simulink model "dynamical_model_extended"  (R2017b)
settings: Solver=ode4  StartTime=0.0  StopTime=3  FixedStep=dt  RelTol=1e-3
undefined symbols (not defined in the file or in its folder): alpha0, c1, c2, c3, d0, dq_0, g, m, p_true, q_0, r
libraries: dspinverses x2
(part 2 of 3)

== matlab function dynamical_model_extended/soft robotic manipulator dynamical model/Coreoilis matrix  ==
  data: q input; y output; dq input; m parameter; r parameter
function y = fcn(q,dq,m,r)

l1 = q(1);
kappa_x1 = q(2);
kappa_y1 = q(3);

dl1 = dq(1);
dkappa_x1 = dq(2);
dkappa_y1 = dq(3);

V = zeros(3,3);

% V(1,1) = (5.0e-33*dl1*m*(400000000000000000000000000000000.0*kappa_x1^2*sin(l1*(kappa_x1^2 + kappa_y1^2)^(1/2)) + 133333333333333333333333333333333.0*kappa_y1^2*l1^3*(kappa_x1^2 + kappa_y1^2)^(3/2) - 400000000000000000000000000000000.0*kappa_x1^2*l1*cos(l1*(kappa_x1^2 + kappa_y1^2)^(1/2))*(kappa_x1^2 + kappa_y1^2)^(1/2)))/(l1^2*(kappa_x1^2 + kappa_y1^2)^(5/2)) - (5.0e-33*dkappa_y1*kappa_y1*m*(266666666666666666666666666666677.0*kappa_y1^4*l1^3*(kappa_x1^2 + kappa_y1^2)^(3/2) - 133333333333333333333333333333333.0*kappa_x1^2*l1^3*(kappa_x1^2 + kappa_y1^2)^(5/2) - 266666666666666666666666666666677.0*kappa_y1^2*l1^3*(kappa_x1^2 + kappa_y1^2)^(5/2) - 2.0e33*kappa_x1^4*sin(l1*(kappa_x1^2 + kappa_y1^2)^(1/2)) - 2.0e33*kappa_x1^2*kappa_y1^2*sin(l1*(kappa_x1^2 + kappa_y1^2)^(1/2)) + 400000000000000000000000000000000.0*kappa_x1^2*l1*(kappa_x1^2 + kappa_y1^2)^(3/2) + 1.2e33*kappa_x1^4*l1*(kappa_x1^2 + kappa_y1^2)^(1/2) + 266666666666666666666666666666677.0*kappa_x1^2*kappa_y1^2*l1^3*(kappa_x1^2 + kappa_y1^2)^(3/2) + 400000000000000000000000000000000.0*kappa_x1^4*l1*cos(l1*(kappa_x1^2 + kappa_y1^2)^(1/2))*(kappa_x1^2 + kappa_y1^2)^(1/2) + 1.2e33*kappa_x1^2*kappa_y1^2*l1*(kappa_x1^2 + kappa_y1^2)^(1/2) + 400000000000000000000000000000000.0*kappa_x1^2*kappa_y1^2*l1*cos(l1*(kappa_x1^2 + kappa_y1^2)^(1/2))*(kappa_x1^2 + kappa_y1^2)^(1/2)))/(l1*(kappa_x1^2 + kappa_y1^2)^(9/2)) - (5.0e-33*dkappa_x1*kappa_x1*m*(800000000000000000000000000000000.0*kappa_y1^4*sin(l1*(kappa_x1^2 + kappa_y1^2)^(1/2)) - 1.2e33*kappa_x1^4*sin(l1*(kappa_x1^2 + kappa_y1^2)^(1/2)) - 400000000000000000000000000000000.0*l1*(kappa_x1^2 + kappa_y1^2)^(5/2) - 133333333333333333333333333333333.0*kappa_y1^2*l1^3*(kappa_x1^2 + kappa_y1^2)^(5/2) + 266666666666666666666666666666677.0*kappa_y1^4*l1^3*(kappa_x1^2 + kappa_y1^2)^(3/2) - 400000000000000000000000000000000.0*kappa_x1^2*kappa_y1^2*sin(l1*(kappa_x1^2 + kappa_y1^2)^(1/2)) + 1.2e33*kappa_x1^4*l1*(kappa_x1^2 + kappa_y1^2)^(1/2) - 400000000000000000000000000000000.0*kappa_y1^2*l1*(kappa_x1^2 + kappa_y1^2)^(3/2) + 266666666666666666666666666666677.0*kappa_x1^2*kappa_y1^2*l1^3*(kappa_x1^2 + kappa_y1^2)^(3/2) + 400000000000000000000000000000000.0*kappa_x1^4*l1*cos(l1*(kappa_x1^2 + kappa_y1^2)^(1/2))*(kappa_x1^2 + kappa_y1^2)^(1/2) + 1.2e33*kappa_x1^2*kappa_y1^2*l1*(kappa_x1^2 + kappa_y1^2)^(1/2) + 400000000000000000000000000000000.0*kappa_x1^2*kappa_y1^2*l1*cos(l1*(kappa_x1^2 + kappa_y1^2)^(1/2))*(kappa_x1^2 + kappa_y1^2)^(1/2)))/(l1*(kappa_x1^2 + kappa_y1^2)^(9/2));
% V(1,2) = - (dkappa_x1*(6.4e34*l1*m*(kappa_x1^2 + kappa_y1^2)^(3/2) - 1.6e34*l1^3*m*(kappa_x1^2 + kappa_y1^2)^(5/2) - 6.4e34*l1*m*cos(l1*(kappa_x1^2 + kappa_y1^2)^(1/2))*(kappa_x1^2 + kappa_y1^2)^(3/2) + 1.6e34*l1^2*m*sin(l1*(kappa_x1^2 + kappa_y1^2)^(1/2))*(kappa_x1^2 + kappa_y1^2)^2 + 3.2e34*kappa_x1^2*l1^3*m*(kappa_x1^2 + kappa_y1^2)^(3/2) + 3.2e34*kappa_y1^2*l1^3*m*(kappa_x1^2 + kappa_y1^2)^(3/2) + 5.3333333333333333333333333333333e33*kappa_x1^6*l1^3*m*((kappa_x1^2 + kappa_y1^2)/kappa_x1^2)^(1/2) + 1.6e34*kappa_x1^2*l1^3*m*cos(l1*(kappa_x1^2 + kappa_y1^2)^(1/2))*(kappa_x1^2 + kappa_y1^2)^(3/2) + 1.6e34*kappa_y1^2*l1^3*m*cos(l1*(kappa_x1^2 + kappa_y1^2)^(1/2))*(kappa_x1^2 + kappa_y1^2)^(3/2) - 2.0e33*kappa_y1^2*m*sin(2.0*l1*(kappa_x1^2 + kappa_y1^2)^(1/2))*((kappa_x1^2 + kappa_y1^2)/kappa_x1^2)^(1/2)*(kappa_x1^2 + kappa_y1^2)^(1/2) + 5.3333333333333333333333333333333e33*kappa_x1^2*kappa_y1^4*l1^3*m*((kappa_x1^2 + kappa_y1^2)/kappa_x1^2)^(1/2) + 1.0666666666666666666666666666667e34*kappa_x1^4*kappa_y1^2*l1^3*m*((kappa_x1^2 + kappa_y1^2)/kappa_x1^2)^(1/2) + 1.3333333333333333333333333333333e33*kappa_x1^8*l1^3*m*r^2*((kappa_x1^2 + kappa_y1^2)/kappa_x1^2)^(1/2) - 8.0e34*kappa_x1^2*l1^2*m*sin(l1*(kappa_x1^2 + kappa_y1^2)^(1/2))*(kappa_x1^2 + kappa_y1^2) - 8.0e34*kappa_y1^2*l1^2*m*sin(l1*(kappa_x1^2 + kappa_y1^2)^(1/2))*(kappa_x1^2 + kappa_y1^2) + 3.2e34*kappa_x1^2*m*sin(l1*(kappa_x1^2 + kappa_y1^2)^(1/2))*((kappa_x1^2 + kappa_y1^2)/kappa_x1^2)^(1/2)*(kappa_x1^2 + kappa_y1^2)^(1/2) + 1.6e34*kappa_y1^2*m*sin(l1*(kappa_x1^2 + kappa_y1^2)^(1/2))*((kappa_x1^2 + kappa_y1^2)/kappa_x1^2)^(1/2)*(kappa_x1^2 + kappa_y1^2)^(1/2) - 1.0e33*kappa_y1^2*m*r^2*sin(2.0*l1*(kappa_x1^2 + kappa_y1^2)^(1/2))*((kappa_x1^2 + kappa_y1^2)/kappa_x1^2)^(1/2)*(kappa_x1^2 + kappa_y1^2)^(3/2) + 500000000000000000000000000000000.0*kappa_y1^4*m*r^2*sin(2.0*l1*(kappa_x1^2 + kappa_y1^2)^(1/2))*((kappa_x1^2 + kappa_y1^2)/kappa_x1^2)^(1/2)*(kappa_x1^2 + kappa_y1^2)^(1/2) + 4.0e33*kappa_y1^2*l1*m*cos(2.0*l1*(kappa_x1^2 + kappa_y1^2)^(1/2))*((kappa_x1^2 + kappa_y1^2)/kappa_x1^2)^(1/2)*(kappa_x1^2 + kappa_y1^2) + 2.6666666666666666666666666666667e33*kappa_x1^2*kappa_y1^6*l1^3*m*r^2*((kappa_x1^2 + kappa_y1^2)/kappa_x1^2)^(1/2) + 6.6666666666666666666666666666667e33*kappa_x1^4*kappa_y1^4*l1^3*m*r^2*((kappa_x1^2 + kappa_y1^2)/kappa_x1^2)^(1/2) + 5.3333333333333333333333333333333e33*kappa_x1^6*kappa_y1^2*l1^3*m*r^2*((kappa_x1^2 + kappa_y1^2)/kappa_x1^2)^(1/2) - 1.6e34*kappa_x1^4*l1^2*m*sin(l1*(kappa_x1^2 + kappa_y1^2)^(1/2))*((kappa_x1^2 + kappa_y1^2)/kappa_x1^2)^(1/2)*(kappa_x1^2 + kappa_y1^2)^(1/2) + 8.0e33*kappa_y1^2*m*r^2*sin(l1*(kappa_x1^2 + kappa_y1^2)^(1/2))*((kappa_x1^2 + kappa_y1^2)/kappa_x1^2)^(1/2)*(kappa_x1^2 + kappa_y1^2)^(3/2) - 3.2e34*kappa_x1^2*l1*m*cos(l1*(kappa_x1^2 + kappa_y1^2)^(1/2))*((kappa_x1^2 + kappa_y1^2)/kappa_x1^2)^(1/2)*(kappa_x1^2 + kappa_y1^2) - 1.6e34*kappa_y1^2*l1*m*cos(l1*(kappa_x1^2 + kappa_y1^2)^(1/2))*((kappa_x1^2 + kappa_y1^2)/kappa_x1^2)^(1/2)*(kappa_x1^2 + kappa_y1^2) - 1.0e33*kappa_y1^4*l1*m*r^2*cos(2.0*l1*(kappa_x1^2 + kappa_y1^2)^(1/2))*((kappa_x1^2 + kappa_y1^2)/kappa_x1^2)^(1/2)*(kappa_x1^2 + kappa_y1^2) - 8.0e33*kappa_y1^2*l1*m*r^2*cos(l1*(kappa_x1^2 + kappa_y1^2)^(1/2))*((kappa_x1^2 + kappa_y1^2)/kappa_x1^2)^(1/2)*(kappa_x1^2 + kappa_y1^2)^2 + 2.0e33*kappa_y1^2*l1*m*r^2*cos(2.0*l1*(kappa_x1^2 + kappa_y1^2)^(1/2))*((kappa_x1^2 + kappa_y1^2)/kappa_x1^2)^(1/2)*(kappa_x1^2 + kappa_y1^2)^2 - 1.6e34*kappa_x1^2*kappa_y1^2*l1^2*m*sin(l1*(kappa_x1^2 + kappa_y1^2)^(1/2))*((kappa_x1^2 + kappa_y1^2)/kappa_x1^2)^(1/2)*(kappa_x1^2 + kappa_y1^2)^(1/2) + 4.0e33*kappa_x1^2*kappa_y1^2*m*r^2*sin(l1*(kappa_x1^2 + kappa_y1^2)^(1/2))*((kappa_x1^2 + kappa_y1^2)/kappa_x1^2)^(1/2)*(kappa_x1^2 + kappa_y1^2)^(1/2) + 1.0e33*kappa_x1^2*kappa_y1^2*m*r^2*sin(2.0*l1*(kappa_x1^2 + kappa_y1^2)^(1/2))*((kappa_x1^2 + kappa_y1^2)/kappa_x1^2)^(1/2)*(kappa_x1^2 + kappa_y1^2)^(1/2) - 4.0e33*kappa_x1^2*kappa_y1^4*l1^2*m*r^2*sin(l1*(kappa_x1^2 + kappa_y1^2)^(1/2))*((kappa_x1^2 + kappa_y1^2)/kappa_x1^2)^(1/2)*(kappa_x1^2 + kappa_y1^2)^(1/2) - 4.0e33*kappa_x1^4*kappa_y1^2*l1^2*m*r^2*sin(l1*(kappa_x1^2 + kappa_y1^2)^(1/2))*((kappa_x1^2 + kappa_y1^2)/kappa_x1^2)^(1/2)*(kappa_x1^2 + kappa_y1^2)^(1/2) - 4.0e33*kappa_x1^2*kappa_y1^2*l1*m*r^2*cos(l1*(kappa_x1^2 + kappa_y1^2)^(1/2))*((kappa_x1^2 + kappa_y1^2)/kappa_x1^2)^(1/2)*(kappa_x1^2 + kappa_y1^2) - 2.0e33*kappa_x1^2*kappa_y1^2*l1*m*r^2*cos(2.0*l1*(kappa_x1^2 + kappa_y1^2)^(1/2))*((kappa_x1^2 + kappa_y1^2)/kappa_x1^2)^(1/2)*(kappa_x1^2 + kappa_y1^2)))/(8000000000000000000000000000000000*l1^2*((kappa_x1^2 + kappa_y1^2)/kappa_x1^2)^(1/2)*(kappa_x1^2 + kappa_y1^2)^4) - (dkappa_y1*(4.0e33*kappa_y1^3*l1^3*m*(kappa_x1^2 + kappa_y1^2)^(3/2) - 2.0e33*kappa_y1*l1^3*m*(kappa_x1^2 + kappa_y1^2)^(5/2) + 8.0e33*kappa_y1*l1*m*(kappa_x1^2 + kappa_y1^2)^(3/2) + 4.0e33*kappa_x1^2*kappa_y1*l1^3*m*(kappa_x1^2 + kappa_y1^2)^(3/2) + 2.0e33*kappa_y1^3*l1^3*m*cos(l1*(kappa_x1^2 + kappa_y1^2)^(1/2))*(kappa_x1^2 + kappa_y1^2)^(3/2) + 1.3333333333333333333333333333333e33*kappa_x1^6*kappa_y1*l1^3*m*((kappa_x1^2 + kappa_y1^2)/kappa_x1^2)^(1/2) - 8.0e33*kappa_y1*l1*m*cos(l1*(kappa_x1^2 + kappa_y1^2)^(1/2))*(kappa_x1^2 + kappa_y1^2)^(3/2) + 1.3333333333333333333333333333333e33*kappa_x1^2*kappa_y1^5*l1^3*m*((kappa_x1^2 + kappa_y1^2)/kappa_x1^2)^(1/2) + 2.6666666666666666666666666666667e33*kappa_x1^4*kappa_y1^3*l1^3*m*((kappa_x1^2 + kappa_y1^2)/kappa_x1^2)^(1/2) + 2.0e33*kappa_y1*l1^2*m*sin(l1*(kappa_x1^2 + kappa_y1^2)^(1/2))*(kappa_x1^2 + kappa_y1^2)^2 - 1.0e34*kappa_y1^3*l1^2*m*sin(l1*(kappa_x1^2 + kappa_y1^2)^(1/2))*(kappa_x1^2 + kappa_y1^2) + 333333333333333333333333333333333.0*kappa_x1^8*kappa_y1*l1^3*m*r^2*((kappa_x1^2 + kappa_y1^2)/kappa_x1^2)^(1/2) - 1.0e34*kappa_x1^2*kappa_y1*l1^2*m*sin(l1*(kappa_x1^2 + kappa_y1^2)^(1/2))*(kappa_x1^2 + kappa_y1^2) + 4.0e33*kappa_x1^2*kappa_y1*m*sin(l1*(kappa_x1^2 + kappa_y1^2)^(1/2))*((kappa_x1^2 + kappa_y1^2)/kappa_x1^2)^(1/2)*(kappa_x1^2 + kappa_y1^2)^(1/2) + 666666666666666666666666666666677.0*kappa_x1^2*kappa_y1^7*l1^3*m*r^2*((kappa_x1^2 + kappa_y1^2)/kappa_x1^2)^(1/2) + 1.6666666666666666666666666666667e33*kappa_x1^4*kappa_y1^5*l1^3*m*r^2*((kappa_x1^2 + kappa_y1^2)/kappa_x1^2)^(1/2) + 1.3333333333333333333333333333333e33*kappa_x1^6*kappa_y1^3*l1^3*m*r^2*((kappa_x1^2 + kappa_y1^2)/kappa_x1^2)^(1/2) + 2.0e33*kappa_x1^2*kappa_y1*l1^3*m*cos(l1*(kappa_x1^2 + kappa_y1^2)^(1/2))*(kappa_x1^2 + kappa_y1^2)^(3/2) + 500000000000000000000000000000000.0*kappa_x1^2*kappa_y1*m*sin(2.0*l1*(kappa_x1^2 + kappa_y1^2)^(1/2))*((kappa_x1^2 + kappa_y1^2)/kappa_x1^2)^(1/2)*(kappa_x1^2 + kappa_y1^2)^(1/2) - 4.0e33*kappa_x1^4*kappa_y1*l1^2*m*sin(l1*(kappa_x1^2 + kappa_y1^2)^(1/2))*((kappa_x1^2 + kappa_y1^2)/kappa_x1^2)^(1/2)*(kappa_x1^2 + kappa_y1^2)^(1/2) - 2.0e33*kappa_x1^2*kappa_y1*m*r^2*sin(l1*(kappa_x1^2 + kappa_y1^2)^(1/2))*((kappa_x1^2 + kappa_y1^2)/kappa_x1^2)^(1/2)*(kappa_x1^2 + kappa_y1^2)^(3/2) - 500000000000000000000000000000000.0*kappa_x1^4*kappa_y1*m*r^2*sin(l1*(kappa_x1^2 + kappa_y1^2)^(1/2))*((kappa_x1^2 + kappa_y1^2)/kappa_x1^2)^(1/2)*(kappa_x1^2 + kappa_y1^2)^(1/2) - 4.0e33*kappa_x1^2*kappa_y1*l1*m*cos(l1*(kappa_x1^2 + kappa_y1^2)^(1/2))*((kappa_x1^2 + kappa_y1^2)/kappa_x1^2)^(1/2)*(kappa_x1^2 + kappa_y1^2) + 250000000000000000000000000000000.0*kappa_x1^2*kappa_y1*m*r^2*sin(2.0*l1*(kappa_x1^2 + kappa_y1^2)^(1/2))*((kappa_x1^2 + kappa_y1^2)/kappa_x1^2)^(1/2)*(kappa_x1^2 + kappa_y1^2)^(3/2) - 250000000000000000000000000000000.0*kappa_x1^4*kappa_y1*m*r^2*sin(2.0*l1*(kappa_x1^2 + kappa_y1^2)^(1/2))*((kappa_x1^2 + kappa_y1^2)/kappa_x1^2)^(1/2)*(kappa_x1^2 + kappa_y1^2)^(1/2) - 4.0e33*kappa_x1^2*kappa_y1^3*l1^2*m*sin(l1*(kappa_x1^2 + kappa_y1^2)^(1/2))*((kappa_x1^2 + kappa_y1^2)/kappa_x1^2)^(1/2)*(kappa_x1^2 + kappa_y1^2)^(1/2) + 500000000000000000000000000000000.0*kappa_x1^2*kappa_y1^3*m*r^2*sin(l1*(kappa_x1^2 + kappa_y1^2)^(1/2))*((kappa_x1^2 + kappa_y1^2)/kappa_x1^2)^(1/2)*(kappa_x1^2 + kappa_y1^2)^(1/2) - 1.0e33*kappa_x1^2*kappa_y1*l1*m*cos(2.0*l1*(kappa_x1^2 + kappa_y1^2)^(1/2))*((kappa_x1^2 + kappa_y1^2)/kappa_x1^2)^(1/2)*(kappa_x1^2 + kappa_y1^2) - 125000000000000000000000000000000.0*kappa_x1^2*kappa_y1^3*m*r^2*sin(2.0*l1*(kappa_x1^2 + kappa_y1^2)^(1/2))*((kappa_x1^2 + kappa_y1^2)/kappa_x1^2)^(1/2)*(kappa_x1^2 + kappa_y1^2)^(1/2) + 500000000000000000000000000000000.0*kappa_x1^6*kappa_y1*l1^2*m*r^2*sin(l1*(kappa_x1^2 + kappa_y1^2)^(1/2))*((kappa_x1^2 + kappa_y1^2)/kappa_x1^2)^(1/2)*(kappa_x1^2 + kappa_y1^2)^(1/2) + 500000000000000000000000000000000.0*kappa_x1^4*kappa_y1*l1*m*r^2*cos(l1*(kappa_x1^2 + kappa_y1^2)^(1/2))*((kappa_x1^2 + kappa_y1^2)/kappa_x1^2)^(1/2)*(kappa_x1^2 + kappa_y1^2) - 500000000000000000000000000000000.0*kappa_x1^2*kappa_y1^5*l1^2*m*r^2*sin(l1*(kappa_x1^2 + kappa_y1^2)^(1/2))*((kappa_x1^2 + kappa_y1^2)/kappa_x1^2)^(1/2)*(kappa_x1^2 + kappa_y1^2)^(1/2) + 500000000000000000000000000000000.0*kappa_x1^4*kappa_y1*l1*m*r^2*cos(2.0*l1*(kappa_x1^2 + kappa_y1^2)^(1/2))*((kappa_x1^2 + kappa_y1^2)/kappa_x1^2)^(1/2)*(kappa_x1^2 + kappa_y1^2) + 2.0e33*kappa_x1^2*kappa_y1*l1*m*r^2*cos(l1*(kappa_x1^2 + kappa_y1^2)^(1/2))*((kappa_x1^2 + kappa_y1^2)/kappa_x1^2)^(1/2)*(kappa_x1^2 + kappa_y1^2)^2 - 500000000000000000000000000000000.0*kappa_x1^2*kappa_y1^3*l1*m*r^2*cos(l1*(kappa_x1^2 + kappa_y1^2)^(1/2))*((kappa_x1^2 + kappa_y1^2)/kappa_x1^2)^(1/2)*(kappa_x1^2 + kappa_y1^2) - 500000000000000000000000000000000.0*kappa_x1^2*kappa_y1*l1*m*r^2*cos(2.0*l1*(kappa_x1^2 + kappa_y1^2)^(1/2))*((kappa_x1^2 + kappa_y1^2)/kappa_x1^2)^(1/2)*(kappa_x1^2 + kappa_y1^2)^2 + 250000000000000000000000000000000.0*kappa_x1^2*kappa_y1^3*l1*m*r^2*cos(2.0*l1*(kappa_x1^2 + kappa_y1^2)^(1/2))*((kappa_x1^2 + kappa_y1^2)/kappa_x1^2)^(1/2)*(kappa_x1^2 + kappa_y1^2)))/(2000000000000000000000000000000000*kappa_x1*l1^2*((kappa_x1^2 + kappa_y1^2)/kappa_x1^2)^(1/2)*(kappa_x1^2 + kappa_y1^2)^4) - (5.0e-33*dl1*kappa_x1*m*(800000000000000000000000000000000.0*kappa_y1^4*sin(l1*(kappa_x1^2 + kappa_y1^2)^(1/2)) - 1.2e33*kappa_x1^4*sin(l1*(kappa_x1^2 + kappa_y1^2)^(1/2)) - 400000000000000000000000000000000.0*l1*(kappa_x1^2 + kappa_y1^2)^(5/2) - 133333333333333333333333333333333.0*kappa_y1^2*l1^3*(kappa_x1^2 + kappa_y1^2)^(5/2) + 266666666666666666666666666666677.0*kappa_y1^4*l1^3*(kappa_x1^2 + kappa_y1^2)^(3/2) - 400000000000000000000000000000000.0*kappa_x1^2*kappa_y1^2*sin(l1*(kappa_x1^2 + kappa_y1^2)^(1/2)) + 1.2e33*kappa_x1^4*l1*(kappa_x1^2 + kappa_y1^2)^(1/2) - 400000000000000000000000000000000.0*kappa_y1^2*l1*(kappa_x1^2 + kappa_y1^2)^(3/2) + 266666666666666666666666666666677.0*kappa_x1^2*kappa_y1^2*l1^3*(kappa_x1^2 + kappa_y1^2)^(3/2) + 400000000000000000000000000000000.0*kappa_x1^4*l1*cos(l1*(kappa_x1^2 + kappa_y1^2)^(1/2))*(kappa_x1^2 + kappa_y1^2)^(1/2) + 1.2e33*kappa_x1^2*kappa_y1^2*l1*(kappa_x1^2 + kappa_y1^2)^(1/2) + 400000000000000000000000000000000.0*kappa_x1^2*kappa_y1^2*l1*cos(l1*(kappa_x1^2 + kappa_y1^2)^(1/2))*(kappa_x1^2 + kappa_y1^2)^(1/2)))/(l1*(kappa_x1^2 + kappa_y1^2)^(9/2));
% V(1,3) = - (dkappa_y1*(5.3333333333333333333333333333333e33*kappa_y1^6*l1^3*m + 1.0666666666666666666666666666667e34*kappa_x1^2*kappa_y1^4*l1^3*m + 5.3333333333333333333333333333333e33*kappa_x1^4*kappa_y1^2*l1^3*m + 2.6666666666666666666666666666667e33*kappa_y1^8*l1^3*m*r^2 + 1.6e34*kappa_x1^2*m*sin(l1*(kappa_x1^2 + kappa_y1^2)^(1/2))*(kappa_x1^2 + kappa_y1^2)^(1/2) + 3.2e34*kappa_y1^2*m*sin(l1*(kappa_x1^2 + kappa_y1^2)^(1/2))*(kappa_x1^2 + kappa_y1^2)^(1/2) - 2.0e33*kappa_x1^2*m*sin(2.0*l1*(kappa_x1^2 + kappa_y1^2)^(1/2))*(kappa_x1^2 + kappa_y1^2)^(1/2) - 1.6e34*kappa_y1^4*l1^2*m*sin(l1*(kappa_x1^2 + kappa_y1^2)^(1/2))*(kappa_x1^2 + kappa_y1^2)^(1/2) + 8.0e33*kappa_x1^2*m*r^2*sin(l1*(kappa_x1^2 + kappa_y1^2)^(1/2))*(kappa_x1^2 + kappa_y1^2)^(3/2) - 1.6e34*kappa_x1^2*l1*m*cos(l1*(kappa_x1^2 + kappa_y1^2)^(1/2))*(kappa_x1^2 + kappa_y1^2) - 3.2e34*kappa_y1^2*l1*m*cos(l1*(kappa_x1^2 + kappa_y1^2)^(1/2))*(kappa_x1^2 + kappa_y1^2) - 1.0e33*kappa_x1^2*m*r^2*sin(2.0*l1*(kappa_x1^2 + kappa_y1^2)^(1/2))*(kappa_x1^2 + kappa_y1^2)^(3/2) + 1.0e33*kappa_x1^4*m*r^2*sin(2.0*l1*(kappa_x1^2 + kappa_y1^2)^(1/2))*(kappa_x1^2 + kappa_y1^2)^(1/2) + 4.0e33*kappa_x1^2*l1*m*cos(2.0*l1*(kappa_x1^2 + kappa_y1^2)^(1/2))*(kappa_x1^2 + kappa_y1^2) + 6.6666666666666666666666666666667e33*kappa_x1^2*kappa_y1^6*l1^3*m*r^2 + 5.3333333333333333333333333333333e33*kappa_x1^4*kappa_y1^4*l1^3*m*r^2 + 1.3333333333333333333333333333333e33*kappa_x1^6*kappa_y1^2*l1^3*m*r^2 - 1.6e34*kappa_x1^2*kappa_y1^2*l1^2*m*sin(l1*(kappa_x1^2 + kappa_y1^2)^(1/2))*(kappa_x1^2 + kappa_y1^2)^(1/2) - 4.0e33*kappa_x1^2*kappa_y1^2*m*r^2*sin(l1*(kappa_x1^2 + kappa_y1^2)^(1/2))*(kappa_x1^2 + kappa_y1^2)^(1/2) + 500000000000000000000000000000000.0*kappa_x1^2*kappa_y1^2*m*r^2*sin(2.0*l1*(kappa_x1^2 + kappa_y1^2)^(1/2))*(kappa_x1^2 + kappa_y1^2)^(1/2) - 2.0e33*kappa_x1^4*l1*m*r^2*cos(2.0*l1*(kappa_x1^2 + kappa_y1^2)^(1/2))*(kappa_x1^2 + kappa_y1^2) - 8.0e33*kappa_x1^2*l1*m*r^2*cos(l1*(kappa_x1^2 + kappa_y1^2)^(1/2))*(kappa_x1^2 + kappa_y1^2)^2 + 2.0e33*kappa_x1^2*l1*m*r^2*cos(2.0*l1*(kappa_x1^2 + kappa_y1^2)^(1/2))*(kappa_x1^2 + kappa_y1^2)^2 + 4.0e33*kappa_x1^2*kappa_y1^2*l1*m*r^2*cos(l1*(kappa_x1^2 + kappa_y1^2)^(1/2))*(kappa_x1^2 + kappa_y1^2) - 1.0e33*kappa_x1^2*kappa_y1^2*l1*m*r^2*cos(2.0*l1*(kappa_x1^2 + kappa_y1^2)^(1/2))*(kappa_x1^2 + kappa_y1^2) + 4.0e33*kappa_x1^2*kappa_y1^4*l1^2*m*r^2*sin(l1*(kappa_x1^2 + kappa_y1^2)^(1/2))*(kappa_x1^2 + kappa_y1^2)^(1/2) + 4.0e33*kappa_x1^4*kappa_y1^2*l1^2*m*r^2*sin(l1*(kappa_x1^2 + kappa_y1^2)^(1/2))*(kappa_x1^2 + kappa_y1^2)^(1/2)))/(8000000000000000000000000000000000*l1^2*(kappa_x1^2 + kappa_y1^2)^4) - (5.0e-33*dl1*kappa_y1*m*(266666666666666666666666666666677.0*kappa_y1^4*l1^3*(kappa_x1^2 + kappa_y1^2)^(3/2) - 133333333333333333333333333333333.0*kappa_x1^2*l1^3*(kappa_x1^2 + kappa_y1^2)^(5/2) - 266666666666666666666666666666677.0*kappa_y1^2*l1^3*(kappa_x1^2 + kappa_y1^2)^(5/2) - 2.0e33*kappa_x1^4*sin(l1*(kappa_x1^2 + kappa_y1^2)^(1/2)) - 2.0e33*kappa_x1^2*kappa_y1^2*sin(l1*(kappa_x1^2 + kappa_y1^2)^(1/2)) + 400000000000000000000000000000000.0*kappa_x1^2*l1*(kappa_x1^2 + kappa_y1^2)^(3/2) + 1.2e33*kappa_x1^4*l1*(kappa_x1^2 + kappa_y1^2)^(1/2) + 266666666666666666666666666666677.0*kappa_x1^2*kappa_y1^2*l1^3*(kappa_x1^2 + kappa_y1^2)^(3/2) + 400000000000000000000000000000000.0*kappa_x1^4*l1*cos(l1*(kappa_x1^2 + kappa_y1^2)^(1/2))*(kappa_x1^2 + kappa_y1^2)^(1/2) + 1.2e33*kappa_x1^2*kappa_y1^2*l1*(kappa_x1^2 + kappa_y1^2)^(1/2) + 400000000000000000000000000000000.0*kappa_x1^2*kappa_y1^2*l1*cos(l1*(kappa_x1^2 + kappa_y1^2)^(1/2))*(kappa_x1^2 + kappa_y1^2)^(1/2)))/(l1*(kappa_x1^2 + kappa_y1^2)^(9/2)) - (dkappa_x1*(4.0e33*kappa_y1^3*l1^3*m*(kappa_x1^2 + kappa_y1^2)^(3/2) - 2.0e33*kappa_y1*l1^3*m*(kappa_x1^2 + kappa_y1^2)^(5/2) + 8.0e33*kappa_y1*l1*m*(kappa_x1^2 + kappa_y1^2)^(3/2) + 4.0e33*kappa_x1^2*kappa_y1*l1^3*m*(kappa_x1^2 + kappa_y1^2)^(3/2) + 2.0e33*kappa_y1^3*l1^3*m*cos(l1*(kappa_x1^2 + kappa_y1^2)^(1/2))*(kappa_x1^2 + kappa_y1^2)^(3/2) + 1.3333333333333333333333333333333e33*kappa_x1^6*kappa_y1*l1^3*m*((kappa_x1^2 + kappa_y1^2)/kappa_x1^2)^(1/2) - 8.0e33*kappa_y1*l1*m*cos(l1*(kappa_x1^2 + kappa_y1^2)^(1/2))*(kappa_x1^2 + kappa_y1^2)^(3/2) + 1.3333333333333333333333333333333e33*kappa_x1^2*kappa_y1^5*l1^3*m*((kappa_x1^2 + kappa_y1^2)/kappa_x1^2)^(1/2) + 2.6666666666666666666666666666667e33*kappa_x1^4*kappa_y1^3*l1^3*m*((kappa_x1^2 + kappa_y1^2)/kappa_x1^2)^(1/2) + 2.0e33*kappa_y1*l1^2*m*sin(l1*(kappa_x1^2 + kappa_y1^2)^(1/2))*(kappa_x1^2 + kappa_y1^2)^2 - 1.0e34*kappa_y1^3*l1^2*m*sin(l1*(kappa_x1^2 + kappa_y1^2)^(1/2))*(kappa_x1^2 + kappa_y1^2) + 333333333333333333333333333333333.0*kappa_x1^8*kappa_y1*l1^3*m*r^2*((kappa_x1^2 + kappa_y1^2)/kappa_x1^2)^(1/2) - 1.0e34*kappa_x1^2*kappa_y1*l1^2*m*sin(l1*(kappa_x1^2 + kappa_y1^2)^(1/2))*(kappa_x1^2 + kappa_y1^2) + 4.0e33*kappa_x1^2*kappa_y1*m*sin(l1*(kappa_x1^2 + kappa_y1^2)^(1/2))*((kappa_x1^2 + kappa_y1^2)/kappa_x1^2)^(1/2)*(kappa_x1^2 + kappa_y1^2)^(1/2) + 666666666666666666666666666666677.0*kappa_x1^2*kappa_y1^7*l1^3*m*r^2*((kappa_x1^2 + kappa_y1^2)/kappa_x1^2)^(1/2) + 1.6666666666666666666666666666667e33*kappa_x1^4*kappa_y1^5*l1^3*m*r^2*((kappa_x1^2 + kappa_y1^2)/kappa_x1^2)^(1/2) + 1.3333333333333333333333333333333e33*kappa_x1^6*kappa_y1^3*l1^3*m*r^2*((kappa_x1^2 + kappa_y1^2)/kappa_x1^2)^(1/2) + 2.0e33*kappa_x1^2*kappa_y1*l1^3*m*cos(l1*(kappa_x1^2 + kappa_y1^2)^(1/2))*(kappa_x1^2 + kappa_y1^2)^(3/2) + 500000000000000000000000000000000.0*kappa_x1^2*kappa_y1*m*sin(2.0*l1*(kappa_x1^2 + kappa_y1^2)^(1/2))*((kappa_x1^2 + kappa_y1^2)/kappa_x1^2)^(1/2)*(kappa_x1^2 + kappa_y1^2)^(1/2) - 4.0e33*kappa_x1^4*kappa_y1*l1^2*m*sin(l1*(kappa_x1^2 + kappa_y1^2)^(1/2))*((kappa_x1^2 + kappa_y1^2)/kappa_x1^2)^(1/2)*(kappa_x1^2 + kappa_y1^2)^(1/2) - 2.0e33*kappa_x1^2*kappa_y1*m*r^2*sin(l1*(kappa_x1^2 + kappa_y1^2)^(1/2))*((kappa_x1^2 + kappa_y1^2)/kappa_x1^2)^(1/2)*(kappa_x1^2 + kappa_y1^2)^(3/2) - 500000000000000000000000000000000.0*kappa_x1^4*kappa_y1*m*r^2*sin(l1*(kappa_x1^2 + kappa_y1^2)^(1/2))*((kappa_x1^2 + kappa_y1^2)/kappa_x1^2)^(1/2)*(kappa_x1^2 + kappa_y1^2)^(1/2) - 4.0e33*kappa_x1^2*kappa_y1*l1*m*cos(l1*(kappa_x1^2 + kappa_y1^2)^(1/2))*((kappa_x1^2 + kappa_y1^2)/kappa_x1^2)^(1/2)*(kappa_x1^2 + kappa_y1^2) + 250000000000000000000000000000000.0*kappa_x1^2*kappa_y1*m*r^2*sin(2.0*l1*(kappa_x1^2 + kappa_y1^2)^(1/2))*((kappa_x1^2 + kappa_y1^2)/kappa_x1^2)^(1/2)*(kappa_x1^2 + kappa_y1^2)^(3/2) - 250000000000000000000000000000000.0*kappa_x1^4*kappa_y1*m*r^2*sin(2.0*l1*(kappa_x1^2 + kappa_y1^2)^(1/2))*((kappa_x1^2 + kappa_y1^2)/kappa_x1^2)^(1/2)*(kappa_x1^2 + kappa_y1^2)^(1/2) - 4.0e33*kappa_x1^2*kappa_y1^3*l1^2*m*sin(l1*(kappa_x1^2 + kappa_y1^2)^(1/2))*((kappa_x1^2 + kappa_y1^2)/kappa_x1^2)^(1/2)*(kappa_x1^2 + kappa_y1^2)^(1/2) + 500000000000000000000000000000000.0*kappa_x1^2*kappa_y1^3*m*r^2*sin(l1*(kappa_x1^2 + kappa_y1^2)^(1/2))*((kappa_x1^2 + kappa_y1^2)/kappa_x1^2)^(1/2)*(kappa_x1^2 + kappa_y1^2)^(1/2) - 1.0e33*kappa_x1^2*kappa_y1*l1*m*cos(2.0*l1*(kappa_x1^2 + kappa_y1^2)^(1/2))*((kappa_x1^2 + kappa_y1^2)/kappa_x1^2)^(1/2)*(kappa_x1^2 + kappa_y1^2) - 125000000000000000000000000000000.0*kappa_x1^2*kappa_y1^3*m*r^2*sin(2.0*l1*(kappa_x1^2 + kappa_y1^2)^(1/2))*((kappa_x1^2 + kappa_y1^2)/kappa_x1^2)^(1/2)*(kappa_x1^2 + kappa_y1^2)^(1/2) + 500000000000000000000000000000000.0*kappa_x1^6*kappa_y1*l1^2*m*r^2*sin(l1*(kappa_x1^2 + kappa_y1^2)^(1/2))*((kappa_x1^2 + kappa_y1^2)/kappa_x1^2)^(1/2)*(kappa_x1^2 + kappa_y1^2)^(1/2) + 500000000000000000000000000000000.0*kappa_x1^4*kappa_y1*l1*m*r^2*cos(l1*(kappa_x1^2 + kappa_y1^2)^(1/2))*((kappa_x1^2 + kappa_y1^2)/kappa_x1^2)^(1/2)*(kappa_x1^2 + kappa_y1^2) - 500000000000000000000000000000000.0*kappa_x1^2*kappa_y1^5*l1^2*m*r^2*sin(l1*(kappa_x1^2 + kappa_y1^2)^(1/2))*((kappa_x1^2 + kappa_y1^2)/kappa_x1^2)^(1/2)*(kappa_x1^2 + kappa_y1^2)^(1/2) + 500000000000000000000000000000000.0*kappa_x1^4*kappa_y1*l1*m*r^2*cos(2.0*l1*(kappa_x1^2 + kappa_y1^2)^(1/2))*((kappa_x1^2 + kappa_y1^2)/kappa_x1^2)^(1/2)*(kappa_x1^2 + kappa_y1^2) + 2.0e33*kappa_x1^2*kappa_y1*l1*m*r^2*cos(l1*(kappa_x1^2 + kappa_y1^2)^(1/2))*((kappa_x1^2 + kappa_y1^2)/kappa_x1^2)^(1/2)*(kappa_x1^2 + kappa_y1^2)^2 - 500000000000000000000000000000000.0*kappa_x1^2*kappa_y1^3*l1*m*r^2*cos(l1*(kappa_x1^2 + kappa_y1^2)^(1/2))*((kappa_x1^2 + kappa_y1^2)/kappa_x1^2)^(1/2)*(kappa_x1^2 + kappa_y1^2) - 500000000000000000000000000000000.0*kappa_x1^2*kappa_y1*l1*m*r^2*cos(2.0*l1*(kappa_x1^2 + kappa_y1^2)^(1/2))*((kappa_x1^2 + kappa_y1^2)/kappa_x1^2)^(1/2)*(kappa_x1^2 + kappa_y1^2)^2 + 250000000000000000000000000000000.0*kappa_x1^2*kappa_y1^3*l1*m*r^2*cos(2.0*l1*(kappa_x1^2 + kappa_y1^2)^(1/2))*((kappa_x1^2 + kappa_y1^2)/kappa_x1^2)^(1/2)*(kappa_x1^2 + kappa_y1^2)))/(2000000000000000000000000000000000*kappa_x1*l1^2*((kappa_x1^2 + kappa_y1^2)/kappa_x1^2)^(1/2)*(kappa_x1^2 + kappa_y1^2)^4);
% 
% V(2,1) = (dkappa_x1*(5.3333333333333333333333333333333e33*kappa_x1^6*l1^3*m + 5.3333333333333333333333333333333e33*kappa_x1^2*kappa_y1^4*l1^3*m + 1.0666666666666666666666666666667e34*kappa_x1^4*kappa_y1^2*l1^3*m + 1.3333333333333333333333333333333e33*kappa_x1^8*l1^3*m*r^2 + 3.2e34*kappa_x1^2*m*sin(l1*(kappa_x1^2 + kappa_y1^2)^(1/2))*(kappa_x1^2 + kappa_y1^2)^(1/2) + 1.6e34*kappa_y1^2*m*sin(l1*(kappa_x1^2 + kappa_y1^2)^(1/2))*(kappa_x1^2 + kappa_y1^2)^(1/2) - 2.0e33*kappa_y1^2*m*sin(2.0*l1*(kappa_x1^2 + kappa_y1^2)^(1/2))*(kappa_x1^2 + kappa_y1^2)^(1/2) - 1.6e34*kappa_x1^4*l1^2*m*sin(l1*(kappa_x1^2 + kappa_y1^2)^(1/2))*(kappa_x1^2 + kappa_y1^2)^(1/2) + 8.0e33*kappa_y1^2*m*r^2*sin(l1*(kappa_x1^2 + kappa_y1^2)^(1/2))*(kappa_x1^2 + kappa_y1^2)^(3/2) - 3.2e34*kappa_x1^2*l1*m*cos(l1*(kappa_x1^2 + kappa_y1^2)^(1/2))*(kappa_x1^2 + kappa_y1^2) - 1.6e34*kappa_y1^2*l1*m*cos(l1*(kappa_x1^2 + kappa_y1^2)^(1/2))*(kappa_x1^2 + kappa_y1^2) - 1.0e33*kappa_y1^2*m*r^2*sin(2.0*l1*(kappa_x1^2 + kappa_y1^2)^(1/2))*(kappa_x1^2 + kappa_y1^2)^(3/2) + 500000000000000000000000000000000.0*kappa_y1^4*m*r^2*sin(2.0*l1*(kappa_x1^2 + kappa_y1^2)^(1/2))*(kappa_x1^2 + kappa_y1^2)^(1/2) + 4.0e33*kappa_y1^2*l1*m*cos(2.0*l1*(kappa_x1^2 + kappa_y1^2)^(1/2))*(kappa_x1^2 + kappa_y1^2) + 2.6666666666666666666666666666667e33*kappa_x1^2*kappa_y1^6*l1^3*m*r^2 + 6.6666666666666666666666666666667e33*kappa_x1^4*kappa_y1^4*l1^3*m*r^2 + 5.3333333333333333333333333333333e33*kappa_x1^6*kappa_y1^2*l1^3*m*r^2 - 1.6e34*kappa_x1^2*kappa_y1^2*l1^2*m*sin(l1*(kappa_x1^2 + kappa_y1^2)^(1/2))*(kappa_x1^2 + kappa_y1^2)^(1/2) + 4.0e33*kappa_x1^2*kappa_y1^2*m*r^2*sin(l1*(kappa_x1^2 + kappa_y1^2)^(1/2))*(kappa_x1^2 + kappa_y1^2)^(1/2) + 1.0e33*kappa_x1^2*kappa_y1^2*m*r^2*sin(2.0*l1*(kappa_x1^2 + kappa_y1^2)^(1/2))*(kappa_x1^2 + kappa_y1^2)^(1/2) - 1.0e33*kappa_y1^4*l1*m*r^2*cos(2.0*l1*(kappa_x1^2 + kappa_y1^2)^(1/2))*(kappa_x1^2 + kappa_y1^2) - 8.0e33*kappa_y1^2*l1*m*r^2*cos(l1*(kappa_x1^2 + kappa_y1^2)^(1/2))*(kappa_x1^2 + kappa_y1^2)^2 + 2.0e33*kappa_y1^2*l1*m*r^2*cos(2.0*l1*(kappa_x1^2 + kappa_y1^2)^(1/2))*(kappa_x1^2 + kappa_y1^2)^2 - 4.0e33*kappa_x1^2*kappa_y1^2*l1*m*r^2*cos(l1*(kappa_x1^2 + kappa_y1^2)^(1/2))*(kappa_x1^2 + kappa_y1^2) - 2.0e33*kappa_x1^2*kappa_y1^2*l1*m*r^2*cos(2.0*l1*(kappa_x1^2 + kappa_y1^2)^(1/2))*(kappa_x1^2 + kappa_y1^2) - 4.0e33*kappa_x1^2*kappa_y1^4*l1^2*m*r^2*sin(l1*(kappa_x1^2 + kappa_y1^2)^(1/2))*(kappa_x1^2 + kappa_y1^2)^(1/2) - 4.0e33*kappa_x1^4*kappa_y1^2*l1^2*m*r^2*sin(l1*(kappa_x1^2 + kappa_y1^2)^(1/2))*(kappa_x1^2 + kappa_y1^2)^(1/2)))/(8000000000000000000000000000000000*l1^2*(kappa_x1^2 + kappa_y1^2)^4) + (dl1*(12.0*kappa_x1^5*l1^2*m*(kappa_x1^2 + kappa_y1^2)^(1/2) - 4.0*kappa_x1*l1^2*m*(kappa_x1^2 + kappa_y1^2)^(5/2) - 28.0*kappa_x1^5*l1*m*sin(l1*(kappa_x1^2 + kappa_y1^2)^(1/2)) - 4.0*kappa_x1*m*((kappa_x1^2 + kappa_y1^2)/kappa_x1^2)^(1/2)*(kappa_x1^2 + kappa_y1^2)^2 - 4.0*kappa_x1*kappa_y1^2*l1^2*m*(kappa_x1^2 + kappa_y1^2)^(3/2) - 1.3333333333333333333333333333333*kappa_x1*kappa_y1^2*l1^4*m*(kappa_x1^2 + kappa_y1^2)^(5/2) + 2.6666666666666666666666666666667*kappa_x1*kappa_y1^4*l1^4*m*(kappa_x1^2 + kappa_y1^2)^(3/2) + 2.0*kappa_x1^3*l1^2*m*((kappa_x1^2 + kappa_y1^2)/kappa_x1^2)^(1/2)*(kappa_x1^2 + kappa_y1^2)^2 + 4.0*kappa_x1^5*l1^2*m*cos(l1*(kappa_x1^2 + kappa_y1^2)^(1/2))*(kappa_x1^2 + kappa_y1^2)^(1/2) - 28.0*kappa_x1^3*kappa_y1^2*l1*m*sin(l1*(kappa_x1^2 + kappa_y1^2)^(1/2)) + 12.0*kappa_x1^3*kappa_y1^2*l1^2*m*(kappa_x1^2 + kappa_y1^2)^(1/2) + 2.6666666666666666666666666666667*kappa_x1^3*kappa_y1^2*l1^4*m*(kappa_x1^2 + kappa_y1^2)^(3/2) + 16.0*kappa_x1^3*l1*m*sin(l1*(kappa_x1^2 + kappa_y1^2)^(1/2))*(kappa_x1^2 + kappa_y1^2) + 4.0*kappa_x1*m*cos(l1*(kappa_x1^2 + kappa_y1^2)^(1/2))*((kappa_x1^2 + kappa_y1^2)/kappa_x1^2)^(1/2)*(kappa_x1^2 + kappa_y1^2)^2 + 4.0*kappa_x1^3*kappa_y1^2*l1^2*m*cos(l1*(kappa_x1^2 + kappa_y1^2)^(1/2))*(kappa_x1^2 + kappa_y1^2)^(1/2) + 4.0*kappa_x1*l1*m*sin(l1*(kappa_x1^2 + kappa_y1^2)^(1/2))*((kappa_x1^2 + kappa_y1^2)/kappa_x1^2)^(1/2)*(kappa_x1^2 + kappa_y1^2)^(5/2) + 2.0*kappa_x1*kappa_y1^2*l1^2*m*((kappa_x1^2 + kappa_y1^2)/kappa_x1^2)^(1/2)*(kappa_x1^2 + kappa_y1^2)^2 - 4.0*kappa_x1^3*l1^2*m*cos(l1*(kappa_x1^2 + kappa_y1^2)^(1/2))*((kappa_x1^2 + kappa_y1^2)/kappa_x1^2)^(1/2)*(kappa_x1^2 + kappa_y1^2)^2 + 8.0*kappa_x1*kappa_y1^2*l1*m*sin(l1*(kappa_x1^2 + kappa_y1^2)^(1/2))*(kappa_x1^2 + kappa_y1^2) - 4.0*kappa_x1*kappa_y1^2*l1^2*m*cos(l1*(kappa_x1^2 + kappa_y1^2)^(1/2))*((kappa_x1^2 + kappa_y1^2)/kappa_x1^2)^(1/2)*(kappa_x1^2 + kappa_y1^2)^2))/(2*l1^2*(kappa_x1^2 + kappa_y1^2)^(9/2)) + (dkappa_y1*(2.0e33*kappa_y1*l1^3*m*(kappa_x1^2 + kappa_y1^2)^(5/2) - 4.0e33*kappa_y1^3*l1^3*m*(kappa_x1^2 + kappa_y1^2)^(3/2) - 8.0e33*kappa_y1*l1*m*(kappa_x1^2 + kappa_y1^2)^(3/2) - 4.0e33*kappa_x1^2*kappa_y1*l1^3*m*(kappa_x1^2 + kappa_y1^2)^(3/2) - 2.0e33*kappa_y1^3*l1^3*m*cos(l1*(kappa_x1^2 + kappa_y1^2)^(1/2))*(kappa_x1^2 + kappa_y1^2)^(3/2) + 1.3333333333333333333333333333333e33*kappa_x1^6*kappa_y1*l1^3*m*((kappa_x1^2 + kappa_y1^2)/kappa_x1^2)^(1/2) + 8.0e33*kappa_y1*l1*m*cos(l1*(kappa_x1^2 + kappa_y1^2)^(1/2))*(kappa_x1^2 + kappa_y1^2)^(3/2) + 1.3333333333333333333333333333333e33*kappa_x1^2*kappa_y1^5*l1^3*m*((kappa_x1^2 + kappa_y1^2)/kappa_x1^2)^(1/2) + 2.6666666666666666666666666666667e33*kappa_x1^4*kappa_y1^3*l1^3*m*((kappa_x1^2 + kappa_y1^2)/kappa_x1^2)^(1/2) - 2.0e33*kappa_y1*l1^2*m*sin(l1*(kappa_x1^2 + kappa_y1^2)^(1/2))*(kappa_x1^2 + kappa_y1^2)^2 + 1.0e34*kappa_y1^3*l1^2*m*sin(l1*(kappa_x1^2 + kappa_y1^2)^(1/2))*(kappa_x1^2 + kappa_y1^2) + 333333333333333333333333333333333.0*kappa_x1^8*kappa_y1*l1^3*m*r^2*((kappa_x1^2 + kappa_y1^2)/kappa_x1^2)^(1/2) + 1.0e34*kappa_x1^2*kappa_y1*l1^2*m*sin(l1*(kappa_x1^2 + kappa_y1^2)^(1/2))*(kappa_x1^2 + kappa_y1^2) + 4.0e33*kappa_x1^2*kappa_y1*m*sin(l1*(kappa_x1^2 + kappa_y1^2)^(1/2))*((kappa_x1^2 + kappa_y1^2)/kappa_x1^2)^(1/2)*(kappa_x1^2 + kappa_y1^2)^(1/2) + 666666666666666666666666666666677.0*kappa_x1^2*kappa_y1^7*l1^3*m*r^2*((kappa_x1^2 + kappa_y1^2)/kappa_x1^2)^(1/2) + 1.6666666666666666666666666666667e33*kappa_x1^4*kappa_y1^5*l1^3*m*r^2*((kappa_x1^2 + kappa_y1^2)/kappa_x1^2)^(1/2) + 1.3333333333333333333333333333333e33*kappa_x1^6*kappa_y1^3*l1^3*m*r^2*((kappa_x1^2 + kappa_y1^2)/kappa_x1^2)^(1/2) - 2.0e33*kappa_x1^2*kappa_y1*l1^3*m*cos(l1*(kappa_x1^2 + kappa_y1^2)^(1/2))*(kappa_x1^2 + kappa_y1^2)^(3/2) + 500000000000000000000000000000000.0*kappa_x1^2*kappa_y1*m*sin(2.0*l1*(kappa_x1^2 + kappa_y1^2)^(1/2))*((kappa_x1^2 + kappa_y1^2)/kappa_x1^2)^(1/2)*(kappa_x1^2 + kappa_y1^2)^(1/2) - 4.0e33*kappa_x1^4*kappa_y1*l1^2*m*sin(l1*(kappa_x1^2 + kappa_y1^2)^(1/2))*((kappa_x1^2 + kappa_y1^2)/kappa_x1^2)^(1/2)*(kappa_x1^2 + kappa_y1^2)^(1/2) - 2.0e33*kappa_x1^2*kappa_y1*m*r^2*sin(l1*(kappa_x1^2 + kappa_y1^2)^(1/2))*((kappa_x1^2 + kappa_y1^2)/kappa_x1^2)^(1/2)*(kappa_x1^2 + kappa_y1^2)^(3/2) - 500000000000000000000000000000000.0*kappa_x1^4*kappa_y1*m*r^2*sin(l1*(kappa_x1^2 + kappa_y1^2)^(1/2))*((kappa_x1^2 + kappa_y1^2)/kappa_x1^2)^(1/2)*(kappa_x1^2 + kappa_y1^2)^(1/2) - 4.0e33*kappa_x1^2*kappa_y1*l1*m*cos(l1*(kappa_x1^2 + kappa_y1^2)^(1/2))*((kappa_x1^2 + kappa_y1^2)/kappa_x1^2)^(1/2)*(kappa_x1^2 + kappa_y1^2) + 250000000000000000000000000000000.0*kappa_x1^2*kappa_y1*m*r^2*sin(2.0*l1*(kappa_x1^2 + kappa_y1^2)^(1/2))*((kappa_x1^2 + kappa_y1^2)/kappa_x1^2)^(1/2)*(kappa_x1^2 + kappa_y1^2)^(3/2) - 250000000000000000000000000000000.0*kappa_x1^4*kappa_y1*m*r^2*sin(2.0*l1*(kappa_x1^2 + kappa_y1^2)^(1/2))*((kappa_x1^2 + kappa_y1^2)/kappa_x1^2)^(1/2)*(kappa_x1^2 + kappa_y1^2)^(1/2) - 4.0e33*kappa_x1^2*kappa_y1^3*l1^2*m*sin(l1*(kappa_x1^2 + kappa_y1^2)^(1/2))*((kappa_x1^2 + kappa_y1^2)/kappa_x1^2)^(1/2)*(kappa_x1^2 + kappa_y1^2)^(1/2) + 500000000000000000000000000000000.0*kappa_x1^2*kappa_y1^3*m*r^2*sin(l1*(kappa_x1^2 + kappa_y1^2)^(1/2))*((kappa_x1^2 + kappa_y1^2)/kappa_x1^2)^(1/2)*(kappa_x1^2 + kappa_y1^2)^(1/2) - 1.0e33*kappa_x1^2*kappa_y1*l1*m*cos(2.0*l1*(kappa_x1^2 + kappa_y1^2)^(1/2))*((kappa_x1^2 + kappa_y1^2)/kappa_x1^2)^(1/2)*(kappa_x1^2 + kappa_y1^2) - 125000000000000000000000000000000.0*kappa_x1^2*kappa_y1^3*m*r^2*sin(2.0*l1*(kappa_x1^2 + kappa_y1^2)^(1/2))*((kappa_x1^2 + kappa_y1^2)/kappa_x1^2)^(1/2)*(kappa_x1^2 + kappa_y1^2)^(1/2) + 500000000000000000000000000000000.0*kappa_x1^6*kappa_y1*l1^2*m*r^2*sin(l1*(kappa_x1^2 + kappa_y1^2)^(1/2))*((kappa_x1^2 + kappa_y1^2)/kappa_x1^2)^(1/2)*(kappa_x1^2 + kappa_y1^2)^(1/2) + 500000000000000000000000000000000.0*kappa_x1^4*kappa_y1*l1*m*r^2*cos(l1*(kappa_x1^2 + kappa_y1^2)^(1/2))*((kappa_x1^2 + kappa_y1^2)/kappa_x1^2)^(1/2)*(kappa_x1^2 + kappa_y1^2) - 500000000000000000000000000000000.0*kappa_x1^2*kappa_y1^5*l1^2*m*r^2*sin(l1*(kappa_x1^2 + kappa_y1^2)^(1/2))*((kappa_x1^2 + kappa_y1^2)/kappa_x1^2)^(1/2)*(kappa_x1^2 + kappa_y1^2)^(1/2) + 500000000000000000000000000000000.0*kappa_x1^4*kappa_y1*l1*m*r^2*cos(2.0*l1*(kappa_x1^2 + kappa_y1^2)^(1/2))*((kappa_x1^2 + kappa_y1^2)/kappa_x1^2)^(1/2)*(kappa_x1^2 + kappa_y1^2) + 2.0e33*kappa_x1^2*kappa_y1*l1*m*r^2*cos(l1*(kappa_x1^2 + kappa_y1^2)^(1/2))*((kappa_x1^2 + kappa_y1^2)/kappa_x1^2)^(1/2)*(kappa_x1^2 + kappa_y1^2)^2 - 500000000000000000000000000000000.0*kappa_x1^2*kappa_y1^3*l1*m*r^2*cos(l1*(kappa_x1^2 + kappa_y1^2)^(1/2))*((kappa_x1^2 + kappa_y1^2)/kappa_x1^2)^(1/2)*(kappa_x1^2 + kappa_y1^2) - 500000000000000000000000000000000.0*kappa_x1^2*kappa_y1*l1*m*r^2*cos(2.0*l1*(kappa_x1^2 + kappa_y1^2)^(1/2))*((kappa_x1^2 + kappa_y1^2)/kappa_x1^2)^(1/2)*(kappa_x1^2 + kappa_y1^2)^2 + 250000000000000000000000000000000.0*kappa_x1^2*kappa_y1^3*l1*m*r^2*cos(2.0*l1*(kappa_x1^2 + kappa_y1^2)^(1/2))*((kappa_x1^2 + kappa_y1^2)/kappa_x1^2)^(1/2)*(kappa_x1^2 + kappa_y1^2)))/(2000000000000000000000000000000000*kappa_x1*l1^2*((kappa_x1^2 + kappa_y1^2)/kappa_x1^2)^(1/2)*(kappa_x1^2 + kappa_y1^2)^4);
% V(2,2) = (dl1*(5.3333333333333333333333333333333e33*kappa_x1^6*l1^3*m + 5.3333333333333333333333333333333e33*kappa_x1^2*kappa_y1^4*l1^3*m + 1.0666666666666666666666666666667e34*kappa_x1^4*kappa_y1^2*l1^3*m + 1.3333333333333333333333333333333e33*kappa_x1^8*l1^3*m*r^2 + 3.2e34*kappa_x1^2*m*sin(l1*(kappa_x1^2 + kappa_y1^2)^(1/2))*(kappa_x1^2 + kappa_y1^2)^(1/2) + 1.6e34*kappa_y1^2*m*sin(l1*(kappa_x1^2 + kappa_y1^2)^(1/2))*(kappa_x1^2 + kappa_y1^2)^(1/2) - 2.0e33*kappa_y1^2*m*sin(2.0*l1*(kappa_x1^2 + kappa_y1^2)^(1/2))*(kappa_x1^2 + kappa_y1^2)^(1/2) - 1.6e34*kappa_x1^4*l1^2*m*sin(l1*(kappa_x1^2 + kappa_y1^2)^(1/2))*(kappa_x1^2 + kappa_y1^2)^(1/2) + 8.0e33*kappa_y1^2*m*r^2*sin(l1*(kappa_x1^2 + kappa_y1^2)^(1/2))*(kappa_x1^2 + kappa_y1^2)^(3/2) - 3.2e34*kappa_x1^2*l1*m*cos(l1*(kappa_x1^2 + kappa_y1^2)^(1/2))*(kappa_x1^2 + kappa_y1^2) - 1.6e34*kappa_y1^2*l1*m*cos(l1*(kappa_x1^2 + kappa_y1^2)^(1/2))*(kappa_x1^2 + kappa_y1^2) - 1.0e33*kappa_y1^2*m*r^2*sin(2.0*l1*(kappa_x1^2 + kappa_y1^2)^(1/2))*(kappa_x1^2 + kappa_y1^2)^(3/2) + 500000000000000000000000000000000.0*kappa_y1^4*m*r^2*sin(2.0*l1*(kappa_x1^2 + kappa_y1^2)^(1/2))*(kappa_x1^2 + kappa_y1^2)^(1/2) + 4.0e33*kappa_y1^2*l1*m*cos(2.0*l1*(kappa_x1^2 + kappa_y1^2)^(1/2))*(kappa_x1^2 + kappa_y1^2) + 2.6666666666666666666666666666667e33*kappa_x1^2*kappa_y1^6*l1^3*m*r^2 + 6.6666666666666666666666666666667e33*kappa_x1^4*kappa_y1^4*l1^3*m*r^2 + 5.3333333333333333333333333333333e33*kappa_x1^6*kappa_y1^2*l1^3*m*r^2 - 1.6e34*kappa_x1^2*kappa_y1^2*l1^2*m*sin(l1*(kappa_x1^2 + kappa_y1^2)^(1/2))*(kappa_x1^2 + kappa_y1^2)^(1/2) + 4.0e33*kappa_x1^2*kappa_y1^2*m*r^2*sin(l1*(kappa_x1^2 + kappa_y1^2)^(1/2))*(kappa_x1^2 + kappa_y1^2)^(1/2) + 1.0e33*kappa_x1^2*kappa_y1^2*m*r^2*sin(2.0*l1*(kappa_x1^2 + kappa_y1^2)^(1/2))*(kappa_x1^2 + kappa_y1^2)^(1/2) - 1.0e33*kappa_y1^4*l1*m*r^2*cos(2.0*l1*(kappa_x1^2 + kappa_y1^2)^(1/2))*(kappa_x1^2 + kappa_y1^2) - 8.0e33*kappa_y1^2*l1*m*r^2*cos(l1*(kappa_x1^2 + kappa_y1^2)^(1/2))*(kappa_x1^2 + kappa_y1^2)^2 + 2.0e33*kappa_y1^2*l1*m*r^2*cos(2.0*l1*(kappa_x1^2 + kappa_y1^2)^(1/2))*(kappa_x1^2 + kappa_y1^2)^2 - 4.0e33*kappa_x1^2*kappa_y1^2*l1*m*r^2*cos(l1*(kappa_x1^2 + kappa_y1^2)^(1/2))*(kappa_x1^2 + kappa_y1^2) - 2.0e33*kappa_x1^2*kappa_y1^2*l1*m*r^2*cos(2.0*l1*(kappa_x1^2 + kappa_y1^2)^(1/2))*(kappa_x1^2 + kappa_y1^2) - 4.0e33*kappa_x1^2*kappa_y1^4*l1^2*m*r^2*sin(l1*(kappa_x1^2 + kappa_y1^2)^(1/2))*(kappa_x1^2 + kappa_y1^2)^(1/2) - 4.0e33*kappa_x1^4*kappa_y1^2*l1^2*m*r^2*sin(l1*(kappa_x1^2 + kappa_y1^2)^(1/2))*(kappa_x1^2 + kappa_y1^2)^(1/2)))/(8000000000000000000000000000000000*l1^2*(kappa_x1^2 + kappa_y1^2)^4) - (2.5e-33*dkappa_y1*(2.4e33*kappa_y1^5*l1*m + 1.6e33*kappa_y1*m*sin(l1*(kappa_x1^2 + kappa_y1^2)^(1/2))*(kappa_x1^2 + kappa_y1^2)^(3/2) + 533333333333333333333333333333344.0*kappa_x1^2*kappa_y1^5*l1^3*m + 1.0666666666666666666666666666667e33*kappa_x1^4*kappa_y1^3*l1^3*m - 200000000000000000000000000000000.0*kappa_y1*m*sin(2.0*l1*(kappa_x1^2 + kappa_y1^2)^(1/2))*(kappa_x1^2 + kappa_y1^2)^(3/2) + 3.6e33*kappa_x1^4*kappa_y1*l1*m - 5.6e33*kappa_y1^3*m*sin(l1*(kappa_x1^2 + kappa_y1^2)^(1/2))*(kappa_x1^2 + kappa_y1^2)^(1/2) + 800000000000000000000000000000000.0*kappa_y1^5*l1*m*cos(l1*(kappa_x1^2 + kappa_y1^2)^(1/2)) + 700000000000000000000000000000000.0*kappa_y1^3*m*sin(2.0*l1*(kappa_x1^2 + kappa_y1^2)^(1/2))*(kappa_x1^2 + kappa_y1^2)^(1/2) - 200000000000000000000000000000000.0*kappa_y1^5*l1*m*cos(2.0*l1*(kappa_x1^2 + kappa_y1^2)^(1/2)) + 6.0e33*kappa_x1^2*kappa_y1^3*l1*m + 533333333333333333333333333333344.0*kappa_x1^6*kappa_y1*l1^3*m + 700000000000000000000000000000000.0*kappa_y1^7*l1*m*r^2 - 100000000000000000000000000000000.0*kappa_y1*m*r^2*sin(2.0*l1*(kappa_x1^2 + kappa_y1^2)^(1/2))*(kappa_x1^2 + kappa_y1^2)^(5/2) - 800000000000000000000000000000000.0*kappa_x1^6*kappa_y1*l1*m*r^2 - 2.0e33*kappa_y1^3*m*r^2*sin(l1*(kappa_x1^2 + kappa_y1^2)^(1/2))*(kappa_x1^2 + kappa_y1^2)^(3/2) + 7.2e33*kappa_x1^2*kappa_y1^3*l1*m*cos(l1*(kappa_x1^2 + kappa_y1^2)^(1/2)) + 400000000000000000000000000000000.0*kappa_y1^7*l1*m*r^2*cos(l1*(kappa_x1^2 + kappa_y1^2)^(1/2)) + 350000000000000000000000000000000.0*kappa_y1^3*m*r^2*sin(2.0*l1*(kappa_x1^2 + kappa_y1^2)^(1/2))*(kappa_x1^2 + kappa_y1^2)^(3/2) - 175000000000000000000000000000000.0*kappa_y1^5*m*r^2*sin(2.0*l1*(kappa_x1^2 + kappa_y1^2)^(1/2))*(kappa_x1^2 + kappa_y1^2)^(1/2) - 200000000000000000000000000000000.0*kappa_x1^2*kappa_y1^3*l1*m*cos(2.0*l1*(kappa_x1^2 + kappa_y1^2)^(1/2)) - 50000000000000000000000000000000.0*kappa_y1^7*l1*m*r^2*cos(2.0*l1*(kappa_x1^2 + kappa_y1^2)^(1/2)) + 900000000000000000000000000000000.0*kappa_x1^2*kappa_y1^5*l1*m*r^2 - 600000000000000000000000000000000.0*kappa_x1^4*kappa_y1^3*l1*m*r^2 - 1.12e34*kappa_x1^2*kappa_y1*m*sin(l1*(kappa_x1^2 + kappa_y1^2)^(1/2))*(kappa_x1^2 + kappa_y1^2)^(1/2) + 800000000000000000000000000000000.0*kappa_y1*m*r^2*sin(l1*(kappa_x1^2 + kappa_y1^2)^(1/2))*(kappa_x1^2 + kappa_y1^2)^(5/2) + 6.4e33*kappa_x1^4*kappa_y1*l1*m*cos(l1*(kappa_x1^2 + kappa_y1^2)^(1/2)) + 133333333333333333333333333333333.0*kappa_x1^2*kappa_y1^7*l1^3*m*r^2 + 266666666666666666666666666666677.0*kappa_x1^4*kappa_y1^5*l1^3*m*r^2 + 133333333333333333333333333333333.0*kappa_x1^6*kappa_y1^3*l1^3*m*r^2 + 800000000000000000000000000000000.0*kappa_x1^2*kappa_y1^3*l1^2*m*sin(l1*(kappa_x1^2 + kappa_y1^2)^(1/2))*(kappa_x1^2 + kappa_y1^2)^(1/2) - 1.4e33*kappa_x1^2*kappa_y1^3*m*r^2*sin(l1*(kappa_x1^2 + kappa_y1^2)^(1/2))*(kappa_x1^2 + kappa_y1^2)^(1/2) + 1.8e33*kappa_x1^2*kappa_y1^5*l1*m*r^2*cos(l1*(kappa_x1^2 + kappa_y1^2)^(1/2)) + 1.0e33*kappa_x1^4*kappa_y1^3*l1*m*r^2*cos(l1*(kappa_x1^2 + kappa_y1^2)^(1/2)) - 350000000000000000000000000000000.0*kappa_x1^2*kappa_y1^3*m*r^2*sin(2.0*l1*(kappa_x1^2 + kappa_y1^2)^(1/2))*(kappa_x1^2 + kappa_y1^2)^(1/2) - 50000000000000000000000000000000.0*kappa_x1^2*kappa_y1^5*l1*m*r^2*cos(2.0*l1*(kappa_x1^2 + kappa_y1^2)^(1/2)) + 800000000000000000000000000000000.0*kappa_x1^4*kappa_y1*l1^2*m*sin(l1*(kappa_x1^2 + kappa_y1^2)^(1/2))*(kappa_x1^2 + kappa_y1^2)^(1/2) + 400000000000000000000000000000000.0*kappa_x1^2*kappa_y1*m*r^2*sin(l1*(kappa_x1^2 + kappa_y1^2)^(1/2))*(kappa_x1^2 + kappa_y1^2)^(3/2) - 400000000000000000000000000000000.0*kappa_x1^6*kappa_y1*l1*m*r^2*cos(l1*(kappa_x1^2 + kappa_y1^2)^(1/2)) + 100000000000000000000000000000000.0*kappa_x1^2*kappa_y1*m*r^2*sin(2.0*l1*(kappa_x1^2 + kappa_y1^2)^(1/2))*(kappa_x1^2 + kappa_y1^2)^(3/2) + 200000000000000000000000000000000.0*kappa_x1^2*kappa_y1^5*l1^2*m*r^2*sin(l1*(kappa_x1^2 + kappa_y1^2)^(1/2))*(kappa_x1^2 + kappa_y1^2)^(1/2) + 200000000000000000000000000000000.0*kappa_x1^4*kappa_y1^3*l1^2*m*r^2*sin(l1*(kappa_x1^2 + kappa_y1^2)^(1/2))*(kappa_x1^2 + kappa_y1^2)^(1/2)))/(l1*(kappa_x1^2 + kappa_y1^2)^5) - (2.5e-33*dkappa_x1*(3.2e33*kappa_x1^5*l1*m + 266666666666666666666666666666666.0*kappa_x1^7*l1^3*m + 3.2e33*kappa_x1*m*sin(l1*(kappa_x1^2 + kappa_y1^2)^(1/2))*(kappa_x1^2 + kappa_y1^2)^(3/2) - 266666666666666666666666666666677.0*kappa_x1^3*kappa_y1^4*l1^3*m + 266666666666666666666666666666666.0*kappa_x1^5*kappa_y1^2*l1^3*m + 2.0e33*kappa_x1*kappa_y1^4*l1*m - 1.12e34*kappa_x1^3*m*sin(l1*(kappa_x1^2 + kappa_y1^2)^(1/2))*(kappa_x1^2 + kappa_y1^2)^(1/2) + 4.8e33*kappa_x1^5*l1*m*cos(l1*(kappa_x1^2 + kappa_y1^2)^(1/2)) + 5.2e33*kappa_x1^3*kappa_y1^2*l1*m - 266666666666666666666666666666677.0*kappa_x1*kappa_y1^6*l1^3*m + 700000000000000000000000000000000.0*kappa_x1*kappa_y1^2*m*sin(2.0*l1*(kappa_x1^2 + kappa_y1^2)^(1/2))*(kappa_x1^2 + kappa_y1^2)^(1/2) - 200000000000000000000000000000000.0*kappa_x1*kappa_y1^4*l1*m*cos(2.0*l1*(kappa_x1^2 + kappa_y1^2)^(1/2)) + 1.3e33*kappa_x1*kappa_y1^6*l1*m*r^2 + 800000000000000000000000000000000.0*kappa_x1^5*l1^2*m*sin(l1*(kappa_x1^2 + kappa_y1^2)^(1/2))*(kappa_x1^2 + kappa_y1^2)^(1/2) + 4.0e33*kappa_x1^3*kappa_y1^2*l1*m*cos(l1*(kappa_x1^2 + kappa_y1^2)^(1/2)) - 200000000000000000000000000000000.0*kappa_x1^3*kappa_y1^2*l1*m*cos(2.0*l1*(kappa_x1^2 + kappa_y1^2)^(1/2)) + 2.9e33*kappa_x1^3*kappa_y1^4*l1*m*r^2 + 1.6e33*kappa_x1^5*kappa_y1^2*l1*m*r^2 - 133333333333333333333333333333333.0*kappa_x1*kappa_y1^8*l1^3*m*r^2 - 5.6e33*kappa_x1*kappa_y1^2*m*sin(l1*(kappa_x1^2 + kappa_y1^2)^(1/2))*(kappa_x1^2 + kappa_y1^2)^(1/2) - 800000000000000000000000000000000.0*kappa_x1*kappa_y1^4*l1*m*cos(l1*(kappa_x1^2 + kappa_y1^2)^(1/2)) - 266666666666666666666666666666677.0*kappa_x1^3*kappa_y1^6*l1^3*m*r^2 - 133333333333333333333333333333344.0*kappa_x1^5*kappa_y1^4*l1^3*m*r^2 + 3.0*kappa_x1^7*kappa_y1^2*l1^3*m*r^2 - 50000000000000000000000000000000.0*kappa_x1*kappa_y1^6*l1*m*r^2*cos(2.0*l1*(kappa_x1^2 + kappa_y1^2)^(1/2)) + 800000000000000000000000000000000.0*kappa_x1^3*kappa_y1^2*l1^2*m*sin(l1*(kappa_x1^2 + kappa_y1^2)^(1/2))*(kappa_x1^2 + kappa_y1^2)^(1/2) - 1.4e33*kappa_x1^3*kappa_y1^2*m*r^2*sin(l1*(kappa_x1^2 + kappa_y1^2)^(1/2))*(kappa_x1^2 + kappa_y1^2)^(1/2) + 1.4e33*kappa_x1^3*kappa_y1^4*l1*m*r^2*cos(l1*(kappa_x1^2 + kappa_y1^2)^(1/2)) + 1.4e33*kappa_x1^5*kappa_y1^2*l1*m*r^2*cos(l1*(kappa_x1^2 + kappa_y1^2)^(1/2)) - 350000000000000000000000000000000.0*kappa_x1^3*kappa_y1^2*m*r^2*sin(2.0*l1*(kappa_x1^2 + kappa_y1^2)^(1/2))*(kappa_x1^2 + kappa_y1^2)^(1/2) - 50000000000000000000000000000000.0*kappa_x1^3*kappa_y1^4*l1*m*r^2*cos(2.0*l1*(kappa_x1^2 + kappa_y1^2)^(1/2)) - 1.6e33*kappa_x1*kappa_y1^2*m*r^2*sin(l1*(kappa_x1^2 + kappa_y1^2)^(1/2))*(kappa_x1^2 + kappa_y1^2)^(3/2) + 350000000000000000000000000000000.0*kappa_x1*kappa_y1^2*m*r^2*sin(2.0*l1*(kappa_x1^2 + kappa_y1^2)^(1/2))*(kappa_x1^2 + kappa_y1^2)^(3/2) - 175000000000000000000000000000000.0*kappa_x1*kappa_y1^4*m*r^2*sin(2.0*l1*(kappa_x1^2 + kappa_y1^2)^(1/2))*(kappa_x1^2 + kappa_y1^2)^(1/2) + 200000000000000000000000000000000.0*kappa_x1^3*kappa_y1^4*l1^2*m*r^2*sin(l1*(kappa_x1^2 + kappa_y1^2)^(1/2))*(kappa_x1^2 + kappa_y1^2)^(1/2) + 200000000000000000000000000000000.0*kappa_x1^5*kappa_y1^2*l1^2*m*r^2*sin(l1*(kappa_x1^2 + kappa_y1^2)^(1/2))*(kappa_x1^2 + kappa_y1^2)^(1/2)))/(l1*(kappa_x1^2 + kappa_y1^2)^5);
% V(2,3) = (dkappa_y1*(5.6e33*kappa_x1^5*l1*m + 533333333333333333333333333333333.0*kappa_x1^7*l1^3*m - 533333333333333333333333333333333.0*kappa_x1^3*kappa_y1^4*l1^3*m + 533333333333333333333333333333322.0*kappa_x1^5*kappa_y1^2*l1^3*m + 133333333333333333333333333333333.0*kappa_x1^9*l1^3*m*r^2 - 800000000000000000000000000000000.0*kappa_x1*m*sin(2.0*l1*(kappa_x1^2 + kappa_y1^2)^(1/2))*(kappa_x1^2 + kappa_y1^2)^(3/2) + 3.2e33*kappa_x1*kappa_y1^4*l1*m - 1.12e34*kappa_x1^3*m*sin(l1*(kappa_x1^2 + kappa_y1^2)^(1/2))*(kappa_x1^2 + kappa_y1^2)^(1/2) + 4.8e33*kappa_x1^5*l1*m*cos(l1*(kappa_x1^2 + kappa_y1^2)^(1/2)) + 1.4e33*kappa_x1^3*m*sin(2.0*l1*(kappa_x1^2 + kappa_y1^2)^(1/2))*(kappa_x1^2 + kappa_y1^2)^(1/2) - 400000000000000000000000000000000.0*kappa_x1^5*l1*m*cos(2.0*l1*(kappa_x1^2 + kappa_y1^2)^(1/2)) + 8.8e33*kappa_x1^3*kappa_y1^2*l1*m - 533333333333333333333333333333344.0*kappa_x1*kappa_y1^6*l1^3*m + 2.8e33*kappa_x1*kappa_y1^2*m*sin(2.0*l1*(kappa_x1^2 + kappa_y1^2)^(1/2))*(kappa_x1^2 + kappa_y1^2)^(1/2) - 400000000000000000000000000000000.0*kappa_x1*m*r^2*sin(2.0*l1*(kappa_x1^2 + kappa_y1^2)^(1/2))*(kappa_x1^2 + kappa_y1^2)^(5/2) - 800000000000000000000000000000000.0*kappa_x1*kappa_y1^4*l1*m*cos(2.0*l1*(kappa_x1^2 + kappa_y1^2)^(1/2)) + 2.8e33*kappa_x1*kappa_y1^6*l1*m*r^2 - 3.6e33*kappa_x1^3*m*r^2*sin(l1*(kappa_x1^2 + kappa_y1^2)^(1/2))*(kappa_x1^2 + kappa_y1^2)^(3/2) - 1.6e33*kappa_x1^3*kappa_y1^2*l1*m*cos(l1*(kappa_x1^2 + kappa_y1^2)^(1/2)) + 400000000000000000000000000000000.0*kappa_x1^7*l1*m*r^2*cos(l1*(kappa_x1^2 + kappa_y1^2)^(1/2)) + 1.1e33*kappa_x1^3*m*r^2*sin(2.0*l1*(kappa_x1^2 + kappa_y1^2)^(1/2))*(kappa_x1^2 + kappa_y1^2)^(3/2) - 700000000000000000000000000000000.0*kappa_x1^5*m*r^2*sin(2.0*l1*(kappa_x1^2 + kappa_y1^2)^(1/2))*(kappa_x1^2 + kappa_y1^2)^(1/2) - 1.2e33*kappa_x1^3*kappa_y1^2*l1*m*cos(2.0*l1*(kappa_x1^2 + kappa_y1^2)^(1/2)) + 6.2e33*kappa_x1^3*kappa_y1^4*l1*m*r^2 + 3.4e33*kappa_x1^5*kappa_y1^2*l1*m*r^2 + 133333333333333333333333333333333.0*kappa_x1*kappa_y1^8*l1^3*m*r^2 + 3.2e33*kappa_x1*m*r^2*sin(l1*(kappa_x1^2 + kappa_y1^2)^(1/2))*(kappa_x1^2 + kappa_y1^2)^(5/2) - 6.4e33*kappa_x1*kappa_y1^4*l1*m*cos(l1*(kappa_x1^2 + kappa_y1^2)^(1/2)) + 800000000000000000000000000000000.0*kappa_x1^3*kappa_y1^6*l1^3*m*r^2 + 1.3333333333333333333333333333333e33*kappa_x1^5*kappa_y1^4*l1^3*m*r^2 + 800000000000000000000000000000000.0*kappa_x1^7*kappa_y1^2*l1^3*m*r^2 - 200000000000000000000000000000000.0*kappa_x1*kappa_y1^6*l1*m*r^2*cos(2.0*l1*(kappa_x1^2 + kappa_y1^2)^(1/2)) - 1.6e33*kappa_x1^3*kappa_y1^2*l1^2*m*sin(l1*(kappa_x1^2 + kappa_y1^2)^(1/2))*(kappa_x1^2 + kappa_y1^2)^(1/2) + 4.8e33*kappa_x1^3*kappa_y1^4*l1*m*r^2*cos(l1*(kappa_x1^2 + kappa_y1^2)^(1/2)) + 4.4e33*kappa_x1^5*kappa_y1^2*l1*m*r^2*cos(l1*(kappa_x1^2 + kappa_y1^2)^(1/2)) - 1.75e33*kappa_x1^3*kappa_y1^2*m*r^2*sin(2.0*l1*(kappa_x1^2 + kappa_y1^2)^(1/2))*(kappa_x1^2 + kappa_y1^2)^(1/2) - 300000000000000000000000000000000.0*kappa_x1^3*kappa_y1^4*l1*m*r^2*cos(2.0*l1*(kappa_x1^2 + kappa_y1^2)^(1/2)) - 100000000000000000000000000000000.0*kappa_x1^5*kappa_y1^2*l1*m*r^2*cos(2.0*l1*(kappa_x1^2 + kappa_y1^2)^(1/2)) - 1.6e33*kappa_x1*kappa_y1^4*l1^2*m*sin(l1*(kappa_x1^2 + kappa_y1^2)^(1/2))*(kappa_x1^2 + kappa_y1^2)^(1/2) - 1.0e34*kappa_x1*kappa_y1^2*m*r^2*sin(l1*(kappa_x1^2 + kappa_y1^2)^(1/2))*(kappa_x1^2 + kappa_y1^2)^(3/2) + 2.8e33*kappa_x1*kappa_y1^4*m*r^2*sin(l1*(kappa_x1^2 + kappa_y1^2)^(1/2))*(kappa_x1^2 + kappa_y1^2)^(1/2) + 800000000000000000000000000000000.0*kappa_x1*kappa_y1^6*l1*m*r^2*cos(l1*(kappa_x1^2 + kappa_y1^2)^(1/2)) + 1.4e33*kappa_x1*kappa_y1^2*m*r^2*sin(2.0*l1*(kappa_x1^2 + kappa_y1^2)^(1/2))*(kappa_x1^2 + kappa_y1^2)^(3/2) - 700000000000000000000000000000000.0*kappa_x1*kappa_y1^4*m*r^2*sin(2.0*l1*(kappa_x1^2 + kappa_y1^2)^(1/2))*(kappa_x1^2 + kappa_y1^2)^(1/2) - 400000000000000000000000000000000.0*kappa_x1*kappa_y1^6*l1^2*m*r^2*sin(l1*(kappa_x1^2 + kappa_y1^2)^(1/2))*(kappa_x1^2 + kappa_y1^2)^(1/2) - 400000000000000000000000000000000.0*kappa_x1^3*kappa_y1^4*l1^2*m*r^2*sin(l1*(kappa_x1^2 + kappa_y1^2)^(1/2))*(kappa_x1^2 + kappa_y1^2)^(1/2)))/(800000000000000000000000000000000*l1*(kappa_x1^2 + kappa_y1^2)^5) - (2.5e-33*dkappa_x1*(2.4e33*kappa_y1^5*l1*m + 1.6e33*kappa_y1*m*sin(l1*(kappa_x1^2 + kappa_y1^2)^(1/2))*(kappa_x1^2 + kappa_y1^2)^(3/2) + 533333333333333333333333333333344.0*kappa_x1^2*kappa_y1^5*l1^3*m + 1.0666666666666666666666666666667e33*kappa_x1^4*kappa_y1^3*l1^3*m - 200000000000000000000000000000000.0*kappa_y1*m*sin(2.0*l1*(kappa_x1^2 + kappa_y1^2)^(1/2))*(kappa_x1^2 + kappa_y1^2)^(3/2) + 3.6e33*kappa_x1^4*kappa_y1*l1*m - 5.6e33*kappa_y1^3*m*sin(l1*(kappa_x1^2 + kappa_y1^2)^(1/2))*(kappa_x1^2 + kappa_y1^2)^(1/2) + 800000000000000000000000000000000.0*kappa_y1^5*l1*m*cos(l1*(kappa_x1^2 + kappa_y1^2)^(1/2)) + 700000000000000000000000000000000.0*kappa_y1^3*m*sin(2.0*l1*(kappa_x1^2 + kappa_y1^2)^(1/2))*(kappa_x1^2 + kappa_y1^2)^(1/2) - 200000000000000000000000000000000.0*kappa_y1^5*l1*m*cos(2.0*l1*(kappa_x1^2 + kappa_y1^2)^(1/2)) + 6.0e33*kappa_x1^2*kappa_y1^3*l1*m + 533333333333333333333333333333344.0*kappa_x1^6*kappa_y1*l1^3*m + 700000000000000000000000000000000.0*kappa_y1^7*l1*m*r^2 - 100000000000000000000000000000000.0*kappa_y1*m*r^2*sin(2.0*l1*(kappa_x1^2 + kappa_y1^2)^(1/2))*(kappa_x1^2 + kappa_y1^2)^(5/2) - 800000000000000000000000000000000.0*kappa_x1^6*kappa_y1*l1*m*r^2 - 2.0e33*kappa_y1^3*m*r^2*sin(l1*(kappa_x1^2 + kappa_y1^2)^(1/2))*(kappa_x1^2 + kappa_y1^2)^(3/2) + 7.2e33*kappa_x1^2*kappa_y1^3*l1*m*cos(l1*(kappa_x1^2 + kappa_y1^2)^(1/2)) + 400000000000000000000000000000000.0*kappa_y1^7*l1*m*r^2*cos(l1*(kappa_x1^2 + kappa_y1^2)^(1/2)) + 350000000000000000000000000000000.0*kappa_y1^3*m*r^2*sin(2.0*l1*(kappa_x1^2 + kappa_y1^2)^(1/2))*(kappa_x1^2 + kappa_y1^2)^(3/2) - 175000000000000000000000000000000.0*kappa_y1^5*m*r^2*sin(2.0*l1*(kappa_x1^2 + kappa_y1^2)^(1/2))*(kappa_x1^2 + kappa_y1^2)^(1/2) - 200000000000000000000000000000000.0*kappa_x1^2*kappa_y1^3*l1*m*cos(2.0*l1*(kappa_x1^2 + kappa_y1^2)^(1/2)) - 50000000000000000000000000000000.0*kappa_y1^7*l1*m*r^2*cos(2.0*l1*(kappa_x1^2 + kappa_y1^2)^(1/2)) + 900000000000000000000000000000000.0*kappa_x1^2*kappa_y1^5*l1*m*r^2 - 600000000000000000000000000000000.0*kappa_x1^4*kappa_y1^3*l1*m*r^2 - 1.12e34*kappa_x1^2*kappa_y1*m*sin(l1*(kappa_x1^2 + kappa_y1^2)^(1/2))*(kappa_x1^2 + kappa_y1^2)^(1/2) + 800000000000000000000000000000000.0*kappa_y1*m*r^2*sin(l1*(kappa_x1^2 + kappa_y1^2)^(1/2))*(kappa_x1^2 + kappa_y1^2)^(5/2) + 6.4e33*kappa_x1^4*kappa_y1*l1*m*cos(l1*(kappa_x1^2 + kappa_y1^2)^(1/2)) + 133333333333333333333333333333333.0*kappa_x1^2*kappa_y1^7*l1^3*m*r^2 + 266666666666666666666666666666677.0*kappa_x1^4*kappa_y1^5*l1^3*m*r^2 + 133333333333333333333333333333333.0*kappa_x1^6*kappa_y1^3*l1^3*m*r^2 + 800000000000000000000000000000000.0*kappa_x1^2*kappa_y1^3*l1^2*m*sin(l1*(kappa_x1^2 + kappa_y1^2)^(1/2))*(kappa_x1^2 + kappa_y1^2)^(1/2) - 1.4e33*kappa_x1^2*kappa_y1^3*m*r^2*sin(l1*(kappa_x1^2 + kappa_y1^2)^(1/2))*(kappa_x1^2 + kappa_y1^2)^(1/2) + 1.8e33*kappa_x1^2*kappa_y1^5*l1*m*r^2*cos(l1*(kappa_x1^2 + kappa_y1^2)^(1/2)) + 1.0e33*kappa_x1^4*kappa_y1^3*l1*m*r^2*cos(l1*(kappa_x1^2 + kappa_y1^2)^(1/2)) - 350000000000000000000000000000000.0*kappa_x1^2*kappa_y1^3*m*r^2*sin(2.0*l1*(kappa_x1^2 + kappa_y1^2)^(1/2))*(kappa_x1^2 + kappa_y1^2)^(1/2) - 50000000000000000000000000000000.0*kappa_x1^2*kappa_y1^5*l1*m*r^2*cos(2.0*l1*(kappa_x1^2 + kappa_y1^2)^(1/2)) + 800000000000000000000000000000000.0*kappa_x1^4*kappa_y1*l1^2*m*sin(l1*(kappa_x1^2 + kappa_y1^2)^(1/2))*(kappa_x1^2 + kappa_y1^2)^(1/2) + 400000000000000000000000000000000.0*kappa_x1^2*kappa_y1*m*r^2*sin(l1*(kappa_x1^2 + kappa_y1^2)^(1/2))*(kappa_x1^2 + kappa_y1^2)^(3/2) - 400000000000000000000000000000000.0*kappa_x1^6*kappa_y1*l1*m*r^2*cos(l1*(kappa_x1^2 + kappa_y1^2)^(1/2)) + 100000000000000000000000000000000.0*kappa_x1^2*kappa_y1*m*r^2*sin(2.0*l1*(kappa_x1^2 + kappa_y1^2)^(1/2))*(kappa_x1^2 + kappa_y1^2)^(3/2) + 200000000000000000000000000000000.0*kappa_x1^2*kappa_y1^5*l1^2*m*r^2*sin(l1*(kappa_x1^2 + kappa_y1^2)^(1/2))*(kappa_x1^2 + kappa_y1^2)^(1/2) + 200000000000000000000000000000000.0*kappa_x1^4*kappa_y1^3*l1^2*m*r^2*sin(l1*(kappa_x1^2 + kappa_y1^2)^(1/2))*(kappa_x1^2 + kappa_y1^2)^(1/2)))/(l1*(kappa_x1^2 + kappa_y1^2)^5) + (dl1*(2.0e33*kappa_y1*l1^3*m*(kappa_x1^2 + kappa_y1^2)^(5/2) - 4.0e33*kappa_y1^3*l1^3*m*(kappa_x1^2 + kappa_y1^2)^(3/2) - 8.0e33*kappa_y1*l1*m*(kappa_x1^2 + kappa_y1^2)^(3/2) - 4.0e33*kappa_x1^2*kappa_y1*l1^3*m*(kappa_x1^2 + kappa_y1^2)^(3/2) - 2.0e33*kappa_y1^3*l1^3*m*cos(l1*(kappa_x1^2 + kappa_y1^2)^(1/2))*(kappa_x1^2 + kappa_y1^2)^(3/2) + 1.3333333333333333333333333333333e33*kappa_x1^6*kappa_y1*l1^3*m*((kappa_x1^2 + kappa_y1^2)/kappa_x1^2)^(1/2) + 8.0e33*kappa_y1*l1*m*cos(l1*(kappa_x1^2 + kappa_y1^2)^(1/2))*(kappa_x1^2 + kappa_y1^2)^(3/2) + 1.3333333333333333333333333333333e33*kappa_x1^2*kappa_y1^5*l1^3*m*((kappa_x1^2 + kappa_y1^2)/kappa_x1^2)^(1/2) + 2.6666666666666666666666666666667e33*kappa_x1^4*kappa_y1^3*l1^3*m*((kappa_x1^2 + kappa_y1^2)/kappa_x1^2)^(1/2) - 2.0e33*kappa_y1*l1^2*m*sin(l1*(kappa_x1^2 + kappa_y1^2)^(1/2))*(kappa_x1^2 + kappa_y1^2)^2 + 1.0e34*kappa_y1^3*l1^2*m*sin(l1*(kappa_x1^2 + kappa_y1^2)^(1/2))*(kappa_x1^2 + kappa_y1^2) + 333333333333333333333333333333333.0*kappa_x1^8*kappa_y1*l1^3*m*r^2*((kappa_x1^2 + kappa_y1^2)/kappa_x1^2)^(1/2) + 1.0e34*kappa_x1^2*kappa_y1*l1^2*m*sin(l1*(kappa_x1^2 + kappa_y1^2)^(1/2))*(kappa_x1^2 + kappa_y1^2) + 4.0e33*kappa_x1^2*kappa_y1*m*sin(l1*(kappa_x1^2 + kappa_y1^2)^(1/2))*((kappa_x1^2 + kappa_y1^2)/kappa_x1^2)^(1/2)*(kappa_x1^2 + kappa_y1^2)^(1/2) + 666666666666666666666666666666677.0*kappa_x1^2*kappa_y1^7*l1^3*m*r^2*((kappa_x1^2 + kappa_y1^2)/kappa_x1^2)^(1/2) + 1.6666666666666666666666666666667e33*kappa_x1^4*kappa_y1^5*l1^3*m*r^2*((kappa_x1^2 + kappa_y1^2)/kappa_x1^2)^(1/2) + 1.3333333333333333333333333333333e33*kappa_x1^6*kappa_y1^3*l1^3*m*r^2*((kappa_x1^2 + kappa_y1^2)/kappa_x1^2)^(1/2) - 2.0e33*kappa_x1^2*kappa_y1*l1^3*m*cos(l1*(kappa_x1^2 + kappa_y1^2)^(1/2))*(kappa_x1^2 + kappa_y1^2)^(3/2) + 500000000000000000000000000000000.0*kappa_x1^2*kappa_y1*m*sin(2.0*l1*(kappa_x1^2 + kappa_y1^2)^(1/2))*((kappa_x1^2 + kappa_y1^2)/kappa_x1^2)^(1/2)*(kappa_x1^2 + kappa_y1^2)^(1/2) - 4.0e33*kappa_x1^4*kappa_y1*l1^2*m*sin(l1*(kappa_x1^2 + kappa_y1^2)^(1/2))*((kappa_x1^2 + kappa_y1^2)/kappa_x1^2)^(1/2)*(kappa_x1^2 + kappa_y1^2)^(1/2) - 2.0e33*kappa_x1^2*kappa_y1*m*r^2*sin(l1*(kappa_x1^2 + kappa_y1^2)^(1/2))*((kappa_x1^2 + kappa_y1^2)/kappa_x1^2)^(1/2)*(kappa_x1^2 + kappa_y1^2)^(3/2) - 500000000000000000000000000000000.0*kappa_x1^4*kappa_y1*m*r^2*sin(l1*(kappa_x1^2 + kappa_y1^2)^(1/2))*((kappa_x1^2 + kappa_y1^2)/kappa_x1^2)^(1/2)*(kappa_x1^2 + kappa_y1^2)^(1/2) - 4.0e33*kappa_x1^2*kappa_y1*l1*m*cos(l1*(kappa_x1^2 + kappa_y1^2)^(1/2))*((kappa_x1^2 + kappa_y1^2)/kappa_x1^2)^(1/2)*(kappa_x1^2 + kappa_y1^2) + 250000000000000000000000000000000.0*kappa_x1^2*kappa_y1*m*r^2*sin(2.0*l1*(kappa_x1^2 + kappa_y1^2)^(1/2))*((kappa_x1^2 + kappa_y1^2)/kappa_x1^2)^(1/2)*(kappa_x1^2 + kappa_y1^2)^(3/2) - 250000000000000000000000000000000.0*kappa_x1^4*kappa_y1*m*r^2*sin(2.0*l1*(kappa_x1^2 + kappa_y1^2)^(1/2))*((kappa_x1^2 + kappa_y1^2)/kappa_x1^2)^(1/2)*(kappa_x1^2 + kappa_y1^2)^(1/2) - 4.0e33*kappa_x1^2*kappa_y1^3*l1^2*m*sin(l1*(kappa_x1^2 + kappa_y1^2)^(1/2))*((kappa_x1^2 + kappa_y1^2)/kappa_x1^2)^(1/2)*(kappa_x1^2 + kappa_y1^2)^(1/2) + 500000000000000000000000000000000.0*kappa_x1^2*kappa_y1^3*m*r^2*sin(l1*(kappa_x1^2 + kappa_y1^2)^(1/2))*((kappa_x1^2 + kappa_y1^2)/kappa_x1^2)^(1/2)*(kappa_x1^2 + kappa_y1^2)^(1/2) - 1.0e33*kappa_x1^2*kappa_y1*l1*m*cos(2.0*l1*(kappa_x1^2 + kappa_y1^2)^(1/2))*((kappa_x1^2 + kappa_y1^2)/kappa_x1^2)^(1/2)*(kappa_x1^2 + kappa_y1^2) - 125000000000000000000000000000000.0*kappa_x1^2*kappa_y1^3*m*r^2*sin(2.0*l1*(kappa_x1^2 + kappa_y1^2)^(1/2))*((kappa_x1^2 + kappa_y1^2)/kappa_x1^2)^(1/2)*(kappa_x1^2 + kappa_y1^2)^(1/2) + 500000000000000000000000000000000.0*kappa_x1^6*kappa_y1*l1^2*m*r^2*sin(l1*(kappa_x1^2 + kappa_y1^2)^(1/2))*((kappa_x1^2 + kappa_y1^2)/kappa_x1^2)^(1/2)*(kappa_x1^2 + kappa_y1^2)^(1/2) + 500000000000000000000000000000000.0*kappa_x1^4*kappa_y1*l1*m*r^2*cos(l1*(kappa_x1^2 + kappa_y1^2)^(1/2))*((kappa_x1^2 + kappa_y1^2)/kappa_x1^2)^(1/2)*(kappa_x1^2 + kappa_y1^2) - 500000000000000000000000000000000.0*kappa_x1^2*kappa_y1^5*l1^2*m*r^2*sin(l1*(kappa_x1^2 + kappa_y1^2)^(1/2))*((kappa_x1^2 + kappa_y1^2)/kappa_x1^2)^(1/2)*(kappa_x1^2 + kappa_y1^2)^(1/2) + 500000000000000000000000000000000.0*kappa_x1^4*kappa_y1*l1*m*r^2*cos(2.0*l1*(kappa_x1^2 + kappa_y1^2)^(1/2))*((kappa_x1^2 + kappa_y1^2)/kappa_x1^2)^(1/2)*(kappa_x1^2 + kappa_y1^2) + 2.0e33*kappa_x1^2*kappa_y1*l1*m*r^2*cos(l1*(kappa_x1^2 + kappa_y1^2)^(1/2))*((kappa_x1^2 + kappa_y1^2)/kappa_x1^2)^(1/2)*(kappa_x1^2 + kappa_y1^2)^2 - 500000000000000000000000000000000.0*kappa_x1^2*kappa_y1^3*l1*m*r^2*cos(l1*(kappa_x1^2 + kappa_y1^2)^(1/2))*((kappa_x1^2 + kappa_y1^2)/kappa_x1^2)^(1/2)*(kappa_x1^2 + kappa_y1^2) - 500000000000000000000000000000000.0*kappa_x1^2*kappa_y1*l1*m*r^2*cos(2.0*l1*(kappa_x1^2 + kappa_y1^2)^(1/2))*((kappa_x1^2 + kappa_y1^2)/kappa_x1^2)^(1/2)*(kappa_x1^2 + kappa_y1^2)^2 + 250000000000000000000000000000000.0*kappa_x1^2*kappa_y1^3*l1*m*r^2*cos(2.0*l1*(kappa_x1^2 + kappa_y1^2)^(1/2))*((kappa_x1^2 + kappa_y1^2)/kappa_x1^2)^(1/2)*(kappa_x1^2 + kappa_y1^2)))/(2000000000000000000000000000000000*kappa_x1*l1^2*((kappa_x1^2 + kappa_y1^2)/kappa_x1^2)^(1/2)*(kappa_x1^2 + kappa_y1^2)^4);
% 
% V(3,1) = (dkappa_y1*(5.3333333333333333333333333333333e33*kappa_y1^6*l1^3*m + 1.0666666666666666666666666666667e34*kappa_x1^2*kappa_y1^4*l1^3*m + 5.3333333333333333333333333333333e33*kappa_x1^4*kappa_y1^2*l1^3*m + 2.6666666666666666666666666666667e33*kappa_y1^8*l1^3*m*r^2 + 1.6e34*kappa_x1^2*m*sin(l1*(kappa_x1^2 + kappa_y1^2)^(1/2))*(kappa_x1^2 + kappa_y1^2)^(1/2) + 3.2e34*kappa_y1^2*m*sin(l1*(kappa_x1^2 + kappa_y1^2)^(1/2))*(kappa_x1^2 + kappa_y1^2)^(1/2) - 2.0e33*kappa_x1^2*m*sin(2.0*l1*(kappa_x1^2 + kappa_y1^2)^(1/2))*(kappa_x1^2 + kappa_y1^2)^(1/2) - 1.6e34*kappa_y1^4*l1^2*m*sin(l1*(kappa_x1^2 + kappa_y1^2)^(1/2))*(kappa_x1^2 + kappa_y1^2)^(1/2) + 8.0e33*kappa_x1^2*m*r^2*sin(l1*(kappa_x1^2 + kappa_y1^2)^(1/2))*(kappa_x1^2 + kappa_y1^2)^(3/2) - 1.6e34*kappa_x1^2*l1*m*cos(l1*(kappa_x1^2 + kappa_y1^2)^(1/2))*(kappa_x1^2 + kappa_y1^2) - 3.2e34*kappa_y1^2*l1*m*cos(l1*(kappa_x1^2 + kappa_y1^2)^(1/2))*(kappa_x1^2 + kappa_y1^2) - 1.0e33*kappa_x1^2*m*r^2*sin(2.0*l1*(kappa_x1^2 + kappa_y1^2)^(1/2))*(kappa_x1^2 + kappa_y1^2)^(3/2) + 1.0e33*kappa_x1^4*m*r^2*sin(2.0*l1*(kappa_x1^2 + kappa_y1^2)^(1/2))*(kappa_x1^2 + kappa_y1^2)^(1/2) + 4.0e33*kappa_x1^2*l1*m*cos(2.0*l1*(kappa_x1^2 + kappa_y1^2)^(1/2))*(kappa_x1^2 + kappa_y1^2) + 6.6666666666666666666666666666667e33*kappa_x1^2*kappa_y1^6*l1^3*m*r^2 + 5.3333333333333333333333333333333e33*kappa_x1^4*kappa_y1^4*l1^3*m*r^2 + 1.3333333333333333333333333333333e33*kappa_x1^6*kappa_y1^2*l1^3*m*r^2 - 1.6e34*kappa_x1^2*kappa_y1^2*l1^2*m*sin(l1*(kappa_x1^2 + kappa_y1^2)^(1/2))*(kappa_x1^2 + kappa_y1^2)^(1/2) - 4.0e33*kappa_x1^2*kappa_y1^2*m*r^2*sin(l1*(kappa_x1^2 + kappa_y1^2)^(1/2))*(kappa_x1^2 + kappa_y1^2)^(1/2) + 500000000000000000000000000000000.0*kappa_x1^2*kappa_y1^2*m*r^2*sin(2.0*l1*(kappa_x1^2 + kappa_y1^2)^(1/2))*(kappa_x1^2 + kappa_y1^2)^(1/2) - 2.0e33*kappa_x1^4*l1*m*r^2*cos(2.0*l1*(kappa_x1^2 + kappa_y1^2)^(1/2))*(kappa_x1^2 + kappa_y1^2) - 8.0e33*kappa_x1^2*l1*m*r^2*cos(l1*(kappa_x1^2 + kappa_y1^2)^(1/2))*(kappa_x1^2 + kappa_y1^2)^2 + 2.0e33*kappa_x1^2*l1*m*r^2*cos(2.0*l1*(kappa_x1^2 + kappa_y1^2)^(1/2))*(kappa_x1^2 + kappa_y1^2)^2 + 4.0e33*kappa_x1^2*kappa_y1^2*l1*m*r^2*cos(l1*(kappa_x1^2 + kappa_y1^2)^(1/2))*(kappa_x1^2 + kappa_y1^2) - 1.0e33*kappa_x1^2*kappa_y1^2*l1*m*r^2*cos(2.0*l1*(kappa_x1^2 + kappa_y1^2)^(1/2))*(kappa_x1^2 + kappa_y1^2) + 4.0e33*kappa_x1^2*kappa_y1^4*l1^2*m*r^2*sin(l1*(kappa_x1^2 + kappa_y1^2)^(1/2))*(kappa_x1^2 + kappa_y1^2)^(1/2) + 4.0e33*kappa_x1^4*kappa_y1^2*l1^2*m*r^2*sin(l1*(kappa_x1^2 + kappa_y1^2)^(1/2))*(kappa_x1^2 + kappa_y1^2)^(1/2)))/(8000000000000000000000000000000000*l1^2*(kappa_x1^2 + kappa_y1^2)^4) + (dl1*(2.6666666666666666666666666666667*kappa_y1^5*l1^3*m*(kappa_x1^2 + kappa_y1^2)^(3/2) - 2.6666666666666666666666666666667*kappa_y1^3*l1^3*m*(kappa_x1^2 + kappa_y1^2)^(5/2) - 20.0*kappa_x1^4*kappa_y1*m*sin(l1*(kappa_x1^2 + kappa_y1^2)^(1/2)) - 20.0*kappa_x1^2*kappa_y1^3*m*sin(l1*(kappa_x1^2 + kappa_y1^2)^(1/2)) + 12.0*kappa_x1^2*kappa_y1^3*l1*m*(kappa_x1^2 + kappa_y1^2)^(1/2) - 1.3333333333333333333333333333333*kappa_x1^2*kappa_y1*l1^3*m*(kappa_x1^2 + kappa_y1^2)^(5/2) + 2.6666666666666666666666666666667*kappa_x1^2*kappa_y1^3*l1^3*m*(kappa_x1^2 + kappa_y1^2)^(3/2) + 4.0*kappa_x1^2*kappa_y1*l1*m*(kappa_x1^2 + kappa_y1^2)^(3/2) + 12.0*kappa_x1^4*kappa_y1*l1*m*(kappa_x1^2 + kappa_y1^2)^(1/2) + 4.0*kappa_x1^4*kappa_y1*l1*m*cos(l1*(kappa_x1^2 + kappa_y1^2)^(1/2))*(kappa_x1^2 + kappa_y1^2)^(1/2) + 4.0*kappa_x1^2*kappa_y1^3*l1*m*cos(l1*(kappa_x1^2 + kappa_y1^2)^(1/2))*(kappa_x1^2 + kappa_y1^2)^(1/2)))/(2*l1*(kappa_x1^2 + kappa_y1^2)^(9/2)) + (dkappa_x1*(4.0e33*kappa_y1^3*l1^3*m*(kappa_x1^2 + kappa_y1^2)^(3/2) - 2.0e33*kappa_y1*l1^3*m*(kappa_x1^2 + kappa_y1^2)^(5/2) + 8.0e33*kappa_y1*l1*m*(kappa_x1^2 + kappa_y1^2)^(3/2) + 4.0e33*kappa_x1^2*kappa_y1*l1^3*m*(kappa_x1^2 + kappa_y1^2)^(3/2) + 2.0e33*kappa_y1^3*l1^3*m*cos(l1*(kappa_x1^2 + kappa_y1^2)^(1/2))*(kappa_x1^2 + kappa_y1^2)^(3/2) + 1.3333333333333333333333333333333e33*kappa_x1^6*kappa_y1*l1^3*m*((kappa_x1^2 + kappa_y1^2)/kappa_x1^2)^(1/2) - 8.0e33*kappa_y1*l1*m*cos(l1*(kappa_x1^2 + kappa_y1^2)^(1/2))*(kappa_x1^2 + kappa_y1^2)^(3/2) + 1.3333333333333333333333333333333e33*kappa_x1^2*kappa_y1^5*l1^3*m*((kappa_x1^2 + kappa_y1^2)/kappa_x1^2)^(1/2) + 2.6666666666666666666666666666667e33*kappa_x1^4*kappa_y1^3*l1^3*m*((kappa_x1^2 + kappa_y1^2)/kappa_x1^2)^(1/2) + 2.0e33*kappa_y1*l1^2*m*sin(l1*(kappa_x1^2 + kappa_y1^2)^(1/2))*(kappa_x1^2 + kappa_y1^2)^2 - 1.0e34*kappa_y1^3*l1^2*m*sin(l1*(kappa_x1^2 + kappa_y1^2)^(1/2))*(kappa_x1^2 + kappa_y1^2) + 333333333333333333333333333333333.0*kappa_x1^8*kappa_y1*l1^3*m*r^2*((kappa_x1^2 + kappa_y1^2)/kappa_x1^2)^(1/2) - 1.0e34*kappa_x1^2*kappa_y1*l1^2*m*sin(l1*(kappa_x1^2 + kappa_y1^2)^(1/2))*(kappa_x1^2 + kappa_y1^2) + 4.0e33*kappa_x1^2*kappa_y1*m*sin(l1*(kappa_x1^2 + kappa_y1^2)^(1/2))*((kappa_x1^2 + kappa_y1^2)/kappa_x1^2)^(1/2)*(kappa_x1^2 + kappa_y1^2)^(1/2) + 666666666666666666666666666666677.0*kappa_x1^2*kappa_y1^7*l1^3*m*r^2*((kappa_x1^2 + kappa_y1^2)/kappa_x1^2)^(1/2) + 1.6666666666666666666666666666667e33*kappa_x1^4*kappa_y1^5*l1^3*m*r^2*((kappa_x1^2 + kappa_y1^2)/kappa_x1^2)^(1/2) + 1.3333333333333333333333333333333e33*kappa_x1^6*kappa_y1^3*l1^3*m*r^2*((kappa_x1^2 + kappa_y1^2)/kappa_x1^2)^(1/2) + 2.0e33*kappa_x1^2*kappa_y1*l1^3*m*cos(l1*(kappa_x1^2 + kappa_y1^2)^(1/2))*(kappa_x1^2 + kappa_y1^2)^(3/2) + 500000000000000000000000000000000.0*kappa_x1^2*kappa_y1*m*sin(2.0*l1*(kappa_x1^2 + kappa_y1^2)^(1/2))*((kappa_x1^2 + kappa_y1^2)/kappa_x1^2)^(1/2)*(kappa_x1^2 + kappa_y1^2)^(1/2) - 4.0e33*kappa_x1^4*kappa_y1*l1^2*m*sin(l1*(kappa_x1^2 + kappa_y1^2)^(1/2))*((kappa_x1^2 + kappa_y1^2)/kappa_x1^2)^(1/2)*(kappa_x1^2 + kappa_y1^2)^(1/2) - 2.0e33*kappa_x1^2*kappa_y1*m*r^2*sin(l1*(kappa_x1^2 + kappa_y1^2)^(1/2))*((kappa_x1^2 + kappa_y1^2)/kappa_x1^2)^(1/2)*(kappa_x1^2 + kappa_y1^2)^(3/2) - 500000000000000000000000000000000.0*kappa_x1^4*kappa_y1*m*r^2*sin(l1*(kappa_x1^2 + kappa_y1^2)^(1/2))*((kappa_x1^2 + kappa_y1^2)/kappa_x1^2)^(1/2)*(kappa_x1^2 + kappa_y1^2)^(1/2) - 4.0e33*kappa_x1^2*kappa_y1*l1*m*cos(l1*(kappa_x1^2 + kappa_y1^2)^(1/2))*((kappa_x1^2 + kappa_y1^2)/kappa_x1^2)^(1/2)*(kappa_x1^2 + kappa_y1^2) + 250000000000000000000000000000000.0*kappa_x1^2*kappa_y1*m*r^2*sin(2.0*l1*(kappa_x1^2 + kappa_y1^2)^(1/2))*((kappa_x1^2 + kappa_y1^2)/kappa_x1^2)^(1/2)*(kappa_x1^2 + kappa_y1^2)^(3/2) - 250000000000000000000000000000000.0*kappa_x1^4*kappa_y1*m*r^2*sin(2.0*l1*(kappa_x1^2 + kappa_y1^2)^(1/2))*((kappa_x1^2 + kappa_y1^2)/kappa_x1^2)^(1/2)*(kappa_x1^2 + kappa_y1^2)^(1/2) - 4.0e33*kappa_x1^2*kappa_y1^3*l1^2*m*sin(l1*(kappa_x1^2 + kappa_y1^2)^(1/2))*((kappa_x1^2 + kappa_y1^2)/kappa_x1^2)^(1/2)*(kappa_x1^2 + kappa_y1^2)^(1/2) + 500000000000000000000000000000000.0*kappa_x1^2*kappa_y1^3*m*r^2*sin(l1*(kappa_x1^2 + kappa_y1^2)^(1/2))*((kappa_x1^2 + kappa_y1^2)/kappa_x1^2)^(1/2)*(kappa_x1^2 + kappa_y1^2)^(1/2) - 1.0e33*kappa_x1^2*kappa_y1*l1*m*cos(2.0*l1*(kappa_x1^2 + kappa_y1^2)^(1/2))*((kappa_x1^2 + kappa_y1^2)/kappa_x1^2)^(1/2)*(kappa_x1^2 + kappa_y1^2) - 125000000000000000000000000000000.0*kappa_x1^2*kappa_y1^3*m*r^2*sin(2.0*l1*(kappa_x1^2 + kappa_y1^2)^(1/2))*((kappa_x1^2 + kappa_y1^2)/kappa_x1^2)^(1/2)*(kappa_x1^2 + kappa_y1^2)^(1/2) + 500000000000000000000000000000000.0*kappa_x1^6*kappa_y1*l1^2*m*r^2*sin(l1*(kappa_x1^2 + kappa_y1^2)^(1/2))*((kappa_x1^2 + kappa_y1^2)/kappa_x1^2)^(1/2)*(kappa_x1^2 + kappa_y1^2)^(1/2) + 500000000000000000000000000000000.0*kappa_x1^4*kappa_y1*l1*m*r^2*cos(l1*(kappa_x1^2 + kappa_y1^2)^(1/2))*((kappa_x1^2 + kappa_y1^2)/kappa_x1^2)^(1/2)*(kappa_x1^2 + kappa_y1^2) - 500000000000000000000000000000000.0*kappa_x1^2*kappa_y1^5*l1^2*m*r^2*sin(l1*(kappa_x1^2 + kappa_y1^2)^(1/2))*((kappa_x1^2 + kappa_y1^2)/kappa_x1^2)^(1/2)*(kappa_x1^2 + kappa_y1^2)^(1/2) + 500000000000000000000000000000000.0*kappa_x1^4*kappa_y1*l1*m*r^2*cos(2.0*l1*(kappa_x1^2 + kappa_y1^2)^(1/2))*((kappa_x1^2 + kappa_y1^2)/kappa_x1^2)^(1/2)*(kappa_x1^2 + kappa_y1^2) + 2.0e33*kappa_x1^2*kappa_y1*l1*m*r^2*cos(l1*(kappa_x1^2 + kappa_y1^2)^(1/2))*((kappa_x1^2 + kappa_y1^2)/kappa_x1^2)^(1/2)*(kappa_x1^2 + kappa_y1^2)^2 - 500000000000000000000000000000000.0*kappa_x1^2*kappa_y1^3*l1*m*r^2*cos(l1*(kappa_x1^2 + kappa_y1^2)^(1/2))*((kappa_x1^2 + kappa_y1^2)/kappa_x1^2)^(1/2)*(kappa_x1^2 + kappa_y1^2) - 500000000000000000000000000000000.0*kappa_x1^2*kappa_y1*l1*m*r^2*cos(2.0*l1*(kappa_x1^2 + kappa_y1^2)^(1/2))*((kappa_x1^2 + kappa_y1^2)/kappa_x1^2)^(1/2)*(kappa_x1^2 + kappa_y1^2)^2 + 250000000000000000000000000000000.0*kappa_x1^2*kappa_y1^3*l1*m*r^2*cos(2.0*l1*(kappa_x1^2 + kappa_y1^2)^(1/2))*((kappa_x1^2 + kappa_y1^2)/kappa_x1^2)^(1/2)*(kappa_x1^2 + kappa_y1^2)))/(2000000000000000000000000000000000*kappa_x1*l1^2*((kappa_x1^2 + kappa_y1^2)/kappa_x1^2)^(1/2)*(kappa_x1^2 + kappa_y1^2)^4);
% V(3,2) = (dl1*(4.0e33*kappa_y1^3*l1^3*m*(kappa_x1^2 + kappa_y1^2)^(3/2) - 2.0e33*kappa_y1*l1^3*m*(kappa_x1^2 + kappa_y1^2)^(5/2) + 8.0e33*kappa_y1*l1*m*(kappa_x1^2 + kappa_y1^2)^(3/2) + 4.0e33*kappa_x1^2*kappa_y1*l1^3*m*(kappa_x1^2 + kappa_y1^2)^(3/2) + 2.0e33*kappa_y1^3*l1^3*m*cos(l1*(kappa_x1^2 + kappa_y1^2)^(1/2))*(kappa_x1^2 + kappa_y1^2)^(3/2) + 1.3333333333333333333333333333333e33*kappa_x1^6*kappa_y1*l1^3*m*((kappa_x1^2 + kappa_y1^2)/kappa_x1^2)^(1/2) - 8.0e33*kappa_y1*l1*m*cos(l1*(kappa_x1^2 + kappa_y1^2)^(1/2))*(kappa_x1^2 + kappa_y1^2)^(3/2) + 1.3333333333333333333333333333333e33*kappa_x1^2*kappa_y1^5*l1^3*m*((kappa_x1^2 + kappa_y1^2)/kappa_x1^2)^(1/2) + 2.6666666666666666666666666666667e33*kappa_x1^4*kappa_y1^3*l1^3*m*((kappa_x1^2 + kappa_y1^2)/kappa_x1^2)^(1/2) + 2.0e33*kappa_y1*l1^2*m*sin(l1*(kappa_x1^2 + kappa_y1^2)^(1/2))*(kappa_x1^2 + kappa_y1^2)^2 - 1.0e34*kappa_y1^3*l1^2*m*sin(l1*(kappa_x1^2 + kappa_y1^2)^(1/2))*(kappa_x1^2 + kappa_y1^2) + 333333333333333333333333333333333.0*kappa_x1^8*kappa_y1*l1^3*m*r^2*((kappa_x1^2 + kappa_y1^2)/kappa_x1^2)^(1/2) - 1.0e34*kappa_x1^2*kappa_y1*l1^2*m*sin(l1*(kappa_x1^2 + kappa_y1^2)^(1/2))*(kappa_x1^2 + kappa_y1^2) + 4.0e33*kappa_x1^2*kappa_y1*m*sin(l1*(kappa_x1^2 + kappa_y1^2)^(1/2))*((kappa_x1^2 + kappa_y1^2)/kappa_x1^2)^(1/2)*(kappa_x1^2 + kappa_y1^2)^(1/2) + 666666666666666666666666666666677.0*kappa_x1^2*kappa_y1^7*l1^3*m*r^2*((kappa_x1^2 + kappa_y1^2)/kappa_x1^2)^(1/2) + 1.6666666666666666666666666666667e33*kappa_x1^4*kappa_y1^5*l1^3*m*r^2*((kappa_x1^2 + kappa_y1^2)/kappa_x1^2)^(1/2) + 1.3333333333333333333333333333333e33*kappa_x1^6*kappa_y1^3*l1^3*m*r^2*((kappa_x1^2 + kappa_y1^2)/kappa_x1^2)^(1/2) + 2.0e33*kappa_x1^2*kappa_y1*l1^3*m*cos(l1*(kappa_x1^2 + kappa_y1^2)^(1/2))*(kappa_x1^2 + kappa_y1^2)^(3/2) + 500000000000000000000000000000000.0*kappa_x1^2*kappa_y1*m*sin(2.0*l1*(kappa_x1^2 + kappa_y1^2)^(1/2))*((kappa_x1^2 + kappa_y1^2)/kappa_x1^2)^(1/2)*(kappa_x1^2 + kappa_y1^2)^(1/2) - 4.0e33*kappa_x1^4*kappa_y1*l1^2*m*sin(l1*(kappa_x1^2 + kappa_y1^2)^(1/2))*((kappa_x1^2 + kappa_y1^2)/kappa_x1^2)^(1/2)*(kappa_x1^2 + kappa_y1^2)^(1/2) - 2.0e33*kappa_x1^2*kappa_y1*m*r^2*sin(l1*(kappa_x1^2 + kappa_y1^2)^(1/2))*((kappa_x1^2 + kappa_y1^2)/kappa_x1^2)^(1/2)*(kappa_x1^2 + kappa_y1^2)^(3/2) - 500000000000000000000000000000000.0*kappa_x1^4*kappa_y1*m*r^2*sin(l1*(kappa_x1^2 + kappa_y1^2)^(1/2))*((kappa_x1^2 + kappa_y1^2)/kappa_x1^2)^(1/2)*(kappa_x1^2 + kappa_y1^2)^(1/2) - 4.0e33*kappa_x1^2*kappa_y1*l1*m*cos(l1*(kappa_x1^2 + kappa_y1^2)^(1/2))*((kappa_x1^2 + kappa_y1^2)/kappa_x1^2)^(1/2)*(kappa_x1^2 + kappa_y1^2) + 250000000000000000000000000000000.0*kappa_x1^2*kappa_y1*m*r^2*sin(2.0*l1*(kappa_x1^2 + kappa_y1^2)^(1/2))*((kappa_x1^2 + kappa_y1^2)/kappa_x1^2)^(1/2)*(kappa_x1^2 + kappa_y1^2)^(3/2) - 250000000000000000000000000000000.0*kappa_x1^4*kappa_y1*m*r^2*sin(2.0*l1*(kappa_x1^2 + kappa_y1^2)^(1/2))*((kappa_x1^2 + kappa_y1^2)/kappa_x1^2)^(1/2)*(kappa_x1^2 + kappa_y1^2)^(1/2) - 4.0e33*kappa_x1^2*kappa_y1^3*l1^2*m*sin(l1*(kappa_x1^2 + kappa_y1^2)^(1/2))*((kappa_x1^2 + kappa_y1^2)/kappa_x1^2)^(1/2)*(kappa_x1^2 + kappa_y1^2)^(1/2) + 500000000000000000000000000000000.0*kappa_x1^2*kappa_y1^3*m*r^2*sin(l1*(kappa_x1^2 + kappa_y1^2)^(1/2))*((kappa_x1^2 + kappa_y1^2)/kappa_x1^2)^(1/2)*(kappa_x1^2 + kappa_y1^2)^(1/2) - 1.0e33*kappa_x1^2*kappa_y1*l1*m*cos(2.0*l1*(kappa_x1^2 + kappa_y1^2)^(1/2))*((kappa_x1^2 + kappa_y1^2)/kappa_x1^2)^(1/2)*(kappa_x1^2 + kappa_y1^2) - 125000000000000000000000000000000.0*kappa_x1^2*kappa_y1^3*m*r^2*sin(2.0*l1*(kappa_x1^2 + kappa_y1^2)^(1/2))*((kappa_x1^2 + kappa_y1^2)/kappa_x1^2)^(1/2)*(kappa_x1^2 + kappa_y1^2)^(1/2) + 500000000000000000000000000000000.0*kappa_x1^6*kappa_y1*l1^2*m*r^2*sin(l1*(kappa_x1^2 + kappa_y1^2)^(1/2))*((kappa_x1^2 + kappa_y1^2)/kappa_x1^2)^(1/2)*(kappa_x1^2 + kappa_y1^2)^(1/2) + 500000000000000000000000000000000.0*kappa_x1^4*kappa_y1*l1*m*r^2*cos(l1*(kappa_x1^2 + kappa_y1^2)^(1/2))*((kappa_x1^2 + kappa_y1^2)/kappa_x1^2)^(1/2)*(kappa_x1^2 + kappa_y1^2) - 500000000000000000000000000000000.0*kappa_x1^2*kappa_y1^5*l1^2*m*r^2*sin(l1*(kappa_x1^2 + kappa_y1^2)^(1/2))*((kappa_x1^2 + kappa_y1^2)/kappa_x1^2)^(1/2)*(kappa_x1^2 + kappa_y1^2)^(1/2) + 500000000000000000000000000000000.0*kappa_x1^4*kappa_y1*l1*m*r^2*cos(2.0*l1*(kappa_x1^2 + kappa_y1^2)^(1/2))*((kappa_x1^2 + kappa_y1^2)/kappa_x1^2)^(1/2)*(kappa_x1^2 + kappa_y1^2) + 2.0e33*kappa_x1^2*kappa_y1*l1*m*r^2*cos(l1*(kappa_x1^2 + kappa_y1^2)^(1/2))*((kappa_x1^2 + kappa_y1^2)/kappa_x1^2)^(1/2)*(kappa_x1^2 + kappa_y1^2)^2 - 500000000000000000000000000000000.0*kappa_x1^2*kappa_y1^3*l1*m*r^2*cos(l1*(kappa_x1^2 + kappa_y1^2)^(1/2))*((kappa_x1^2 + kappa_y1^2)/kappa_x1^2)^(1/2)*(kappa_x1^2 + kappa_y1^2) - 500000000000000000000000000000000.0*kappa_x1^2*kappa_y1*l1*m*r^2*cos(2.0*l1*(kappa_x1^2 + kappa_y1^2)^(1/2))*((kappa_x1^2 + kappa_y1^2)/kappa_x1^2)^(1/2)*(kappa_x1^2 + kappa_y1^2)^2 + 250000000000000000000000000000000.0*kappa_x1^2*kappa_y1^3*l1*m*r^2*cos(2.0*l1*(kappa_x1^2 + kappa_y1^2)^(1/2))*((kappa_x1^2 + kappa_y1^2)/kappa_x1^2)^(1/2)*(kappa_x1^2 + kappa_y1^2)))/(2000000000000000000000000000000000*kappa_x1*l1^2*((kappa_x1^2 + kappa_y1^2)/kappa_x1^2)^(1/2)*(kappa_x1^2 + kappa_y1^2)^4) - (2.5e-33*dkappa_y1*(2.4e33*kappa_x1^5*l1*m + 1.6e33*kappa_x1*m*sin(l1*(kappa_x1^2 + kappa_y1^2)^(1/2))*(kappa_x1^2 + kappa_y1^2)^(3/2) + 1.0666666666666666666666666666667e33*kappa_x1^3*kappa_y1^4*l1^3*m + 533333333333333333333333333333344.0*kappa_x1^5*kappa_y1^2*l1^3*m - 200000000000000000000000000000000.0*kappa_x1*m*sin(2.0*l1*(kappa_x1^2 + kappa_y1^2)^(1/2))*(kappa_x1^2 + kappa_y1^2)^(3/2) + 3.6e33*kappa_x1*kappa_y1^4*l1*m - 5.6e33*kappa_x1^3*m*sin(l1*(kappa_x1^2 + kappa_y1^2)^(1/2))*(kappa_x1^2 + kappa_y1^2)^(1/2) + 800000000000000000000000000000000.0*kappa_x1^5*l1*m*cos(l1*(kappa_x1^2 + kappa_y1^2)^(1/2)) + 700000000000000000000000000000000.0*kappa_x1^3*m*sin(2.0*l1*(kappa_x1^2 + kappa_y1^2)^(1/2))*(kappa_x1^2 + kappa_y1^2)^(1/2) - 200000000000000000000000000000000.0*kappa_x1^5*l1*m*cos(2.0*l1*(kappa_x1^2 + kappa_y1^2)^(1/2)) + 6.0e33*kappa_x1^3*kappa_y1^2*l1*m + 533333333333333333333333333333344.0*kappa_x1*kappa_y1^6*l1^3*m + 800000000000000000000000000000000.0*kappa_x1^7*l1*m*r^2 - 100000000000000000000000000000000.0*kappa_x1*m*r^2*sin(2.0*l1*(kappa_x1^2 + kappa_y1^2)^(1/2))*(kappa_x1^2 + kappa_y1^2)^(5/2) - 700000000000000000000000000000000.0*kappa_x1*kappa_y1^6*l1*m*r^2 - 2.0e33*kappa_x1^3*m*r^2*sin(l1*(kappa_x1^2 + kappa_y1^2)^(1/2))*(kappa_x1^2 + kappa_y1^2)^(3/2) + 7.2e33*kappa_x1^3*kappa_y1^2*l1*m*cos(l1*(kappa_x1^2 + kappa_y1^2)^(1/2)) + 400000000000000000000000000000000.0*kappa_x1^7*l1*m*r^2*cos(l1*(kappa_x1^2 + kappa_y1^2)^(1/2)) + 450000000000000000000000000000000.0*kappa_x1^3*m*r^2*sin(2.0*l1*(kappa_x1^2 + kappa_y1^2)^(1/2))*(kappa_x1^2 + kappa_y1^2)^(3/2) - 350000000000000000000000000000000.0*kappa_x1^5*m*r^2*sin(2.0*l1*(kappa_x1^2 + kappa_y1^2)^(1/2))*(kappa_x1^2 + kappa_y1^2)^(1/2) - 200000000000000000000000000000000.0*kappa_x1^3*kappa_y1^2*l1*m*cos(2.0*l1*(kappa_x1^2 + kappa_y1^2)^(1/2)) - 900000000000000000000000000000000.0*kappa_x1^3*kappa_y1^4*l1*m*r^2 + 600000000000000000000000000000000.0*kappa_x1^5*kappa_y1^2*l1*m*r^2 + 200000000000000000000000000000000.0*kappa_x1*kappa_y1^8*l1^3*m*r^2 - 1.12e34*kappa_x1*kappa_y1^2*m*sin(l1*(kappa_x1^2 + kappa_y1^2)^(1/2))*(kappa_x1^2 + kappa_y1^2)^(1/2) + 800000000000000000000000000000000.0*kappa_x1*m*r^2*sin(l1*(kappa_x1^2 + kappa_y1^2)^(1/2))*(kappa_x1^2 + kappa_y1^2)^(5/2) + 6.4e33*kappa_x1*kappa_y1^4*l1*m*cos(l1*(kappa_x1^2 + kappa_y1^2)^(1/2)) + 466666666666666666666666666666677.0*kappa_x1^3*kappa_y1^6*l1^3*m*r^2 + 333333333333333333333333333333344.0*kappa_x1^5*kappa_y1^4*l1^3*m*r^2 + 66666666666666666666666666666667.0*kappa_x1^7*kappa_y1^2*l1^3*m*r^2 + 800000000000000000000000000000000.0*kappa_x1^3*kappa_y1^2*l1^2*m*sin(l1*(kappa_x1^2 + kappa_y1^2)^(1/2))*(kappa_x1^2 + kappa_y1^2)^(1/2) + 1.4e33*kappa_x1^3*kappa_y1^2*m*r^2*sin(l1*(kappa_x1^2 + kappa_y1^2)^(1/2))*(kappa_x1^2 + kappa_y1^2)^(1/2) - 200000000000000000000000000000000.0*kappa_x1^3*kappa_y1^4*l1*m*r^2*cos(l1*(kappa_x1^2 + kappa_y1^2)^(1/2)) - 200000000000000000000000000000000.0*kappa_x1^5*kappa_y1^2*l1*m*r^2*cos(l1*(kappa_x1^2 + kappa_y1^2)^(1/2)) - 175000000000000000000000000000000.0*kappa_x1^3*kappa_y1^2*m*r^2*sin(2.0*l1*(kappa_x1^2 + kappa_y1^2)^(1/2))*(kappa_x1^2 + kappa_y1^2)^(1/2) - 50000000000000000000000000000000.0*kappa_x1^3*kappa_y1^4*l1*m*r^2*cos(2.0*l1*(kappa_x1^2 + kappa_y1^2)^(1/2)) - 50000000000000000000000000000000.0*kappa_x1^5*kappa_y1^2*l1*m*r^2*cos(2.0*l1*(kappa_x1^2 + kappa_y1^2)^(1/2)) + 800000000000000000000000000000000.0*kappa_x1*kappa_y1^4*l1^2*m*sin(l1*(kappa_x1^2 + kappa_y1^2)^(1/2))*(kappa_x1^2 + kappa_y1^2)^(1/2) - 400000000000000000000000000000000.0*kappa_x1*kappa_y1^2*m*r^2*sin(l1*(kappa_x1^2 + kappa_y1^2)^(1/2))*(kappa_x1^2 + kappa_y1^2)^(3/2) + 400000000000000000000000000000000.0*kappa_x1*kappa_y1^6*l1*m*r^2*cos(l1*(kappa_x1^2 + kappa_y1^2)^(1/2)) + 50000000000000000000000000000000.0*kappa_x1*kappa_y1^2*m*r^2*sin(2.0*l1*(kappa_x1^2 + kappa_y1^2)^(1/2))*(kappa_x1^2 + kappa_y1^2)^(3/2) - 200000000000000000000000000000000.0*kappa_x1^3*kappa_y1^4*l1^2*m*r^2*sin(l1*(kappa_x1^2 + kappa_y1^2)^(1/2))*(kappa_x1^2 + kappa_y1^2)^(1/2) - 200000000000000000000000000000000.0*kappa_x1^5*kappa_y1^2*l1^2*m*r^2*sin(l1*(kappa_x1^2 + kappa_y1^2)^(1/2))*(kappa_x1^2 + kappa_y1^2)^(1/2)))/(l1*(kappa_x1^2 + kappa_y1^2)^5) - (1.25e-33*dkappa_x1*(533333333333333333333333333333333.0*kappa_x1^4*kappa_y1^3*l1^3*m - 533333333333333333333333333333333.0*kappa_y1^7*l1^3*m - 533333333333333333333333333333322.0*kappa_x1^2*kappa_y1^5*l1^3*m - 5.6e33*kappa_y1^5*l1*m - 266666666666666666666666666666677.0*kappa_y1^9*l1^3*m*r^2 + 800000000000000000000000000000000.0*kappa_y1*m*sin(2.0*l1*(kappa_x1^2 + kappa_y1^2)^(1/2))*(kappa_x1^2 + kappa_y1^2)^(3/2) - 3.2e33*kappa_x1^4*kappa_y1*l1*m + 1.12e34*kappa_y1^3*m*sin(l1*(kappa_x1^2 + kappa_y1^2)^(1/2))*(kappa_x1^2 + kappa_y1^2)^(1/2) - 4.8e33*kappa_y1^5*l1*m*cos(l1*(kappa_x1^2 + kappa_y1^2)^(1/2)) - 1.4e33*kappa_y1^3*m*sin(2.0*l1*(kappa_x1^2 + kappa_y1^2)^(1/2))*(kappa_x1^2 + kappa_y1^2)^(1/2) + 400000000000000000000000000000000.0*kappa_y1^5*l1*m*cos(2.0*l1*(kappa_x1^2 + kappa_y1^2)^(1/2)) - 8.8e33*kappa_x1^2*kappa_y1^3*l1*m + 533333333333333333333333333333344.0*kappa_x1^6*kappa_y1*l1^3*m - 2.8e33*kappa_x1^2*kappa_y1*m*sin(2.0*l1*(kappa_x1^2 + kappa_y1^2)^(1/2))*(kappa_x1^2 + kappa_y1^2)^(1/2) + 400000000000000000000000000000000.0*kappa_y1*m*r^2*sin(2.0*l1*(kappa_x1^2 + kappa_y1^2)^(1/2))*(kappa_x1^2 + kappa_y1^2)^(5/2) + 800000000000000000000000000000000.0*kappa_x1^4*kappa_y1*l1*m*cos(2.0*l1*(kappa_x1^2 + kappa_y1^2)^(1/2)) - 3.2e33*kappa_x1^6*kappa_y1*l1*m*r^2 + 4.4e33*kappa_y1^3*m*r^2*sin(l1*(kappa_x1^2 + kappa_y1^2)^(1/2))*(kappa_x1^2 + kappa_y1^2)^(3/2) + 1.6e33*kappa_x1^2*kappa_y1^3*l1*m*cos(l1*(kappa_x1^2 + kappa_y1^2)^(1/2)) - 1.2e33*kappa_y1^7*l1*m*r^2*cos(l1*(kappa_x1^2 + kappa_y1^2)^(1/2)) - 800000000000000000000000000000000.0*kappa_y1^3*m*r^2*sin(2.0*l1*(kappa_x1^2 + kappa_y1^2)^(1/2))*(kappa_x1^2 + kappa_y1^2)^(3/2) + 350000000000000000000000000000000.0*kappa_y1^5*m*r^2*sin(2.0*l1*(kappa_x1^2 + kappa_y1^2)^(1/2))*(kappa_x1^2 + kappa_y1^2)^(1/2) + 1.2e33*kappa_x1^2*kappa_y1^3*l1*m*cos(2.0*l1*(kappa_x1^2 + kappa_y1^2)^(1/2)) + 100000000000000000000000000000000.0*kappa_y1^7*l1*m*r^2*cos(2.0*l1*(kappa_x1^2 + kappa_y1^2)^(1/2)) - 2.6e33*kappa_x1^2*kappa_y1^5*l1*m*r^2 - 5.8e33*kappa_x1^4*kappa_y1^3*l1*m*r^2 + 133333333333333333333333333333333.0*kappa_x1^8*kappa_y1*l1^3*m*r^2 - 3.2e33*kappa_y1*m*r^2*sin(l1*(kappa_x1^2 + kappa_y1^2)^(1/2))*(kappa_x1^2 + kappa_y1^2)^(5/2) + 6.4e33*kappa_x1^4*kappa_y1*l1*m*cos(l1*(kappa_x1^2 + kappa_y1^2)^(1/2)) - 400000000000000000000000000000000.0*kappa_x1^2*kappa_y1^7*l1^3*m*r^2 + 133333333333333333333333333333333.0*kappa_x1^4*kappa_y1^5*l1^3*m*r^2 + 400000000000000000000000000000000.0*kappa_x1^6*kappa_y1^3*l1^3*m*r^2 + 1.6e33*kappa_x1^2*kappa_y1^3*l1^2*m*sin(l1*(kappa_x1^2 + kappa_y1^2)^(1/2))*(kappa_x1^2 + kappa_y1^2)^(1/2) - 2.0e33*kappa_x1^2*kappa_y1^5*l1*m*r^2*cos(l1*(kappa_x1^2 + kappa_y1^2)^(1/2)) - 3.2e33*kappa_x1^4*kappa_y1^3*l1*m*r^2*cos(l1*(kappa_x1^2 + kappa_y1^2)^(1/2)) + 1.4e33*kappa_x1^2*kappa_y1^3*m*r^2*sin(2.0*l1*(kappa_x1^2 + kappa_y1^2)^(1/2))*(kappa_x1^2 + kappa_y1^2)^(1/2) + 300000000000000000000000000000000.0*kappa_x1^2*kappa_y1^5*l1*m*r^2*cos(2.0*l1*(kappa_x1^2 + kappa_y1^2)^(1/2)) + 200000000000000000000000000000000.0*kappa_x1^4*kappa_y1^3*l1*m*r^2*cos(2.0*l1*(kappa_x1^2 + kappa_y1^2)^(1/2)) + 1.6e33*kappa_x1^4*kappa_y1*l1^2*m*sin(l1*(kappa_x1^2 + kappa_y1^2)^(1/2))*(kappa_x1^2 + kappa_y1^2)^(1/2) + 6.0e33*kappa_x1^2*kappa_y1*m*r^2*sin(l1*(kappa_x1^2 + kappa_y1^2)^(1/2))*(kappa_x1^2 + kappa_y1^2)^(3/2) + 2.8e33*kappa_x1^4*kappa_y1*m*r^2*sin(l1*(kappa_x1^2 + kappa_y1^2)^(1/2))*(kappa_x1^2 + kappa_y1^2)^(1/2) - 2.4e33*kappa_x1^6*kappa_y1*l1*m*r^2*cos(l1*(kappa_x1^2 + kappa_y1^2)^(1/2)) - 1.8e33*kappa_x1^2*kappa_y1*m*r^2*sin(2.0*l1*(kappa_x1^2 + kappa_y1^2)^(1/2))*(kappa_x1^2 + kappa_y1^2)^(3/2) + 1.4e33*kappa_x1^4*kappa_y1*m*r^2*sin(2.0*l1*(kappa_x1^2 + kappa_y1^2)^(1/2))*(kappa_x1^2 + kappa_y1^2)^(1/2) - 400000000000000000000000000000000.0*kappa_x1^6*kappa_y1*l1^2*m*r^2*sin(l1*(kappa_x1^2 + kappa_y1^2)^(1/2))*(kappa_x1^2 + kappa_y1^2)^(1/2) - 400000000000000000000000000000000.0*kappa_x1^4*kappa_y1^3*l1^2*m*r^2*sin(l1*(kappa_x1^2 + kappa_y1^2)^(1/2))*(kappa_x1^2 + kappa_y1^2)^(1/2)))/(l1*(kappa_x1^2 + kappa_y1^2)^5);
% V(3,3) = (dl1*(5.3333333333333333333333333333333e33*kappa_y1^6*l1^3*m + 1.0666666666666666666666666666667e34*kappa_x1^2*kappa_y1^4*l1^3*m + 5.3333333333333333333333333333333e33*kappa_x1^4*kappa_y1^2*l1^3*m + 2.6666666666666666666666666666667e33*kappa_y1^8*l1^3*m*r^2 + 1.6e34*kappa_x1^2*m*sin(l1*(kappa_x1^2 + kappa_y1^2)^(1/2))*(kappa_x1^2 + kappa_y1^2)^(1/2) + 3.2e34*kappa_y1^2*m*sin(l1*(kappa_x1^2 + kappa_y1^2)^(1/2))*(kappa_x1^2 + kappa_y1^2)^(1/2) - 2.0e33*kappa_x1^2*m*sin(2.0*l1*(kappa_x1^2 + kappa_y1^2)^(1/2))*(kappa_x1^2 + kappa_y1^2)^(1/2) - 1.6e34*kappa_y1^4*l1^2*m*sin(l1*(kappa_x1^2 + kappa_y1^2)^(1/2))*(kappa_x1^2 + kappa_y1^2)^(1/2) + 8.0e33*kappa_x1^2*m*r^2*sin(l1*(kappa_x1^2 + kappa_y1^2)^(1/2))*(kappa_x1^2 + kappa_y1^2)^(3/2) - 1.6e34*kappa_x1^2*l1*m*cos(l1*(kappa_x1^2 + kappa_y1^2)^(1/2))*(kappa_x1^2 + kappa_y1^2) - 3.2e34*kappa_y1^2*l1*m*cos(l1*(kappa_x1^2 + kappa_y1^2)^(1/2))*(kappa_x1^2 + kappa_y1^2) - 1.0e33*kappa_x1^2*m*r^2*sin(2.0*l1*(kappa_x1^2 + kappa_y1^2)^(1/2))*(kappa_x1^2 + kappa_y1^2)^(3/2) + 1.0e33*kappa_x1^4*m*r^2*sin(2.0*l1*(kappa_x1^2 + kappa_y1^2)^(1/2))*(kappa_x1^2 + kappa_y1^2)^(1/2) + 4.0e33*kappa_x1^2*l1*m*cos(2.0*l1*(kappa_x1^2 + kappa_y1^2)^(1/2))*(kappa_x1^2 + kappa_y1^2) + 6.6666666666666666666666666666667e33*kappa_x1^2*kappa_y1^6*l1^3*m*r^2 + 5.3333333333333333333333333333333e33*kappa_x1^4*kappa_y1^4*l1^3*m*r^2 + 1.3333333333333333333333333333333e33*kappa_x1^6*kappa_y1^2*l1^3*m*r^2 - 1.6e34*kappa_x1^2*kappa_y1^2*l1^2*m*sin(l1*(kappa_x1^2 + kappa_y1^2)^(1/2))*(kappa_x1^2 + kappa_y1^2)^(1/2) - 4.0e33*kappa_x1^2*kappa_y1^2*m*r^2*sin(l1*(kappa_x1^2 + kappa_y1^2)^(1/2))*(kappa_x1^2 + kappa_y1^2)^(1/2) + 500000000000000000000000000000000.0*kappa_x1^2*kappa_y1^2*m*r^2*sin(2.0*l1*(kappa_x1^2 + kappa_y1^2)^(1/2))*(kappa_x1^2 + kappa_y1^2)^(1/2) - 2.0e33*kappa_x1^4*l1*m*r^2*cos(2.0*l1*(kappa_x1^2 + kappa_y1^2)^(1/2))*(kappa_x1^2 + kappa_y1^2) - 8.0e33*kappa_x1^2*l1*m*r^2*cos(l1*(kappa_x1^2 + kappa_y1^2)^(1/2))*(kappa_x1^2 + kappa_y1^2)^2 + 2.0e33*kappa_x1^2*l1*m*r^2*cos(2.0*l1*(kappa_x1^2 + kappa_y1^2)^(1/2))*(kappa_x1^2 + kappa_y1^2)^2 + 4.0e33*kappa_x1^2*kappa_y1^2*l1*m*r^2*cos(l1*(kappa_x1^2 + kappa_y1^2)^(1/2))*(kappa_x1^2 + kappa_y1^2) - 1.0e33*kappa_x1^2*kappa_y1^2*l1*m*r^2*cos(2.0*l1*(kappa_x1^2 + kappa_y1^2)^(1/2))*(kappa_x1^2 + kappa_y1^2) + 4.0e33*kappa_x1^2*kappa_y1^4*l1^2*m*r^2*sin(l1*(kappa_x1^2 + kappa_y1^2)^(1/2))*(kappa_x1^2 + kappa_y1^2)^(1/2) + 4.0e33*kappa_x1^4*kappa_y1^2*l1^2*m*r^2*sin(l1*(kappa_x1^2 + kappa_y1^2)^(1/2))*(kappa_x1^2 + kappa_y1^2)^(1/2)))/(8000000000000000000000000000000000*l1^2*(kappa_x1^2 + kappa_y1^2)^4) + (dkappa_y1*(533333333333333333333333333333333.0*kappa_x1^4*kappa_y1^3*l1^3*m - 533333333333333333333333333333333.0*kappa_y1^7*l1^3*m - 6.4e33*kappa_y1*m*sin(l1*(kappa_x1^2 + kappa_y1^2)^(1/2))*(kappa_x1^2 + kappa_y1^2)^(3/2) - 533333333333333333333333333333333.0*kappa_x1^2*kappa_y1^5*l1^3*m - 6.4e33*kappa_y1^5*l1*m - 4.0e33*kappa_x1^4*kappa_y1*l1*m + 2.24e34*kappa_y1^3*m*sin(l1*(kappa_x1^2 + kappa_y1^2)^(1/2))*(kappa_x1^2 + kappa_y1^2)^(1/2) - 9.6e33*kappa_y1^5*l1*m*cos(l1*(kappa_x1^2 + kappa_y1^2)^(1/2)) - 1.04e34*kappa_x1^2*kappa_y1^3*l1*m + 533333333333333333333333333333333.0*kappa_x1^6*kappa_y1*l1^3*m - 1.4e33*kappa_x1^2*kappa_y1*m*sin(2.0*l1*(kappa_x1^2 + kappa_y1^2)^(1/2))*(kappa_x1^2 + kappa_y1^2)^(1/2) + 400000000000000000000000000000000.0*kappa_x1^4*kappa_y1*l1*m*cos(2.0*l1*(kappa_x1^2 + kappa_y1^2)^(1/2)) - 3.4e33*kappa_x1^6*kappa_y1*l1*m*r^2 - 1.6e33*kappa_y1^5*l1^2*m*sin(l1*(kappa_x1^2 + kappa_y1^2)^(1/2))*(kappa_x1^2 + kappa_y1^2)^(1/2) - 8.0e33*kappa_x1^2*kappa_y1^3*l1*m*cos(l1*(kappa_x1^2 + kappa_y1^2)^(1/2)) + 400000000000000000000000000000000.0*kappa_x1^2*kappa_y1^3*l1*m*cos(2.0*l1*(kappa_x1^2 + kappa_y1^2)^(1/2)) - 2.8e33*kappa_x1^2*kappa_y1^5*l1*m*r^2 - 6.2e33*kappa_x1^4*kappa_y1^3*l1*m*r^2 + 133333333333333333333333333333333.0*kappa_x1^8*kappa_y1*l1^3*m*r^2 + 1.12e34*kappa_x1^2*kappa_y1*m*sin(l1*(kappa_x1^2 + kappa_y1^2)^(1/2))*(kappa_x1^2 + kappa_y1^2)^(1/2) + 1.6e33*kappa_x1^4*kappa_y1*l1*m*cos(l1*(kappa_x1^2 + kappa_y1^2)^(1/2)) + 399999999999999999999999999999999.0*kappa_x1^2*kappa_y1^7*l1^3*m*r^2 + 933333333333333333333333333333333.0*kappa_x1^4*kappa_y1^5*l1^3*m*r^2 + 666666666666666666666666666666677.0*kappa_x1^6*kappa_y1^3*l1^3*m*r^2 - 1.6e33*kappa_x1^2*kappa_y1^3*l1^2*m*sin(l1*(kappa_x1^2 + kappa_y1^2)^(1/2))*(kappa_x1^2 + kappa_y1^2)^(1/2) - 2.8e33*kappa_x1^2*kappa_y1^3*m*r^2*sin(l1*(kappa_x1^2 + kappa_y1^2)^(1/2))*(kappa_x1^2 + kappa_y1^2)^(1/2) + 1.2e33*kappa_x1^2*kappa_y1^5*l1*m*r^2*cos(l1*(kappa_x1^2 + kappa_y1^2)^(1/2)) - 400000000000000000000000000000000.0*kappa_x1^4*kappa_y1^3*l1*m*r^2*cos(l1*(kappa_x1^2 + kappa_y1^2)^(1/2)) + 350000000000000000000000000000000.0*kappa_x1^2*kappa_y1^3*m*r^2*sin(2.0*l1*(kappa_x1^2 + kappa_y1^2)^(1/2))*(kappa_x1^2 + kappa_y1^2)^(1/2) + 100000000000000000000000000000000.0*kappa_x1^2*kappa_y1^5*l1*m*r^2*cos(2.0*l1*(kappa_x1^2 + kappa_y1^2)^(1/2)) + 100000000000000000000000000000000.0*kappa_x1^4*kappa_y1^3*l1*m*r^2*cos(2.0*l1*(kappa_x1^2 + kappa_y1^2)^(1/2)) + 4.8e33*kappa_x1^2*kappa_y1*m*r^2*sin(l1*(kappa_x1^2 + kappa_y1^2)^(1/2))*(kappa_x1^2 + kappa_y1^2)^(3/2) - 1.6e33*kappa_x1^6*kappa_y1*l1*m*r^2*cos(l1*(kappa_x1^2 + kappa_y1^2)^(1/2)) - 600000000000000000000000000000000.0*kappa_x1^2*kappa_y1*m*r^2*sin(2.0*l1*(kappa_x1^2 + kappa_y1^2)^(1/2))*(kappa_x1^2 + kappa_y1^2)^(3/2) + 700000000000000000000000000000000.0*kappa_x1^4*kappa_y1*m*r^2*sin(2.0*l1*(kappa_x1^2 + kappa_y1^2)^(1/2))*(kappa_x1^2 + kappa_y1^2)^(1/2) + 400000000000000000000000000000000.0*kappa_x1^2*kappa_y1^5*l1^2*m*r^2*sin(l1*(kappa_x1^2 + kappa_y1^2)^(1/2))*(kappa_x1^2 + kappa_y1^2)^(1/2) + 400000000000000000000000000000000.0*kappa_x1^4*kappa_y1^3*l1^2*m*r^2*sin(l1*(kappa_x1^2 + kappa_y1^2)^(1/2))*(kappa_x1^2 + kappa_y1^2)^(1/2)))/(800000000000000000000000000000000*l1*(kappa_x1^2 + kappa_y1^2)^5) - (2.5e-33*dkappa_x1*(2.4e33*kappa_x1^5*l1*m + 1.6e33*kappa_x1*m*sin(l1*(kappa_x1^2 + kappa_y1^2)^(1/2))*(kappa_x1^2 + kappa_y1^2)^(3/2) + 1.0666666666666666666666666666667e33*kappa_x1^3*kappa_y1^4*l1^3*m + 533333333333333333333333333333344.0*kappa_x1^5*kappa_y1^2*l1^3*m - 200000000000000000000000000000000.0*kappa_x1*m*sin(2.0*l1*(kappa_x1^2 + kappa_y1^2)^(1/2))*(kappa_x1^2 + kappa_y1^2)^(3/2) + 3.6e33*kappa_x1*kappa_y1^4*l1*m - 5.6e33*kappa_x1^3*m*sin(l1*(kappa_x1^2 + kappa_y1^2)^(1/2))*(kappa_x1^2 + kappa_y1^2)^(1/2) + 800000000000000000000000000000000.0*kappa_x1^5*l1*m*cos(l1*(kappa_x1^2 + kappa_y1^2)^(1/2)) + 700000000000000000000000000000000.0*kappa_x1^3*m*sin(2.0*l1*(kappa_x1^2 + kappa_y1^2)^(1/2))*(kappa_x1^2 + kappa_y1^2)^(1/2) - 200000000000000000000000000000000.0*kappa_x1^5*l1*m*cos(2.0*l1*(kappa_x1^2 + kappa_y1^2)^(1/2)) + 6.0e33*kappa_x1^3*kappa_y1^2*l1*m + 533333333333333333333333333333344.0*kappa_x1*kappa_y1^6*l1^3*m + 800000000000000000000000000000000.0*kappa_x1^7*l1*m*r^2 - 100000000000000000000000000000000.0*kappa_x1*m*r^2*sin(2.0*l1*(kappa_x1^2 + kappa_y1^2)^(1/2))*(kappa_x1^2 + kappa_y1^2)^(5/2) - 700000000000000000000000000000000.0*kappa_x1*kappa_y1^6*l1*m*r^2 - 2.0e33*kappa_x1^3*m*r^2*sin(l1*(kappa_x1^2 + kappa_y1^2)^(1/2))*(kappa_x1^2 + kappa_y1^2)^(3/2) + 7.2e33*kappa_x1^3*kappa_y1^2*l1*m*cos(l1*(kappa_x1^2 + kappa_y1^2)^(1/2)) + 400000000000000000000000000000000.0*kappa_x1^7*l1*m*r^2*cos(l1*(kappa_x1^2 + kappa_y1^2)^(1/2)) + 450000000000000000000000000000000.0*kappa_x1^3*m*r^2*sin(2.0*l1*(kappa_x1^2 + kappa_y1^2)^(1/2))*(kappa_x1^2 + kappa_y1^2)^(3/2) - 350000000000000000000000000000000.0*kappa_x1^5*m*r^2*sin(2.0*l1*(kappa_x1^2 + kappa_y1^2)^(1/2))*(kappa_x1^2 + kappa_y1^2)^(1/2) - 200000000000000000000000000000000.0*kappa_x1^3*kappa_y1^2*l1*m*cos(2.0*l1*(kappa_x1^2 + kappa_y1^2)^(1/2)) - 900000000000000000000000000000000.0*kappa_x1^3*kappa_y1^4*l1*m*r^2 + 600000000000000000000000000000000.0*kappa_x1^5*kappa_y1^2*l1*m*r^2 + 200000000000000000000000000000000.0*kappa_x1*kappa_y1^8*l1^3*m*r^2 - 1.12e34*kappa_x1*kappa_y1^2*m*sin(l1*(kappa_x1^2 + kappa_y1^2)^(1/2))*(kappa_x1^2 + kappa_y1^2)^(1/2) + 800000000000000000000000000000000.0*kappa_x1*m*r^2*sin(l1*(kappa_x1^2 + kappa_y1^2)^(1/2))*(kappa_x1^2 + kappa_y1^2)^(5/2) + 6.4e33*kappa_x1*kappa_y1^4*l1*m*cos(l1*(kappa_x1^2 + kappa_y1^2)^(1/2)) + 466666666666666666666666666666677.0*kappa_x1^3*kappa_y1^6*l1^3*m*r^2 + 333333333333333333333333333333344.0*kappa_x1^5*kappa_y1^4*l1^3*m*r^2 + 66666666666666666666666666666667.0*kappa_x1^7*kappa_y1^2*l1^3*m*r^2 + 800000000000000000000000000000000.0*kappa_x1^3*kappa_y1^2*l1^2*m*sin(l1*(kappa_x1^2 + kappa_y1^2)^(1/2))*(kappa_x1^2 + kappa_y1^2)^(1/2) + 1.4e33*kappa_x1^3*kappa_y1^2*m*r^2*sin(l1*(kappa_x1^2 + kappa_y1^2)^(1/2))*(kappa_x1^2 + kappa_y1^2)^(1/2) - 200000000000000000000000000000000.0*kappa_x1^3*kappa_y1^4*l1*m*r^2*cos(l1*(kappa_x1^2 + kappa_y1^2)^(1/2)) - 200000000000000000000000000000000.0*kappa_x1^5*kappa_y1^2*l1*m*r^2*cos(l1*(kappa_x1^2 + kappa_y1^2)^(1/2)) - 175000000000000000000000000000000.0*kappa_x1^3*kappa_y1^2*m*r^2*sin(2.0*l1*(kappa_x1^2 + kappa_y1^2)^(1/2))*(kappa_x1^2 + kappa_y1^2)^(1/2) - 50000000000000000000000000000000.0*kappa_x1^3*kappa_y1^4*l1*m*r^2*cos(2.0*l1*(kappa_x1^2 + kappa_y1^2)^(1/2)) - 50000000000000000000000000000000.0*kappa_x1^5*kappa_y1^2*l1*m*r^2*cos(2.0*l1*(kappa_x1^2 + kappa_y1^2)^(1/2)) + 800000000000000000000000000000000.0*kappa_x1*kappa_y1^4*l1^2*m*sin(l1*(kappa_x1^2 + kappa_y1^2)^(1/2))*(kappa_x1^2 + kappa_y1^2)^(1/2) - 400000000000000000000000000000000.0*kappa_x1*kappa_y1^2*m*r^2*sin(l1*(kappa_x1^2 + kappa_y1^2)^(1/2))*(kappa_x1^2 + kappa_y1^2)^(3/2) + 400000000000000000000000000000000.0*kappa_x1*kappa_y1^6*l1*m*r^2*cos(l1*(kappa_x1^2 + kappa_y1^2)^(1/2)) + 50000000000000000000000000000000.0*kappa_x1*kappa_y1^2*m*r^2*sin(2.0*l1*(kappa_x1^2 + kappa_y1^2)^(1/2))*(kappa_x1^2 + kappa_y1^2)^(3/2) - 200000000000000000000000000000000.0*kappa_x1^3*kappa_y1^4*l1^2*m*r^2*sin(l1*(kappa_x1^2 + kappa_y1^2)^(1/2))*(kappa_x1^2 + kappa_y1^2)^(1/2) - 200000000000000000000000000000000.0*kappa_x1^5*kappa_y1^2*l1^2*m*r^2*sin(l1*(kappa_x1^2 + kappa_y1^2)^(1/2))*(kappa_x1^2 + kappa_y1^2)^(1/2)))/(l1*(kappa_x1^2 + kappa_y1^2)^5);

V(1,1) = (dl1*(4.0*m*sin(l1*(kappa_x1^2 + kappa_y1^2)^(1/2)) - 4.0*l1*m*cos(l1*(kappa_x1^2 + kappa_y1^2)^(1/2))*(kappa_x1^2 + kappa_y1^2)^(1/2)))/(2*l1^2*(kappa_x1^2 + kappa_y1^2)^(3/2)) - (2.0*dkappa_x1*kappa_x1*m*(3.0*kappa_x1^2*l1*(kappa_x1^2 + kappa_y1^2)^(1/2) - 3.0*kappa_x1^2*sin(l1*(kappa_x1^2 + kappa_y1^2)^(1/2)) - 3.0*kappa_y1^2*sin(l1*(kappa_x1^2 + kappa_y1^2)^(1/2)) - 1.0*l1*(kappa_x1^2 + kappa_y1^2)^(3/2) + 3.0*kappa_y1^2*l1*(kappa_x1^2 + kappa_y1^2)^(1/2) + kappa_x1^2*l1*cos(l1*(kappa_x1^2 + kappa_y1^2)^(1/2))*(kappa_x1^2 + kappa_y1^2)^(1/2) + kappa_y1^2*l1*cos(l1*(kappa_x1^2 + kappa_y1^2)^(1/2))*(kappa_x1^2 + kappa_y1^2)^(1/2)))/(l1*(kappa_x1^2 + kappa_y1^2)^(7/2)) - (2.0*dkappa_y1*kappa_y1*m*(3.0*kappa_x1^2*l1*(kappa_x1^2 + kappa_y1^2)^(1/2) - 3.0*kappa_x1^2*sin(l1*(kappa_x1^2 + kappa_y1^2)^(1/2)) - 3.0*kappa_y1^2*sin(l1*(kappa_x1^2 + kappa_y1^2)^(1/2)) - 1.0*l1*(kappa_x1^2 + kappa_y1^2)^(3/2) + 3.0*kappa_y1^2*l1*(kappa_x1^2 + kappa_y1^2)^(1/2) + kappa_x1^2*l1*cos(l1*(kappa_x1^2 + kappa_y1^2)^(1/2))*(kappa_x1^2 + kappa_y1^2)^(1/2) + kappa_y1^2*l1*cos(l1*(kappa_x1^2 + kappa_y1^2)^(1/2))*(kappa_x1^2 + kappa_y1^2)^(1/2)))/(l1*(kappa_x1^2 + kappa_y1^2)^(7/2));
V(1,2) = - (dkappa_y1*(4.0*kappa_x1*kappa_y1*m*sin(l1*(kappa_x1^2 + kappa_y1^2)^(1/2)) + 0.5*kappa_x1*kappa_y1*m*sin(2.0*l1*(kappa_x1^2 + kappa_y1^2)^(1/2)) - 2.0*kappa_x1*kappa_y1^3*m*r^2*sin(l1*(kappa_x1^2 + kappa_y1^2)^(1/2)) - 2.0*kappa_x1^3*kappa_y1*m*r^2*sin(l1*(kappa_x1^2 + kappa_y1^2)^(1/2)) + 60.0*kappa_x1*kappa_y1*l1*m*sin(l1*(kappa_x1^2 + kappa_y1^2)^(1/2)) + 0.125*kappa_x1*kappa_y1^3*m*r^2*sin(2.0*l1*(kappa_x1^2 + kappa_y1^2)^(1/2)) + 0.125*kappa_x1^3*kappa_y1*m*r^2*sin(2.0*l1*(kappa_x1^2 + kappa_y1^2)^(1/2)) - 32.0*kappa_x1*kappa_y1*l1^2*m*(kappa_x1^2 + kappa_y1^2)^(1/2) + 1.3333333333333333333333333333333*kappa_x1*kappa_y1*l1^3*m*(kappa_x1^2 + kappa_y1^2)^(3/2) - 1.0*kappa_x1*kappa_y1*l1*m*cos(2.0*l1*(kappa_x1^2 + kappa_y1^2)^(1/2))*(kappa_x1^2 + kappa_y1^2)^(1/2) - 28.0*kappa_x1*kappa_y1*l1^2*m*cos(l1*(kappa_x1^2 + kappa_y1^2)^(1/2))*(kappa_x1^2 + kappa_y1^2)^(1/2) - 4.0*kappa_x1*kappa_y1*l1*m*cos(l1*(kappa_x1^2 + kappa_y1^2)^(1/2))*(kappa_x1^2 + kappa_y1^2)^(1/2) + 0.33333333333333333333333333333333*kappa_x1*kappa_y1^3*l1^3*m*r^2*(kappa_x1^2 + kappa_y1^2)^(3/2) + 0.33333333333333333333333333333333*kappa_x1^3*kappa_y1*l1^3*m*r^2*(kappa_x1^2 + kappa_y1^2)^(3/2) - 4.0*kappa_x1*kappa_y1*l1^2*m*sin(l1*(kappa_x1^2 + kappa_y1^2)^(1/2))*(kappa_x1^2 + kappa_y1^2) - 4*kappa_x1*kappa_y1*l1^3*m*sin(l1*(kappa_x1^2 + kappa_y1^2)^(1/2))*(kappa_x1^2 + kappa_y1^2) + 2.0*kappa_x1*kappa_y1^3*l1*m*r^2*cos(l1*(kappa_x1^2 + kappa_y1^2)^(1/2))*(kappa_x1^2 + kappa_y1^2)^(1/2) + 2.0*kappa_x1^3*kappa_y1*l1*m*r^2*cos(l1*(kappa_x1^2 + kappa_y1^2)^(1/2))*(kappa_x1^2 + kappa_y1^2)^(1/2) - 0.25*kappa_x1*kappa_y1^3*l1*m*r^2*cos(2.0*l1*(kappa_x1^2 + kappa_y1^2)^(1/2))*(kappa_x1^2 + kappa_y1^2)^(1/2) - 0.25*kappa_x1^3*kappa_y1*l1*m*r^2*cos(2.0*l1*(kappa_x1^2 + kappa_y1^2)^(1/2))*(kappa_x1^2 + kappa_y1^2)^(1/2)))/(2*l1^2*(kappa_x1^2 + kappa_y1^2)^(7/2)) - (dkappa_x1*(8.0*kappa_x1^2*m*sin(l1*(kappa_x1^2 + kappa_y1^2)^(1/2)) + 4.0*kappa_y1^2*m*sin(l1*(kappa_x1^2 + kappa_y1^2)^(1/2)) - 0.5*kappa_y1^2*m*sin(2.0*l1*(kappa_x1^2 + kappa_y1^2)^(1/2)) + 8.0*l1^2*m*(kappa_x1^2 + kappa_y1^2)^(3/2) - 0.125*kappa_y1^4*m*r^2*sin(2.0*l1*(kappa_x1^2 + kappa_y1^2)^(1/2)) + 4*l1^2*m*cos(l1*(kappa_x1^2 + kappa_y1^2)^(1/2))*(kappa_x1^2 + kappa_y1^2)^(3/2) + 60.0*kappa_x1^2*l1*m*sin(l1*(kappa_x1^2 + kappa_y1^2)^(1/2)) - 32.0*kappa_x1^2*l1^2*m*(kappa_x1^2 + kappa_y1^2)^(1/2) + 1.3333333333333333333333333333333*kappa_x1^2*l1^3*m*(kappa_x1^2 + kappa_y1^2)^(3/2) - 12.0*l1*m*sin(l1*(kappa_x1^2 + kappa_y1^2)^(1/2))*(kappa_x1^2 + kappa_y1^2) + 2.0*kappa_y1^4*m*r^2*sin(l1*(kappa_x1^2 + kappa_y1^2)^(1/2)) - 0.125*kappa_x1^2*kappa_y1^2*m*r^2*sin(2.0*l1*(kappa_x1^2 + kappa_y1^2)^(1/2)) + kappa_y1^2*l1*m*cos(2.0*l1*(kappa_x1^2 + kappa_y1^2)^(1/2))*(kappa_x1^2 + kappa_y1^2)^(1/2) - 28.0*kappa_x1^2*l1^2*m*cos(l1*(kappa_x1^2 + kappa_y1^2)^(1/2))*(kappa_x1^2 + kappa_y1^2)^(1/2) + 0.33333333333333333333333333333333*kappa_x1^4*l1^3*m*r^2*(kappa_x1^2 + kappa_y1^2)^(3/2) + 2.0*kappa_x1^2*kappa_y1^2*m*r^2*sin(l1*(kappa_x1^2 + kappa_y1^2)^(1/2)) - 8.0*kappa_x1^2*l1*m*cos(l1*(kappa_x1^2 + kappa_y1^2)^(1/2))*(kappa_x1^2 + kappa_y1^2)^(1/2) - 4.0*kappa_y1^2*l1*m*cos(l1*(kappa_x1^2 + kappa_y1^2)^(1/2))*(kappa_x1^2 + kappa_y1^2)^(1/2) - 4.0*kappa_x1^2*l1^2*m*sin(l1*(kappa_x1^2 + kappa_y1^2)^(1/2))*(kappa_x1^2 + kappa_y1^2) - 4*kappa_x1^2*l1^3*m*sin(l1*(kappa_x1^2 + kappa_y1^2)^(1/2))*(kappa_x1^2 + kappa_y1^2) + 0.33333333333333333333333333333333*kappa_x1^2*kappa_y1^2*l1^3*m*r^2*(kappa_x1^2 + kappa_y1^2)^(3/2) - 2.0*kappa_y1^4*l1*m*r^2*cos(l1*(kappa_x1^2 + kappa_y1^2)^(1/2))*(kappa_x1^2 + kappa_y1^2)^(1/2) + 0.25*kappa_y1^4*l1*m*r^2*cos(2.0*l1*(kappa_x1^2 + kappa_y1^2)^(1/2))*(kappa_x1^2 + kappa_y1^2)^(1/2) - 2.0*kappa_x1^2*kappa_y1^2*l1*m*r^2*cos(l1*(kappa_x1^2 + kappa_y1^2)^(1/2))*(kappa_x1^2 + kappa_y1^2)^(1/2) + 0.25*kappa_x1^2*kappa_y1^2*l1*m*r^2*cos(2.0*l1*(kappa_x1^2 + kappa_y1^2)^(1/2))*(kappa_x1^2 + kappa_y1^2)^(1/2)))/(2*l1^2*(kappa_x1^2 + kappa_y1^2)^(7/2)) - (2.0*dl1*kappa_x1*m*(3.0*kappa_x1^2*l1*(kappa_x1^2 + kappa_y1^2)^(1/2) - 3.0*kappa_x1^2*sin(l1*(kappa_x1^2 + kappa_y1^2)^(1/2)) - 3.0*kappa_y1^2*sin(l1*(kappa_x1^2 + kappa_y1^2)^(1/2)) - 1.0*l1*(kappa_x1^2 + kappa_y1^2)^(3/2) + 3.0*kappa_y1^2*l1*(kappa_x1^2 + kappa_y1^2)^(1/2) + kappa_x1^2*l1*cos(l1*(kappa_x1^2 + kappa_y1^2)^(1/2))*(kappa_x1^2 + kappa_y1^2)^(1/2) + kappa_y1^2*l1*cos(l1*(kappa_x1^2 + kappa_y1^2)^(1/2))*(kappa_x1^2 + kappa_y1^2)^(1/2)))/(l1*(kappa_x1^2 + kappa_y1^2)^(7/2));
V(1,3) = - (dkappa_x1*(4.0*kappa_x1*kappa_y1*m*sin(l1*(kappa_x1^2 + kappa_y1^2)^(1/2)) + 0.5*kappa_x1*kappa_y1*m*sin(2.0*l1*(kappa_x1^2 + kappa_y1^2)^(1/2)) - 2.0*kappa_x1*kappa_y1^3*m*r^2*sin(l1*(kappa_x1^2 + kappa_y1^2)^(1/2)) - 2.0*kappa_x1^3*kappa_y1*m*r^2*sin(l1*(kappa_x1^2 + kappa_y1^2)^(1/2)) + 60.0*kappa_x1*kappa_y1*l1*m*sin(l1*(kappa_x1^2 + kappa_y1^2)^(1/2)) + 0.125*kappa_x1*kappa_y1^3*m*r^2*sin(2.0*l1*(kappa_x1^2 + kappa_y1^2)^(1/2)) + 0.125*kappa_x1^3*kappa_y1*m*r^2*sin(2.0*l1*(kappa_x1^2 + kappa_y1^2)^(1/2)) - 32.0*kappa_x1*kappa_y1*l1^2*m*(kappa_x1^2 + kappa_y1^2)^(1/2) + 1.3333333333333333333333333333333*kappa_x1*kappa_y1*l1^3*m*(kappa_x1^2 + kappa_y1^2)^(3/2) - 1.0*kappa_x1*kappa_y1*l1*m*cos(2.0*l1*(kappa_x1^2 + kappa_y1^2)^(1/2))*(kappa_x1^2 + kappa_y1^2)^(1/2) - 28.0*kappa_x1*kappa_y1*l1^2*m*cos(l1*(kappa_x1^2 + kappa_y1^2)^(1/2))*(kappa_x1^2 + kappa_y1^2)^(1/2) - 4.0*kappa_x1*kappa_y1*l1*m*cos(l1*(kappa_x1^2 + kappa_y1^2)^(1/2))*(kappa_x1^2 + kappa_y1^2)^(1/2) + 0.33333333333333333333333333333333*kappa_x1*kappa_y1^3*l1^3*m*r^2*(kappa_x1^2 + kappa_y1^2)^(3/2) + 0.33333333333333333333333333333333*kappa_x1^3*kappa_y1*l1^3*m*r^2*(kappa_x1^2 + kappa_y1^2)^(3/2) - 4.0*kappa_x1*kappa_y1*l1^2*m*sin(l1*(kappa_x1^2 + kappa_y1^2)^(1/2))*(kappa_x1^2 + kappa_y1^2) - 4*kappa_x1*kappa_y1*l1^3*m*sin(l1*(kappa_x1^2 + kappa_y1^2)^(1/2))*(kappa_x1^2 + kappa_y1^2) + 2.0*kappa_x1*kappa_y1^3*l1*m*r^2*cos(l1*(kappa_x1^2 + kappa_y1^2)^(1/2))*(kappa_x1^2 + kappa_y1^2)^(1/2) + 2.0*kappa_x1^3*kappa_y1*l1*m*r^2*cos(l1*(kappa_x1^2 + kappa_y1^2)^(1/2))*(kappa_x1^2 + kappa_y1^2)^(1/2) - 0.25*kappa_x1*kappa_y1^3*l1*m*r^2*cos(2.0*l1*(kappa_x1^2 + kappa_y1^2)^(1/2))*(kappa_x1^2 + kappa_y1^2)^(1/2) - 0.25*kappa_x1^3*kappa_y1*l1*m*r^2*cos(2.0*l1*(kappa_x1^2 + kappa_y1^2)^(1/2))*(kappa_x1^2 + kappa_y1^2)^(1/2)))/(2*l1^2*(kappa_x1^2 + kappa_y1^2)^(7/2)) - (dkappa_y1*(4.0*kappa_x1^2*m*sin(l1*(kappa_x1^2 + kappa_y1^2)^(1/2)) + 8.0*kappa_y1^2*m*sin(l1*(kappa_x1^2 + kappa_y1^2)^(1/2)) - 0.5*kappa_x1^2*m*sin(2.0*l1*(kappa_x1^2 + kappa_y1^2)^(1/2)) + 8.0*l1^2*m*(kappa_x1^2 + kappa_y1^2)^(3/2) - 0.125*kappa_x1^4*m*r^2*sin(2.0*l1*(kappa_x1^2 + kappa_y1^2)^(1/2)) + 4*l1^2*m*cos(l1*(kappa_x1^2 + kappa_y1^2)^(1/2))*(kappa_x1^2 + kappa_y1^2)^(3/2) + 60.0*kappa_y1^2*l1*m*sin(l1*(kappa_x1^2 + kappa_y1^2)^(1/2)) - 32.0*kappa_y1^2*l1^2*m*(kappa_x1^2 + kappa_y1^2)^(1/2) + 1.3333333333333333333333333333333*kappa_y1^2*l1^3*m*(kappa_x1^2 + kappa_y1^2)^(3/2) - 12.0*l1*m*sin(l1*(kappa_x1^2 + kappa_y1^2)^(1/2))*(kappa_x1^2 + kappa_y1^2) + 2.0*kappa_x1^4*m*r^2*sin(l1*(kappa_x1^2 + kappa_y1^2)^(1/2)) - 0.125*kappa_x1^2*kappa_y1^2*m*r^2*sin(2.0*l1*(kappa_x1^2 + kappa_y1^2)^(1/2)) + kappa_x1^2*l1*m*cos(2.0*l1*(kappa_x1^2 + kappa_y1^2)^(1/2))*(kappa_x1^2 + kappa_y1^2)^(1/2) - 28.0*kappa_y1^2*l1^2*m*cos(l1*(kappa_x1^2 + kappa_y1^2)^(1/2))*(kappa_x1^2 + kappa_y1^2)^(1/2) + 0.33333333333333333333333333333333*kappa_y1^4*l1^3*m*r^2*(kappa_x1^2 + kappa_y1^2)^(3/2) + 2.0*kappa_x1^2*kappa_y1^2*m*r^2*sin(l1*(kappa_x1^2 + kappa_y1^2)^(1/2)) - 4.0*kappa_x1^2*l1*m*cos(l1*(kappa_x1^2 + kappa_y1^2)^(1/2))*(kappa_x1^2 + kappa_y1^2)^(1/2) - 8.0*kappa_y1^2*l1*m*cos(l1*(kappa_x1^2 + kappa_y1^2)^(1/2))*(kappa_x1^2 + kappa_y1^2)^(1/2) - 4.0*kappa_y1^2*l1^2*m*sin(l1*(kappa_x1^2 + kappa_y1^2)^(1/2))*(kappa_x1^2 + kappa_y1^2) - 4*kappa_y1^2*l1^3*m*sin(l1*(kappa_x1^2 + kappa_y1^2)^(1/2))*(kappa_x1^2 + kappa_y1^2) + 0.33333333333333333333333333333333*kappa_x1^2*kappa_y1^2*l1^3*m*r^2*(kappa_x1^2 + kappa_y1^2)^(3/2) - 2.0*kappa_x1^4*l1*m*r^2*cos(l1*(kappa_x1^2 + kappa_y1^2)^(1/2))*(kappa_x1^2 + kappa_y1^2)^(1/2) + 0.25*kappa_x1^4*l1*m*r^2*cos(2.0*l1*(kappa_x1^2 + kappa_y1^2)^(1/2))*(kappa_x1^2 + kappa_y1^2)^(1/2) - 2.0*kappa_x1^2*kappa_y1^2*l1*m*r^2*cos(l1*(kappa_x1^2 + kappa_y1^2)^(1/2))*(kappa_x1^2 + kappa_y1^2)^(1/2) + 0.25*kappa_x1^2*kappa_y1^2*l1*m*r^2*cos(2.0*l1*(kappa_x1^2 + kappa_y1^2)^(1/2))*(kappa_x1^2 + kappa_y1^2)^(1/2)))/(2*l1^2*(kappa_x1^2 + kappa_y1^2)^(7/2)) - (2.0*dl1*kappa_y1*m*(3.0*kappa_x1^2*l1*(kappa_x1^2 + kappa_y1^2)^(1/2) - 3.0*kappa_x1^2*sin(l1*(kappa_x1^2 + kappa_y1^2)^(1/2)) - 3.0*kappa_y1^2*sin(l1*(kappa_x1^2 + kappa_y1^2)^(1/2)) - 1.0*l1*(kappa_x1^2 + kappa_y1^2)^(3/2) + 3.0*kappa_y1^2*l1*(kappa_x1^2 + kappa_y1^2)^(1/2) + kappa_x1^2*l1*cos(l1*(kappa_x1^2 + kappa_y1^2)^(1/2))*(kappa_x1^2 + kappa_y1^2)^(1/2) + kappa_y1^2*l1*cos(l1*(kappa_x1^2 + kappa_y1^2)^(1/2))*(kappa_x1^2 + kappa_y1^2)^(1/2)))/(l1*(kappa_x1^2 + kappa_y1^2)^(7/2));

V(2,1) = (dkappa_y1*(4.0*kappa_x1*kappa_y1*m*sin(l1*(kappa_x1^2 + kappa_y1^2)^(1/2)) + 0.5*kappa_x1*kappa_y1*m*sin(2.0*l1*(kappa_x1^2 + kappa_y1^2)^(1/2)) - 2.0*kappa_x1*kappa_y1^3*m*r^2*sin(l1*(kappa_x1^2 + kappa_y1^2)^(1/2)) - 2.0*kappa_x1^3*kappa_y1*m*r^2*sin(l1*(kappa_x1^2 + kappa_y1^2)^(1/2)) + 0.125*kappa_x1*kappa_y1^3*m*r^2*sin(2.0*l1*(kappa_x1^2 + kappa_y1^2)^(1/2)) + 0.125*kappa_x1^3*kappa_y1*m*r^2*sin(2.0*l1*(kappa_x1^2 + kappa_y1^2)^(1/2)) + 1.3333333333333333333333333333333*kappa_x1*kappa_y1*l1^3*m*(kappa_x1^2 + kappa_y1^2)^(3/2) - 1.0*kappa_x1*kappa_y1*l1*m*cos(2.0*l1*(kappa_x1^2 + kappa_y1^2)^(1/2))*(kappa_x1^2 + kappa_y1^2)^(1/2) - 4.0*kappa_x1*kappa_y1*l1*m*cos(l1*(kappa_x1^2 + kappa_y1^2)^(1/2))*(kappa_x1^2 + kappa_y1^2)^(1/2) + 0.33333333333333333333333333333333*kappa_x1*kappa_y1^3*l1^3*m*r^2*(kappa_x1^2 + kappa_y1^2)^(3/2) + 0.33333333333333333333333333333333*kappa_x1^3*kappa_y1*l1^3*m*r^2*(kappa_x1^2 + kappa_y1^2)^(3/2) - 4.0*kappa_x1*kappa_y1*l1^2*m*sin(l1*(kappa_x1^2 + kappa_y1^2)^(1/2))*(kappa_x1^2 + kappa_y1^2) + 2.0*kappa_x1*kappa_y1^3*l1*m*r^2*cos(l1*(kappa_x1^2 + kappa_y1^2)^(1/2))*(kappa_x1^2 + kappa_y1^2)^(1/2) + 2.0*kappa_x1^3*kappa_y1*l1*m*r^2*cos(l1*(kappa_x1^2 + kappa_y1^2)^(1/2))*(kappa_x1^2 + kappa_y1^2)^(1/2) - 0.25*kappa_x1*kappa_y1^3*l1*m*r^2*cos(2.0*l1*(kappa_x1^2 + kappa_y1^2)^(1/2))*(kappa_x1^2 + kappa_y1^2)^(1/2) - 0.25*kappa_x1^3*kappa_y1*l1*m*r^2*cos(2.0*l1*(kappa_x1^2 + kappa_y1^2)^(1/2))*(kappa_x1^2 + kappa_y1^2)^(1/2)))/(2*l1^2*(kappa_x1^2 + kappa_y1^2)^(7/2)) + (dkappa_x1*(8.0*kappa_x1^2*m*sin(l1*(kappa_x1^2 + kappa_y1^2)^(1/2)) + 4.0*kappa_y1^2*m*sin(l1*(kappa_x1^2 + kappa_y1^2)^(1/2)) - 0.5*kappa_y1^2*m*sin(2.0*l1*(kappa_x1^2 + kappa_y1^2)^(1/2)) - 0.125*kappa_y1^4*m*r^2*sin(2.0*l1*(kappa_x1^2 + kappa_y1^2)^(1/2)) + 1.3333333333333333333333333333333*kappa_x1^2*l1^3*m*(kappa_x1^2 + kappa_y1^2)^(3/2) + 2.0*kappa_y1^4*m*r^2*sin(l1*(kappa_x1^2 + kappa_y1^2)^(1/2)) - 0.125*kappa_x1^2*kappa_y1^2*m*r^2*sin(2.0*l1*(kappa_x1^2 + kappa_y1^2)^(1/2)) + kappa_y1^2*l1*m*cos(2.0*l1*(kappa_x1^2 + kappa_y1^2)^(1/2))*(kappa_x1^2 + kappa_y1^2)^(1/2) + 0.33333333333333333333333333333333*kappa_x1^4*l1^3*m*r^2*(kappa_x1^2 + kappa_y1^2)^(3/2) + 2.0*kappa_x1^2*kappa_y1^2*m*r^2*sin(l1*(kappa_x1^2 + kappa_y1^2)^(1/2)) - 8.0*kappa_x1^2*l1*m*cos(l1*(kappa_x1^2 + kappa_y1^2)^(1/2))*(kappa_x1^2 + kappa_y1^2)^(1/2) - 4.0*kappa_y1^2*l1*m*cos(l1*(kappa_x1^2 + kappa_y1^2)^(1/2))*(kappa_x1^2 + kappa_y1^2)^(1/2) - 4.0*kappa_x1^2*l1^2*m*sin(l1*(kappa_x1^2 + kappa_y1^2)^(1/2))*(kappa_x1^2 + kappa_y1^2) + 0.33333333333333333333333333333333*kappa_x1^2*kappa_y1^2*l1^3*m*r^2*(kappa_x1^2 + kappa_y1^2)^(3/2) - 2.0*kappa_y1^4*l1*m*r^2*cos(l1*(kappa_x1^2 + kappa_y1^2)^(1/2))*(kappa_x1^2 + kappa_y1^2)^(1/2) + 0.25*kappa_y1^4*l1*m*r^2*cos(2.0*l1*(kappa_x1^2 + kappa_y1^2)^(1/2))*(kappa_x1^2 + kappa_y1^2)^(1/2) - 2.0*kappa_x1^2*kappa_y1^2*l1*m*r^2*cos(l1*(kappa_x1^2 + kappa_y1^2)^(1/2))*(kappa_x1^2 + kappa_y1^2)^(1/2) + 0.25*kappa_x1^2*kappa_y1^2*l1*m*r^2*cos(2.0*l1*(kappa_x1^2 + kappa_y1^2)^(1/2))*(kappa_x1^2 + kappa_y1^2)^(1/2)))/(2*l1^2*(kappa_x1^2 + kappa_y1^2)^(7/2)) + (dl1*(12.0*kappa_x1^3*l1^2*m*(kappa_x1^2 + kappa_y1^2)^(1/2) - 20.0*kappa_x1^3*l1*m*sin(l1*(kappa_x1^2 + kappa_y1^2)^(1/2)) - 4.0*kappa_x1*l1^2*m*(kappa_x1^2 + kappa_y1^2)^(3/2) - 12.0*kappa_x1*m*sin(l1*(kappa_x1^2 + kappa_y1^2)^(1/2))*(kappa_x1^2 + kappa_y1^2) - 20.0*kappa_x1*kappa_y1^2*l1*m*sin(l1*(kappa_x1^2 + kappa_y1^2)^(1/2)) + 12.0*kappa_x1*kappa_y1^2*l1^2*m*(kappa_x1^2 + kappa_y1^2)^(1/2) + 8.0*kappa_x1*l1*m*sin(l1*(kappa_x1^2 + kappa_y1^2)^(1/2))*(kappa_x1^2 + kappa_y1^2) + 4.0*kappa_x1^3*l1^2*m*cos(l1*(kappa_x1^2 + kappa_y1^2)^(1/2))*(kappa_x1^2 + kappa_y1^2)^(1/2) + 12.0*kappa_x1*l1*m*cos(l1*(kappa_x1^2 + kappa_y1^2)^(1/2))*(kappa_x1^2 + kappa_y1^2)^(3/2) + 4*kappa_x1*l1^2*m*sin(l1*(kappa_x1^2 + kappa_y1^2)^(1/2))*(kappa_x1^2 + kappa_y1^2)^2 + 4.0*kappa_x1*kappa_y1^2*l1^2*m*cos(l1*(kappa_x1^2 + kappa_y1^2)^(1/2))*(kappa_x1^2 + kappa_y1^2)^(1/2)))/(2*l1^2*(kappa_x1^2 + kappa_y1^2)^(7/2));
V(2,2) = (dl1*(8.0*kappa_x1^2*m*sin(l1*(kappa_x1^2 + kappa_y1^2)^(1/2)) + 4.0*kappa_y1^2*m*sin(l1*(kappa_x1^2 + kappa_y1^2)^(1/2)) - 0.5*kappa_y1^2*m*sin(2.0*l1*(kappa_x1^2 + kappa_y1^2)^(1/2)) - 0.125*kappa_y1^4*m*r^2*sin(2.0*l1*(kappa_x1^2 + kappa_y1^2)^(1/2)) + 1.3333333333333333333333333333333*kappa_x1^2*l1^3*m*(kappa_x1^2 + kappa_y1^2)^(3/2) + 2.0*kappa_y1^4*m*r^2*sin(l1*(kappa_x1^2 + kappa_y1^2)^(1/2)) - 0.125*kappa_x1^2*kappa_y1^2*m*r^2*sin(2.0*l1*(kappa_x1^2 + kappa_y1^2)^(1/2)) + kappa_y1^2*l1*m*cos(2.0*l1*(kappa_x1^2 + kappa_y1^2)^(1/2))*(kappa_x1^2 + kappa_y1^2)^(1/2) + 0.33333333333333333333333333333333*kappa_x1^4*l1^3*m*r^2*(kappa_x1^2 + kappa_y1^2)^(3/2) + 2.0*kappa_x1^2*kappa_y1^2*m*r^2*sin(l1*(kappa_x1^2 + kappa_y1^2)^(1/2)) - 8.0*kappa_x1^2*l1*m*cos(l1*(kappa_x1^2 + kappa_y1^2)^(1/2))*(kappa_x1^2 + kappa_y1^2)^(1/2) - 4.0*kappa_y1^2*l1*m*cos(l1*(kappa_x1^2 + kappa_y1^2)^(1/2))*(kappa_x1^2 + kappa_y1^2)^(1/2) - 4.0*kappa_x1^2*l1^2*m*sin(l1*(kappa_x1^2 + kappa_y1^2)^(1/2))*(kappa_x1^2 + kappa_y1^2) + 0.33333333333333333333333333333333*kappa_x1^2*kappa_y1^2*l1^3*m*r^2*(kappa_x1^2 + kappa_y1^2)^(3/2) - 2.0*kappa_y1^4*l1*m*r^2*cos(l1*(kappa_x1^2 + kappa_y1^2)^(1/2))*(kappa_x1^2 + kappa_y1^2)^(1/2) + 0.25*kappa_y1^4*l1*m*r^2*cos(2.0*l1*(kappa_x1^2 + kappa_y1^2)^(1/2))*(kappa_x1^2 + kappa_y1^2)^(1/2) - 2.0*kappa_x1^2*kappa_y1^2*l1*m*r^2*cos(l1*(kappa_x1^2 + kappa_y1^2)^(1/2))*(kappa_x1^2 + kappa_y1^2)^(1/2) + 0.25*kappa_x1^2*kappa_y1^2*l1*m*r^2*cos(2.0*l1*(kappa_x1^2 + kappa_y1^2)^(1/2))*(kappa_x1^2 + kappa_y1^2)^(1/2)))/(2*l1^2*(kappa_x1^2 + kappa_y1^2)^(7/2)) - (5.0e-34*dkappa_y1*(2.5e33*kappa_y1^3*m*sin(2.0*l1*(kappa_x1^2 + kappa_y1^2)^(1/2)) - 2.0e34*kappa_y1^3*m*sin(l1*(kappa_x1^2 + kappa_y1^2)^(1/2)) + 375000000000000000000000000000000.0*kappa_y1^5*m*r^2*sin(2.0*l1*(kappa_x1^2 + kappa_y1^2)^(1/2)) - 4.8e34*kappa_x1^2*kappa_y1*m*sin(l1*(kappa_x1^2 + kappa_y1^2)^(1/2)) - 1.0e33*kappa_x1^2*kappa_y1*m*sin(2.0*l1*(kappa_x1^2 + kappa_y1^2)^(1/2)) + 1.2e34*kappa_y1*l1*m*(kappa_x1^2 + kappa_y1^2)^(3/2) - 6.0e33*kappa_y1^5*m*r^2*sin(l1*(kappa_x1^2 + kappa_y1^2)^(1/2)) + 125000000000000000000000000000000.0*kappa_x1^2*kappa_y1^3*m*r^2*sin(2.0*l1*(kappa_x1^2 + kappa_y1^2)^(1/2)) - 1.0e33*kappa_y1^3*l1*m*cos(2.0*l1*(kappa_x1^2 + kappa_y1^2)^(1/2))*(kappa_x1^2 + kappa_y1^2)^(1/2) + 2.6666666666666666666666666666667e33*kappa_x1^2*kappa_y1*l1^3*m*(kappa_x1^2 + kappa_y1^2)^(3/2) + 5.0e33*kappa_y1^3*l1*m*r^2*(kappa_x1^2 + kappa_y1^2)^(3/2) + 1.5e33*kappa_y1^5*l1*m*r^2*(kappa_x1^2 + kappa_y1^2)^(1/2) + 4.0e33*kappa_x1^4*kappa_y1*l1^2*m*sin(l1*(kappa_x1^2 + kappa_y1^2)^(1/2)) + 4.0e33*kappa_x1^4*kappa_y1*m*r^2*sin(l1*(kappa_x1^2 + kappa_y1^2)^(1/2)) - 250000000000000000000000000000000.0*kappa_x1^4*kappa_y1*m*r^2*sin(2.0*l1*(kappa_x1^2 + kappa_y1^2)^(1/2)) + 4.0e33*kappa_x1^2*kappa_y1^3*l1^2*m*sin(l1*(kappa_x1^2 + kappa_y1^2)^(1/2)) + 6.0e33*kappa_x1^2*kappa_y1*l1*m*(kappa_x1^2 + kappa_y1^2)^(1/2) - 2.0e33*kappa_x1^2*kappa_y1^3*m*r^2*sin(l1*(kappa_x1^2 + kappa_y1^2)^(1/2)) - 3.0e33*kappa_y1*l1*m*r^2*(kappa_x1^2 + kappa_y1^2)^(5/2) + 4.0e33*kappa_y1^3*l1*m*cos(l1*(kappa_x1^2 + kappa_y1^2)^(1/2))*(kappa_x1^2 + kappa_y1^2)^(1/2) + 3.2e34*kappa_x1^2*kappa_y1*l1*m*cos(l1*(kappa_x1^2 + kappa_y1^2)^(1/2))*(kappa_x1^2 + kappa_y1^2)^(1/2) + 666666666666666666666666666666677.0*kappa_x1^2*kappa_y1^3*l1^3*m*r^2*(kappa_x1^2 + kappa_y1^2)^(3/2) - 500000000000000000000000000000000.0*kappa_x1^2*kappa_y1*l1*m*r^2*(kappa_x1^2 + kappa_y1^2)^(3/2) + 2.0e33*kappa_y1^5*l1*m*r^2*cos(l1*(kappa_x1^2 + kappa_y1^2)^(1/2))*(kappa_x1^2 + kappa_y1^2)^(1/2) - 250000000000000000000000000000000.0*kappa_y1^5*l1*m*r^2*cos(2.0*l1*(kappa_x1^2 + kappa_y1^2)^(1/2))*(kappa_x1^2 + kappa_y1^2)^(1/2) + 1.5e33*kappa_x1^2*kappa_y1^3*l1*m*r^2*(kappa_x1^2 + kappa_y1^2)^(1/2) - 333333333333333333333333333333333.0*kappa_x1^2*kappa_y1*l1^3*m*r^2*(kappa_x1^2 + kappa_y1^2)^(5/2) + 666666666666666666666666666666677.0*kappa_x1^4*kappa_y1*l1^3*m*r^2*(kappa_x1^2 + kappa_y1^2)^(3/2) + 2.0e33*kappa_x1^2*kappa_y1^3*l1*m*r^2*cos(l1*(kappa_x1^2 + kappa_y1^2)^(1/2))*(kappa_x1^2 + kappa_y1^2)^(1/2) - 250000000000000000000000000000000.0*kappa_x1^2*kappa_y1^3*l1*m*r^2*cos(2.0*l1*(kappa_x1^2 + kappa_y1^2)^(1/2))*(kappa_x1^2 + kappa_y1^2)^(1/2)))/(l1*(kappa_x1^2 + kappa_y1^2)^(9/2)) - (5.0e-34*dkappa_x1*(6.0e33*kappa_x1^3*l1*m*(kappa_x1^2 + kappa_y1^2)^(1/2) - 4.0e34*kappa_x1^3*m*sin(l1*(kappa_x1^2 + kappa_y1^2)^(1/2)) - 1.3333333333333333333333333333333e33*kappa_x1*l1^3*m*(kappa_x1^2 + kappa_y1^2)^(5/2) - 1.2e34*kappa_x1*kappa_y1^2*m*sin(l1*(kappa_x1^2 + kappa_y1^2)^(1/2)) + 2.6666666666666666666666666666667e33*kappa_x1^3*l1^3*m*(kappa_x1^2 + kappa_y1^2)^(3/2) + 3.5e33*kappa_x1*kappa_y1^2*m*sin(2.0*l1*(kappa_x1^2 + kappa_y1^2)^(1/2)) + 4.0e33*kappa_x1^5*l1^2*m*sin(l1*(kappa_x1^2 + kappa_y1^2)^(1/2)) + 1.0e34*kappa_x1*l1*m*(kappa_x1^2 + kappa_y1^2)^(3/2) + 625000000000000000000000000000000.0*kappa_x1^3*kappa_y1^2*m*r^2*sin(2.0*l1*(kappa_x1^2 + kappa_y1^2)^(1/2)) - 1.0e34*kappa_x1*kappa_y1^4*m*r^2*sin(l1*(kappa_x1^2 + kappa_y1^2)^(1/2)) - 8.0e33*kappa_x1*l1*m*cos(l1*(kappa_x1^2 + kappa_y1^2)^(1/2))*(kappa_x1^2 + kappa_y1^2)^(3/2) - 666666666666666666666666666666677.0*kappa_x1^3*l1^3*m*r^2*(kappa_x1^2 + kappa_y1^2)^(5/2) + 666666666666666666666666666666677.0*kappa_x1^5*l1^3*m*r^2*(kappa_x1^2 + kappa_y1^2)^(3/2) + 625000000000000000000000000000000.0*kappa_x1*kappa_y1^4*m*r^2*sin(2.0*l1*(kappa_x1^2 + kappa_y1^2)^(1/2)) + 4.0e33*kappa_x1^3*kappa_y1^2*l1^2*m*sin(l1*(kappa_x1^2 + kappa_y1^2)^(1/2)) - 1.0e34*kappa_x1^3*kappa_y1^2*m*r^2*sin(l1*(kappa_x1^2 + kappa_y1^2)^(1/2)) + 3.2e34*kappa_x1^3*l1*m*cos(l1*(kappa_x1^2 + kappa_y1^2)^(1/2))*(kappa_x1^2 + kappa_y1^2)^(1/2) + 4.0e33*kappa_x1*kappa_y1^2*l1*m*cos(l1*(kappa_x1^2 + kappa_y1^2)^(1/2))*(kappa_x1^2 + kappa_y1^2)^(1/2) + 666666666666666666666666666666677.0*kappa_x1^3*kappa_y1^2*l1^3*m*r^2*(kappa_x1^2 + kappa_y1^2)^(3/2) - 1.0e33*kappa_x1*kappa_y1^2*l1*m*cos(2.0*l1*(kappa_x1^2 + kappa_y1^2)^(1/2))*(kappa_x1^2 + kappa_y1^2)^(1/2) + 5.5e33*kappa_x1*kappa_y1^2*l1*m*r^2*(kappa_x1^2 + kappa_y1^2)^(3/2) + 1.5e33*kappa_x1*kappa_y1^4*l1*m*r^2*(kappa_x1^2 + kappa_y1^2)^(1/2) + 1.5e33*kappa_x1^3*kappa_y1^2*l1*m*r^2*(kappa_x1^2 + kappa_y1^2)^(1/2) - 333333333333333333333333333333333.0*kappa_x1*kappa_y1^2*l1^3*m*r^2*(kappa_x1^2 + kappa_y1^2)^(5/2) + 2.0e33*kappa_x1*kappa_y1^4*l1*m*r^2*cos(l1*(kappa_x1^2 + kappa_y1^2)^(1/2))*(kappa_x1^2 + kappa_y1^2)^(1/2) - 250000000000000000000000000000000.0*kappa_x1*kappa_y1^4*l1*m*r^2*cos(2.0*l1*(kappa_x1^2 + kappa_y1^2)^(1/2))*(kappa_x1^2 + kappa_y1^2)^(1/2) + 2.0e33*kappa_x1^3*kappa_y1^2*l1*m*r^2*cos(l1*(kappa_x1^2 + kappa_y1^2)^(1/2))*(kappa_x1^2 + kappa_y1^2)^(1/2) - 250000000000000000000000000000000.0*kappa_x1^3*kappa_y1^2*l1*m*r^2*cos(2.0*l1*(kappa_x1^2 + kappa_y1^2)^(1/2))*(kappa_x1^2 + kappa_y1^2)^(1/2)))/(l1*(kappa_x1^2 + kappa_y1^2)^(9/2));
V(2,3) = (dkappa_y1*(1.5*kappa_x1^3*m*sin(2.0*l1*(kappa_x1^2 + kappa_y1^2)^(1/2)) - 28.0*kappa_x1^3*m*sin(l1*(kappa_x1^2 + kappa_y1^2)^(1/2)) + 0.125*kappa_x1^5*m*r^2*sin(2.0*l1*(kappa_x1^2 + kappa_y1^2)^(1/2)) + 1.3333333333333333333333333333333*kappa_x1*l1^3*m*(kappa_x1^2 + kappa_y1^2)^(5/2) + 5.0*kappa_x1*kappa_y1^2*m*sin(2.0*l1*(kappa_x1^2 + kappa_y1^2)^(1/2)) + 14.0*kappa_x1*l1*m*(kappa_x1^2 + kappa_y1^2)^(3/2) - 2.0*kappa_x1^5*m*r^2*sin(l1*(kappa_x1^2 + kappa_y1^2)^(1/2)) + 0.875*kappa_x1^3*kappa_y1^2*m*r^2*sin(2.0*l1*(kappa_x1^2 + kappa_y1^2)^(1/2)) - 1.0*kappa_x1^3*l1*m*cos(2.0*l1*(kappa_x1^2 + kappa_y1^2)^(1/2))*(kappa_x1^2 + kappa_y1^2)^(1/2) - 2.6666666666666666666666666666667*kappa_x1*kappa_y1^2*l1^3*m*(kappa_x1^2 + kappa_y1^2)^(3/2) + 4.5*kappa_x1^3*l1*m*r^2*(kappa_x1^2 + kappa_y1^2)^(3/2) + 1.5*kappa_x1^5*l1*m*r^2*(kappa_x1^2 + kappa_y1^2)^(1/2) - 4.0*kappa_x1*kappa_y1^4*l1^2*m*sin(l1*(kappa_x1^2 + kappa_y1^2)^(1/2)) - 12.0*kappa_x1*kappa_y1^4*m*r^2*sin(l1*(kappa_x1^2 + kappa_y1^2)^(1/2)) + 8.0*kappa_x1*l1*m*cos(l1*(kappa_x1^2 + kappa_y1^2)^(1/2))*(kappa_x1^2 + kappa_y1^2)^(3/2) + 0.33333333333333333333333333333333*kappa_x1^3*l1^3*m*r^2*(kappa_x1^2 + kappa_y1^2)^(5/2) + 0.75*kappa_x1*kappa_y1^4*m*r^2*sin(2.0*l1*(kappa_x1^2 + kappa_y1^2)^(1/2)) - 4.0*kappa_x1^3*kappa_y1^2*l1^2*m*sin(l1*(kappa_x1^2 + kappa_y1^2)^(1/2)) - 6.0*kappa_x1*kappa_y1^2*l1*m*(kappa_x1^2 + kappa_y1^2)^(1/2) - 14.0*kappa_x1^3*kappa_y1^2*m*r^2*sin(l1*(kappa_x1^2 + kappa_y1^2)^(1/2)) - 6.0*kappa_x1*l1*m*r^2*(kappa_x1^2 + kappa_y1^2)^(5/2) + 4.0*kappa_x1^3*l1*m*cos(l1*(kappa_x1^2 + kappa_y1^2)^(1/2))*(kappa_x1^2 + kappa_y1^2)^(1/2) - 24.0*kappa_x1*kappa_y1^2*l1*m*cos(l1*(kappa_x1^2 + kappa_y1^2)^(1/2))*(kappa_x1^2 + kappa_y1^2)^(1/2) - 0.66666666666666666666666666666667*kappa_x1^3*kappa_y1^2*l1^3*m*r^2*(kappa_x1^2 + kappa_y1^2)^(3/2) - 2.0*kappa_x1*kappa_y1^2*l1*m*cos(2.0*l1*(kappa_x1^2 + kappa_y1^2)^(1/2))*(kappa_x1^2 + kappa_y1^2)^(1/2) + 10.0*kappa_x1*kappa_y1^2*l1*m*r^2*(kappa_x1^2 + kappa_y1^2)^(3/2) + 3.0*kappa_x1*kappa_y1^4*l1*m*r^2*(kappa_x1^2 + kappa_y1^2)^(1/2) + 2.0*kappa_x1^5*l1*m*r^2*cos(l1*(kappa_x1^2 + kappa_y1^2)^(1/2))*(kappa_x1^2 + kappa_y1^2)^(1/2) - 0.25*kappa_x1^5*l1*m*r^2*cos(2.0*l1*(kappa_x1^2 + kappa_y1^2)^(1/2))*(kappa_x1^2 + kappa_y1^2)^(1/2) + 4.5*kappa_x1^3*kappa_y1^2*l1*m*r^2*(kappa_x1^2 + kappa_y1^2)^(1/2) + 0.66666666666666666666666666666667*kappa_x1*kappa_y1^2*l1^3*m*r^2*(kappa_x1^2 + kappa_y1^2)^(5/2) - 0.66666666666666666666666666666667*kappa_x1*kappa_y1^4*l1^3*m*r^2*(kappa_x1^2 + kappa_y1^2)^(3/2) + 4.0*kappa_x1*kappa_y1^4*l1*m*r^2*cos(l1*(kappa_x1^2 + kappa_y1^2)^(1/2))*(kappa_x1^2 + kappa_y1^2)^(1/2) - 0.5*kappa_x1*kappa_y1^4*l1*m*r^2*cos(2.0*l1*(kappa_x1^2 + kappa_y1^2)^(1/2))*(kappa_x1^2 + kappa_y1^2)^(1/2) + 6.0*kappa_x1^3*kappa_y1^2*l1*m*r^2*cos(l1*(kappa_x1^2 + kappa_y1^2)^(1/2))*(kappa_x1^2 + kappa_y1^2)^(1/2) - 0.75*kappa_x1^3*kappa_y1^2*l1*m*r^2*cos(2.0*l1*(kappa_x1^2 + kappa_y1^2)^(1/2))*(kappa_x1^2 + kappa_y1^2)^(1/2)))/(2*l1*(kappa_x1^2 + kappa_y1^2)^(9/2)) - (5.0e-34*dkappa_x1*(2.5e33*kappa_y1^3*m*sin(2.0*l1*(kappa_x1^2 + kappa_y1^2)^(1/2)) - 2.0e34*kappa_y1^3*m*sin(l1*(kappa_x1^2 + kappa_y1^2)^(1/2)) + 375000000000000000000000000000000.0*kappa_y1^5*m*r^2*sin(2.0*l1*(kappa_x1^2 + kappa_y1^2)^(1/2)) - 4.8e34*kappa_x1^2*kappa_y1*m*sin(l1*(kappa_x1^2 + kappa_y1^2)^(1/2)) - 1.0e33*kappa_x1^2*kappa_y1*m*sin(2.0*l1*(kappa_x1^2 + kappa_y1^2)^(1/2)) + 1.2e34*kappa_y1*l1*m*(kappa_x1^2 + kappa_y1^2)^(3/2) - 6.0e33*kappa_y1^5*m*r^2*sin(l1*(kappa_x1^2 + kappa_y1^2)^(1/2)) + 125000000000000000000000000000000.0*kappa_x1^2*kappa_y1^3*m*r^2*sin(2.0*l1*(kappa_x1^2 + kappa_y1^2)^(1/2)) - 1.0e33*kappa_y1^3*l1*m*cos(2.0*l1*(kappa_x1^2 + kappa_y1^2)^(1/2))*(kappa_x1^2 + kappa_y1^2)^(1/2) + 2.6666666666666666666666666666667e33*kappa_x1^2*kappa_y1*l1^3*m*(kappa_x1^2 + kappa_y1^2)^(3/2) + 5.0e33*kappa_y1^3*l1*m*r^2*(kappa_x1^2 + kappa_y1^2)^(3/2) + 1.5e33*kappa_y1^5*l1*m*r^2*(kappa_x1^2 + kappa_y1^2)^(1/2) + 4.0e33*kappa_x1^4*kappa_y1*l1^2*m*sin(l1*(kappa_x1^2 + kappa_y1^2)^(1/2)) + 4.0e33*kappa_x1^4*kappa_y1*m*r^2*sin(l1*(kappa_x1^2 + kappa_y1^2)^(1/2)) - 250000000000000000000000000000000.0*kappa_x1^4*kappa_y1*m*r^2*sin(2.0*l1*(kappa_x1^2 + kappa_y1^2)^(1/2)) + 4.0e33*kappa_x1^2*kappa_y1^3*l1^2*m*sin(l1*(kappa_x1^2 + kappa_y1^2)^(1/2)) + 6.0e33*kappa_x1^2*kappa_y1*l1*m*(kappa_x1^2 + kappa_y1^2)^(1/2) - 2.0e33*kappa_x1^2*kappa_y1^3*m*r^2*sin(l1*(kappa_x1^2 + kappa_y1^2)^(1/2)) - 3.0e33*kappa_y1*l1*m*r^2*(kappa_x1^2 + kappa_y1^2)^(5/2) + 4.0e33*kappa_y1^3*l1*m*cos(l1*(kappa_x1^2 + kappa_y1^2)^(1/2))*(kappa_x1^2 + kappa_y1^2)^(1/2) + 3.2e34*kappa_x1^2*kappa_y1*l1*m*cos(l1*(kappa_x1^2 + kappa_y1^2)^(1/2))*(kappa_x1^2 + kappa_y1^2)^(1/2) + 666666666666666666666666666666677.0*kappa_x1^2*kappa_y1^3*l1^3*m*r^2*(kappa_x1^2 + kappa_y1^2)^(3/2) - 500000000000000000000000000000000.0*kappa_x1^2*kappa_y1*l1*m*r^2*(kappa_x1^2 + kappa_y1^2)^(3/2) + 2.0e33*kappa_y1^5*l1*m*r^2*cos(l1*(kappa_x1^2 + kappa_y1^2)^(1/2))*(kappa_x1^2 + kappa_y1^2)^(1/2) - 250000000000000000000000000000000.0*kappa_y1^5*l1*m*r^2*cos(2.0*l1*(kappa_x1^2 + kappa_y1^2)^(1/2))*(kappa_x1^2 + kappa_y1^2)^(1/2) + 1.5e33*kappa_x1^2*kappa_y1^3*l1*m*r^2*(kappa_x1^2 + kappa_y1^2)^(1/2) - 333333333333333333333333333333333.0*kappa_x1^2*kappa_y1*l1^3*m*r^2*(kappa_x1^2 + kappa_y1^2)^(5/2) + 666666666666666666666666666666677.0*kappa_x1^4*kappa_y1*l1^3*m*r^2*(kappa_x1^2 + kappa_y1^2)^(3/2) + 2.0e33*kappa_x1^2*kappa_y1^3*l1*m*r^2*cos(l1*(kappa_x1^2 + kappa_y1^2)^(1/2))*(kappa_x1^2 + kappa_y1^2)^(1/2) - 250000000000000000000000000000000.0*kappa_x1^2*kappa_y1^3*l1*m*r^2*cos(2.0*l1*(kappa_x1^2 + kappa_y1^2)^(1/2))*(kappa_x1^2 + kappa_y1^2)^(1/2)))/(l1*(kappa_x1^2 + kappa_y1^2)^(9/2)) + (dl1*(4.0*kappa_x1*kappa_y1*m*sin(l1*(kappa_x1^2 + kappa_y1^2)^(1/2)) + 0.5*kappa_x1*kappa_y1*m*sin(2.0*l1*(kappa_x1^2 + kappa_y1^2)^(1/2)) - 2.0*kappa_x1*kappa_y1^3*m*r^2*sin(l1*(kappa_x1^2 + kappa_y1^2)^(1/2)) - 2.0*kappa_x1^3*kappa_y1*m*r^2*sin(l1*(kappa_x1^2 + kappa_y1^2)^(1/2)) + 0.125*kappa_x1*kappa_y1^3*m*r^2*sin(2.0*l1*(kappa_x1^2 + kappa_y1^2)^(1/2)) + 0.125*kappa_x1^3*kappa_y1*m*r^2*sin(2.0*l1*(kappa_x1^2 + kappa_y1^2)^(1/2)) + 1.3333333333333333333333333333333*kappa_x1*kappa_y1*l1^3*m*(kappa_x1^2 + kappa_y1^2)^(3/2) - 1.0*kappa_x1*kappa_y1*l1*m*cos(2.0*l1*(kappa_x1^2 + kappa_y1^2)^(1/2))*(kappa_x1^2 + kappa_y1^2)^(1/2) - 4.0*kappa_x1*kappa_y1*l1*m*cos(l1*(kappa_x1^2 + kappa_y1^2)^(1/2))*(kappa_x1^2 + kappa_y1^2)^(1/2) + 0.33333333333333333333333333333333*kappa_x1*kappa_y1^3*l1^3*m*r^2*(kappa_x1^2 + kappa_y1^2)^(3/2) + 0.33333333333333333333333333333333*kappa_x1^3*kappa_y1*l1^3*m*r^2*(kappa_x1^2 + kappa_y1^2)^(3/2) - 4.0*kappa_x1*kappa_y1*l1^2*m*sin(l1*(kappa_x1^2 + kappa_y1^2)^(1/2))*(kappa_x1^2 + kappa_y1^2) + 2.0*kappa_x1*kappa_y1^3*l1*m*r^2*cos(l1*(kappa_x1^2 + kappa_y1^2)^(1/2))*(kappa_x1^2 + kappa_y1^2)^(1/2) + 2.0*kappa_x1^3*kappa_y1*l1*m*r^2*cos(l1*(kappa_x1^2 + kappa_y1^2)^(1/2))*(kappa_x1^2 + kappa_y1^2)^(1/2) - 0.25*kappa_x1*kappa_y1^3*l1*m*r^2*cos(2.0*l1*(kappa_x1^2 + kappa_y1^2)^(1/2))*(kappa_x1^2 + kappa_y1^2)^(1/2) - 0.25*kappa_x1^3*kappa_y1*l1*m*r^2*cos(2.0*l1*(kappa_x1^2 + kappa_y1^2)^(1/2))*(kappa_x1^2 + kappa_y1^2)^(1/2)))/(2*l1^2*(kappa_x1^2 + kappa_y1^2)^(7/2));
 
V(3,1) = (dkappa_x1*(4.0*kappa_x1*kappa_y1*m*sin(l1*(kappa_x1^2 + kappa_y1^2)^(1/2)) + 0.5*kappa_x1*kappa_y1*m*sin(2.0*l1*(kappa_x1^2 + kappa_y1^2)^(1/2)) - 2.0*kappa_x1*kappa_y1^3*m*r^2*sin(l1*(kappa_x1^2 + kappa_y1^2)^(1/2)) - 2.0*kappa_x1^3*kappa_y1*m*r^2*sin(l1*(kappa_x1^2 + kappa_y1^2)^(1/2)) + 0.125*kappa_x1*kappa_y1^3*m*r^2*sin(2.0*l1*(kappa_x1^2 + kappa_y1^2)^(1/2)) + 0.125*kappa_x1^3*kappa_y1*m*r^2*sin(2.0*l1*(kappa_x1^2 + kappa_y1^2)^(1/2)) + 1.3333333333333333333333333333333*kappa_x1*kappa_y1*l1^3*m*(kappa_x1^2 + kappa_y1^2)^(3/2) - 1.0*kappa_x1*kappa_y1*l1*m*cos(2.0*l1*(kappa_x1^2 + kappa_y1^2)^(1/2))*(kappa_x1^2 + kappa_y1^2)^(1/2) - 4.0*kappa_x1*kappa_y1*l1*m*cos(l1*(kappa_x1^2 + kappa_y1^2)^(1/2))*(kappa_x1^2 + kappa_y1^2)^(1/2) + 0.33333333333333333333333333333333*kappa_x1*kappa_y1^3*l1^3*m*r^2*(kappa_x1^2 + kappa_y1^2)^(3/2) + 0.33333333333333333333333333333333*kappa_x1^3*kappa_y1*l1^3*m*r^2*(kappa_x1^2 + kappa_y1^2)^(3/2) - 4.0*kappa_x1*kappa_y1*l1^2*m*sin(l1*(kappa_x1^2 + kappa_y1^2)^(1/2))*(kappa_x1^2 + kappa_y1^2) + 2.0*kappa_x1*kappa_y1^3*l1*m*r^2*cos(l1*(kappa_x1^2 + kappa_y1^2)^(1/2))*(kappa_x1^2 + kappa_y1^2)^(1/2) + 2.0*kappa_x1^3*kappa_y1*l1*m*r^2*cos(l1*(kappa_x1^2 + kappa_y1^2)^(1/2))*(kappa_x1^2 + kappa_y1^2)^(1/2) - 0.25*kappa_x1*kappa_y1^3*l1*m*r^2*cos(2.0*l1*(kappa_x1^2 + kappa_y1^2)^(1/2))*(kappa_x1^2 + kappa_y1^2)^(1/2) - 0.25*kappa_x1^3*kappa_y1*l1*m*r^2*cos(2.0*l1*(kappa_x1^2 + kappa_y1^2)^(1/2))*(kappa_x1^2 + kappa_y1^2)^(1/2)))/(2*l1^2*(kappa_x1^2 + kappa_y1^2)^(7/2)) + (dkappa_y1*(4.0*kappa_x1^2*m*sin(l1*(kappa_x1^2 + kappa_y1^2)^(1/2)) + 8.0*kappa_y1^2*m*sin(l1*(kappa_x1^2 + kappa_y1^2)^(1/2)) - 0.5*kappa_x1^2*m*sin(2.0*l1*(kappa_x1^2 + kappa_y1^2)^(1/2)) - 0.125*kappa_x1^4*m*r^2*sin(2.0*l1*(kappa_x1^2 + kappa_y1^2)^(1/2)) + 1.3333333333333333333333333333333*kappa_y1^2*l1^3*m*(kappa_x1^2 + kappa_y1^2)^(3/2) + 2.0*kappa_x1^4*m*r^2*sin(l1*(kappa_x1^2 + kappa_y1^2)^(1/2)) - 0.125*kappa_x1^2*kappa_y1^2*m*r^2*sin(2.0*l1*(kappa_x1^2 + kappa_y1^2)^(1/2)) + kappa_x1^2*l1*m*cos(2.0*l1*(kappa_x1^2 + kappa_y1^2)^(1/2))*(kappa_x1^2 + kappa_y1^2)^(1/2) + 0.33333333333333333333333333333333*kappa_y1^4*l1^3*m*r^2*(kappa_x1^2 + kappa_y1^2)^(3/2) + 2.0*kappa_x1^2*kappa_y1^2*m*r^2*sin(l1*(kappa_x1^2 + kappa_y1^2)^(1/2)) - 4.0*kappa_x1^2*l1*m*cos(l1*(kappa_x1^2 + kappa_y1^2)^(1/2))*(kappa_x1^2 + kappa_y1^2)^(1/2) - 8.0*kappa_y1^2*l1*m*cos(l1*(kappa_x1^2 + kappa_y1^2)^(1/2))*(kappa_x1^2 + kappa_y1^2)^(1/2) - 4.0*kappa_y1^2*l1^2*m*sin(l1*(kappa_x1^2 + kappa_y1^2)^(1/2))*(kappa_x1^2 + kappa_y1^2) + 0.33333333333333333333333333333333*kappa_x1^2*kappa_y1^2*l1^3*m*r^2*(kappa_x1^2 + kappa_y1^2)^(3/2) - 2.0*kappa_x1^4*l1*m*r^2*cos(l1*(kappa_x1^2 + kappa_y1^2)^(1/2))*(kappa_x1^2 + kappa_y1^2)^(1/2) + 0.25*kappa_x1^4*l1*m*r^2*cos(2.0*l1*(kappa_x1^2 + kappa_y1^2)^(1/2))*(kappa_x1^2 + kappa_y1^2)^(1/2) - 2.0*kappa_x1^2*kappa_y1^2*l1*m*r^2*cos(l1*(kappa_x1^2 + kappa_y1^2)^(1/2))*(kappa_x1^2 + kappa_y1^2)^(1/2) + 0.25*kappa_x1^2*kappa_y1^2*l1*m*r^2*cos(2.0*l1*(kappa_x1^2 + kappa_y1^2)^(1/2))*(kappa_x1^2 + kappa_y1^2)^(1/2)))/(2*l1^2*(kappa_x1^2 + kappa_y1^2)^(7/2)) + (dl1*(12.0*kappa_y1^3*l1^2*m*(kappa_x1^2 + kappa_y1^2)^(1/2) - 20.0*kappa_y1^3*l1*m*sin(l1*(kappa_x1^2 + kappa_y1^2)^(1/2)) - 4.0*kappa_y1*l1^2*m*(kappa_x1^2 + kappa_y1^2)^(3/2) - 12.0*kappa_y1*m*sin(l1*(kappa_x1^2 + kappa_y1^2)^(1/2))*(kappa_x1^2 + kappa_y1^2) - 20.0*kappa_x1^2*kappa_y1*l1*m*sin(l1*(kappa_x1^2 + kappa_y1^2)^(1/2)) + 12.0*kappa_x1^2*kappa_y1*l1^2*m*(kappa_x1^2 + kappa_y1^2)^(1/2) + 8.0*kappa_y1*l1*m*sin(l1*(kappa_x1^2 + kappa_y1^2)^(1/2))*(kappa_x1^2 + kappa_y1^2) + 4.0*kappa_y1^3*l1^2*m*cos(l1*(kappa_x1^2 + kappa_y1^2)^(1/2))*(kappa_x1^2 + kappa_y1^2)^(1/2) + 12.0*kappa_y1*l1*m*cos(l1*(kappa_x1^2 + kappa_y1^2)^(1/2))*(kappa_x1^2 + kappa_y1^2)^(3/2) + 4*kappa_y1*l1^2*m*sin(l1*(kappa_x1^2 + kappa_y1^2)^(1/2))*(kappa_x1^2 + kappa_y1^2)^2 + 4.0*kappa_x1^2*kappa_y1*l1^2*m*cos(l1*(kappa_x1^2 + kappa_y1^2)^(1/2))*(kappa_x1^2 + kappa_y1^2)^(1/2)))/(2*l1^2*(kappa_x1^2 + kappa_y1^2)^(7/2));
V(3,2) = (dkappa_x1*(1.5*kappa_y1^3*m*sin(2.0*l1*(kappa_x1^2 + kappa_y1^2)^(1/2)) - 28.0*kappa_y1^3*m*sin(l1*(kappa_x1^2 + kappa_y1^2)^(1/2)) + 0.125*kappa_y1^5*m*r^2*sin(2.0*l1*(kappa_x1^2 + kappa_y1^2)^(1/2)) + 1.3333333333333333333333333333333*kappa_y1*l1^3*m*(kappa_x1^2 + kappa_y1^2)^(5/2) + 5.0*kappa_x1^2*kappa_y1*m*sin(2.0*l1*(kappa_x1^2 + kappa_y1^2)^(1/2)) + 14.0*kappa_y1*l1*m*(kappa_x1^2 + kappa_y1^2)^(3/2) - 2.0*kappa_y1^5*m*r^2*sin(l1*(kappa_x1^2 + kappa_y1^2)^(1/2)) + 0.875*kappa_x1^2*kappa_y1^3*m*r^2*sin(2.0*l1*(kappa_x1^2 + kappa_y1^2)^(1/2)) - 1.0*kappa_y1^3*l1*m*cos(2.0*l1*(kappa_x1^2 + kappa_y1^2)^(1/2))*(kappa_x1^2 + kappa_y1^2)^(1/2) - 2.6666666666666666666666666666667*kappa_x1^2*kappa_y1*l1^3*m*(kappa_x1^2 + kappa_y1^2)^(3/2) + 4.5*kappa_y1^3*l1*m*r^2*(kappa_x1^2 + kappa_y1^2)^(3/2) + 1.5*kappa_y1^5*l1*m*r^2*(kappa_x1^2 + kappa_y1^2)^(1/2) - 4.0*kappa_x1^4*kappa_y1*l1^2*m*sin(l1*(kappa_x1^2 + kappa_y1^2)^(1/2)) - 12.0*kappa_x1^4*kappa_y1*m*r^2*sin(l1*(kappa_x1^2 + kappa_y1^2)^(1/2)) + 8.0*kappa_y1*l1*m*cos(l1*(kappa_x1^2 + kappa_y1^2)^(1/2))*(kappa_x1^2 + kappa_y1^2)^(3/2) + 0.33333333333333333333333333333333*kappa_y1^3*l1^3*m*r^2*(kappa_x1^2 + kappa_y1^2)^(5/2) + 0.75*kappa_x1^4*kappa_y1*m*r^2*sin(2.0*l1*(kappa_x1^2 + kappa_y1^2)^(1/2)) - 4.0*kappa_x1^2*kappa_y1^3*l1^2*m*sin(l1*(kappa_x1^2 + kappa_y1^2)^(1/2)) - 6.0*kappa_x1^2*kappa_y1*l1*m*(kappa_x1^2 + kappa_y1^2)^(1/2) - 14.0*kappa_x1^2*kappa_y1^3*m*r^2*sin(l1*(kappa_x1^2 + kappa_y1^2)^(1/2)) - 6.0*kappa_y1*l1*m*r^2*(kappa_x1^2 + kappa_y1^2)^(5/2) + 4.0*kappa_y1^3*l1*m*cos(l1*(kappa_x1^2 + kappa_y1^2)^(1/2))*(kappa_x1^2 + kappa_y1^2)^(1/2) - 24.0*kappa_x1^2*kappa_y1*l1*m*cos(l1*(kappa_x1^2 + kappa_y1^2)^(1/2))*(kappa_x1^2 + kappa_y1^2)^(1/2) - 0.66666666666666666666666666666667*kappa_x1^2*kappa_y1^3*l1^3*m*r^2*(kappa_x1^2 + kappa_y1^2)^(3/2) - 2.0*kappa_x1^2*kappa_y1*l1*m*cos(2.0*l1*(kappa_x1^2 + kappa_y1^2)^(1/2))*(kappa_x1^2 + kappa_y1^2)^(1/2) + 10.0*kappa_x1^2*kappa_y1*l1*m*r^2*(kappa_x1^2 + kappa_y1^2)^(3/2) + 3.0*kappa_x1^4*kappa_y1*l1*m*r^2*(kappa_x1^2 + kappa_y1^2)^(1/2) + 2.0*kappa_y1^5*l1*m*r^2*cos(l1*(kappa_x1^2 + kappa_y1^2)^(1/2))*(kappa_x1^2 + kappa_y1^2)^(1/2) - 0.25*kappa_y1^5*l1*m*r^2*cos(2.0*l1*(kappa_x1^2 + kappa_y1^2)^(1/2))*(kappa_x1^2 + kappa_y1^2)^(1/2) + 4.5*kappa_x1^2*kappa_y1^3*l1*m*r^2*(kappa_x1^2 + kappa_y1^2)^(1/2) + 0.66666666666666666666666666666667*kappa_x1^2*kappa_y1*l1^3*m*r^2*(kappa_x1^2 + kappa_y1^2)^(5/2) - 0.66666666666666666666666666666667*kappa_x1^4*kappa_y1*l1^3*m*r^2*(kappa_x1^2 + kappa_y1^2)^(3/2) + 4.0*kappa_x1^4*kappa_y1*l1*m*r^2*cos(l1*(kappa_x1^2 + kappa_y1^2)^(1/2))*(kappa_x1^2 + kappa_y1^2)^(1/2) - 0.5*kappa_x1^4*kappa_y1*l1*m*r^2*cos(2.0*l1*(kappa_x1^2 + kappa_y1^2)^(1/2))*(kappa_x1^2 + kappa_y1^2)^(1/2) + 6.0*kappa_x1^2*kappa_y1^3*l1*m*r^2*cos(l1*(kappa_x1^2 + kappa_y1^2)^(1/2))*(kappa_x1^2 + kappa_y1^2)^(1/2) - 0.75*kappa_x1^2*kappa_y1^3*l1*m*r^2*cos(2.0*l1*(kappa_x1^2 + kappa_y1^2)^(1/2))*(kappa_x1^2 + kappa_y1^2)^(1/2)))/(2*l1*(kappa_x1^2 + kappa_y1^2)^(9/2)) - (5.0e-34*dkappa_y1*(2.5e33*kappa_x1^3*m*sin(2.0*l1*(kappa_x1^2 + kappa_y1^2)^(1/2)) - 2.0e34*kappa_x1^3*m*sin(l1*(kappa_x1^2 + kappa_y1^2)^(1/2)) + 375000000000000000000000000000000.0*kappa_x1^5*m*r^2*sin(2.0*l1*(kappa_x1^2 + kappa_y1^2)^(1/2)) - 4.8e34*kappa_x1*kappa_y1^2*m*sin(l1*(kappa_x1^2 + kappa_y1^2)^(1/2)) - 1.0e33*kappa_x1*kappa_y1^2*m*sin(2.0*l1*(kappa_x1^2 + kappa_y1^2)^(1/2)) + 1.2e34*kappa_x1*l1*m*(kappa_x1^2 + kappa_y1^2)^(3/2) - 6.0e33*kappa_x1^5*m*r^2*sin(l1*(kappa_x1^2 + kappa_y1^2)^(1/2)) + 125000000000000000000000000000000.0*kappa_x1^3*kappa_y1^2*m*r^2*sin(2.0*l1*(kappa_x1^2 + kappa_y1^2)^(1/2)) - 1.0e33*kappa_x1^3*l1*m*cos(2.0*l1*(kappa_x1^2 + kappa_y1^2)^(1/2))*(kappa_x1^2 + kappa_y1^2)^(1/2) + 2.6666666666666666666666666666667e33*kappa_x1*kappa_y1^2*l1^3*m*(kappa_x1^2 + kappa_y1^2)^(3/2) + 5.0e33*kappa_x1^3*l1*m*r^2*(kappa_x1^2 + kappa_y1^2)^(3/2) + 1.5e33*kappa_x1^5*l1*m*r^2*(kappa_x1^2 + kappa_y1^2)^(1/2) + 4.0e33*kappa_x1*kappa_y1^4*l1^2*m*sin(l1*(kappa_x1^2 + kappa_y1^2)^(1/2)) + 4.0e33*kappa_x1*kappa_y1^4*m*r^2*sin(l1*(kappa_x1^2 + kappa_y1^2)^(1/2)) - 250000000000000000000000000000000.0*kappa_x1*kappa_y1^4*m*r^2*sin(2.0*l1*(kappa_x1^2 + kappa_y1^2)^(1/2)) + 4.0e33*kappa_x1^3*kappa_y1^2*l1^2*m*sin(l1*(kappa_x1^2 + kappa_y1^2)^(1/2)) + 6.0e33*kappa_x1*kappa_y1^2*l1*m*(kappa_x1^2 + kappa_y1^2)^(1/2) - 2.0e33*kappa_x1^3*kappa_y1^2*m*r^2*sin(l1*(kappa_x1^2 + kappa_y1^2)^(1/2)) - 3.0e33*kappa_x1*l1*m*r^2*(kappa_x1^2 + kappa_y1^2)^(5/2) + 4.0e33*kappa_x1^3*l1*m*cos(l1*(kappa_x1^2 + kappa_y1^2)^(1/2))*(kappa_x1^2 + kappa_y1^2)^(1/2) + 3.2e34*kappa_x1*kappa_y1^2*l1*m*cos(l1*(kappa_x1^2 + kappa_y1^2)^(1/2))*(kappa_x1^2 + kappa_y1^2)^(1/2) + 666666666666666666666666666666677.0*kappa_x1^3*kappa_y1^2*l1^3*m*r^2*(kappa_x1^2 + kappa_y1^2)^(3/2) - 500000000000000000000000000000000.0*kappa_x1*kappa_y1^2*l1*m*r^2*(kappa_x1^2 + kappa_y1^2)^(3/2) + 2.0e33*kappa_x1^5*l1*m*r^2*cos(l1*(kappa_x1^2 + kappa_y1^2)^(1/2))*(kappa_x1^2 + kappa_y1^2)^(1/2) - 250000000000000000000000000000000.0*kappa_x1^5*l1*m*r^2*cos(2.0*l1*(kappa_x1^2 + kappa_y1^2)^(1/2))*(kappa_x1^2 + kappa_y1^2)^(1/2) + 1.5e33*kappa_x1^3*kappa_y1^2*l1*m*r^2*(kappa_x1^2 + kappa_y1^2)^(1/2) - 333333333333333333333333333333333.0*kappa_x1*kappa_y1^2*l1^3*m*r^2*(kappa_x1^2 + kappa_y1^2)^(5/2) + 666666666666666666666666666666677.0*kappa_x1*kappa_y1^4*l1^3*m*r^2*(kappa_x1^2 + kappa_y1^2)^(3/2) + 2.0e33*kappa_x1^3*kappa_y1^2*l1*m*r^2*cos(l1*(kappa_x1^2 + kappa_y1^2)^(1/2))*(kappa_x1^2 + kappa_y1^2)^(1/2) - 250000000000000000000000000000000.0*kappa_x1^3*kappa_y1^2*l1*m*r^2*cos(2.0*l1*(kappa_x1^2 + kappa_y1^2)^(1/2))*(kappa_x1^2 + kappa_y1^2)^(1/2)))/(l1*(kappa_x1^2 + kappa_y1^2)^(9/2)) + (dl1*(4.0*kappa_x1*kappa_y1*m*sin(l1*(kappa_x1^2 + kappa_y1^2)^(1/2)) + 0.5*kappa_x1*kappa_y1*m*sin(2.0*l1*(kappa_x1^2 + kappa_y1^2)^(1/2)) - 2.0*kappa_x1*kappa_y1^3*m*r^2*sin(l1*(kappa_x1^2 + kappa_y1^2)^(1/2)) - 2.0*kappa_x1^3*kappa_y1*m*r^2*sin(l1*(kappa_x1^2 + kappa_y1^2)^(1/2)) + 0.125*kappa_x1*kappa_y1^3*m*r^2*sin(2.0*l1*(kappa_x1^2 + kappa_y1^2)^(1/2)) + 0.125*kappa_x1^3*kappa_y1*m*r^2*sin(2.0*l1*(kappa_x1^2 + kappa_y1^2)^(1/2)) + 1.3333333333333333333333333333333*kappa_x1*kappa_y1*l1^3*m*(kappa_x1^2 + kappa_y1^2)^(3/2) - 1.0*kappa_x1*kappa_y1*l1*m*cos(2.0*l1*(kappa_x1^2 + kappa_y1^2)^(1/2))*(kappa_x1^2 + kappa_y1^2)^(1/2) - 4.0*kappa_x1*kappa_y1*l1*m*cos(l1*(kappa_x1^2 + kappa_y1^2)^(1/2))*(kappa_x1^2 + kappa_y1^2)^(1/2) + 0.33333333333333333333333333333333*kappa_x1*kappa_y1^3*l1^3*m*r^2*(kappa_x1^2 + kappa_y1^2)^(3/2) + 0.33333333333333333333333333333333*kappa_x1^3*kappa_y1*l1^3*m*r^2*(kappa_x1^2 + kappa_y1^2)^(3/2) - 4.0*kappa_x1*kappa_y1*l1^2*m*sin(l1*(kappa_x1^2 + kappa_y1^2)^(1/2))*(kappa_x1^2 + kappa_y1^2) + 2.0*kappa_x1*kappa_y1^3*l1*m*r^2*cos(l1*(kappa_x1^2 + kappa_y1^2)^(1/2))*(kappa_x1^2 + kappa_y1^2)^(1/2) + 2.0*kappa_x1^3*kappa_y1*l1*m*r^2*cos(l1*(kappa_x1^2 + kappa_y1^2)^(1/2))*(kappa_x1^2 + kappa_y1^2)^(1/2) - 0.25*kappa_x1*kappa_y1^3*l1*m*r^2*cos(2.0*l1*(kappa_x1^2 + kappa_y1^2)^(1/2))*(kappa_x1^2 + kappa_y1^2)^(1/2) - 0.25*kappa_x1^3*kappa_y1*l1*m*r^2*cos(2.0*l1*(kappa_x1^2 + kappa_y1^2)^(1/2))*(kappa_x1^2 + kappa_y1^2)^(1/2)))/(2*l1^2*(kappa_x1^2 + kappa_y1^2)^(7/2));  
V(3,3) = (dl1*(4.0*kappa_x1^2*m*sin(l1*(kappa_x1^2 + kappa_y1^2)^(1/2)) + 8.0*kappa_y1^2*m*sin(l1*(kappa_x1^2 + kappa_y1^2)^(1/2)) - 0.5*kappa_x1^2*m*sin(2.0*l1*(kappa_x1^2 + kappa_y1^2)^(1/2)) - 0.125*kappa_x1^4*m*r^2*sin(2.0*l1*(kappa_x1^2 + kappa_y1^2)^(1/2)) + 1.3333333333333333333333333333333*kappa_y1^2*l1^3*m*(kappa_x1^2 + kappa_y1^2)^(3/2) + 2.0*kappa_x1^4*m*r^2*sin(l1*(kappa_x1^2 + kappa_y1^2)^(1/2)) - 0.125*kappa_x1^2*kappa_y1^2*m*r^2*sin(2.0*l1*(kappa_x1^2 + kappa_y1^2)^(1/2)) + kappa_x1^2*l1*m*cos(2.0*l1*(kappa_x1^2 + kappa_y1^2)^(1/2))*(kappa_x1^2 + kappa_y1^2)^(1/2) + 0.33333333333333333333333333333333*kappa_y1^4*l1^3*m*r^2*(kappa_x1^2 + kappa_y1^2)^(3/2) + 2.0*kappa_x1^2*kappa_y1^2*m*r^2*sin(l1*(kappa_x1^2 + kappa_y1^2)^(1/2)) - 4.0*kappa_x1^2*l1*m*cos(l1*(kappa_x1^2 + kappa_y1^2)^(1/2))*(kappa_x1^2 + kappa_y1^2)^(1/2) - 8.0*kappa_y1^2*l1*m*cos(l1*(kappa_x1^2 + kappa_y1^2)^(1/2))*(kappa_x1^2 + kappa_y1^2)^(1/2) - 4.0*kappa_y1^2*l1^2*m*sin(l1*(kappa_x1^2 + kappa_y1^2)^(1/2))*(kappa_x1^2 + kappa_y1^2) + 0.33333333333333333333333333333333*kappa_x1^2*kappa_y1^2*l1^3*m*r^2*(kappa_x1^2 + kappa_y1^2)^(3/2) - 2.0*kappa_x1^4*l1*m*r^2*cos(l1*(kappa_x1^2 + kappa_y1^2)^(1/2))*(kappa_x1^2 + kappa_y1^2)^(1/2) + 0.25*kappa_x1^4*l1*m*r^2*cos(2.0*l1*(kappa_x1^2 + kappa_y1^2)^(1/2))*(kappa_x1^2 + kappa_y1^2)^(1/2) - 2.0*kappa_x1^2*kappa_y1^2*l1*m*r^2*cos(l1*(kappa_x1^2 + kappa_y1^2)^(1/2))*(kappa_x1^2 + kappa_y1^2)^(1/2) + 0.25*kappa_x1^2*kappa_y1^2*l1*m*r^2*cos(2.0*l1*(kappa_x1^2 + kappa_y1^2)^(1/2))*(kappa_x1^2 + kappa_y1^2)^(1/2)))/(2*l1^2*(kappa_x1^2 + kappa_y1^2)^(7/2)) - (5.0e-34*dkappa_x1*(2.5e33*kappa_x1^3*m*sin(2.0*l1*(kappa_x1^2 + kappa_y1^2)^(1/2)) - 2.0e34*kappa_x1^3*m*sin(l1*(kappa_x1^2 + kappa_y1^2)^(1/2)) + 375000000000000000000000000000000.0*kappa_x1^5*m*r^2*sin(2.0*l1*(kappa_x1^2 + kappa_y1^2)^(1/2)) - 4.8e34*kappa_x1*kappa_y1^2*m*sin(l1*(kappa_x1^2 + kappa_y1^2)^(1/2)) - 1.0e33*kappa_x1*kappa_y1^2*m*sin(2.0*l1*(kappa_x1^2 + kappa_y1^2)^(1/2)) + 1.2e34*kappa_x1*l1*m*(kappa_x1^2 + kappa_y1^2)^(3/2) - 6.0e33*kappa_x1^5*m*r^2*sin(l1*(kappa_x1^2 + kappa_y1^2)^(1/2)) + 125000000000000000000000000000000.0*kappa_x1^3*kappa_y1^2*m*r^2*sin(2.0*l1*(kappa_x1^2 + kappa_y1^2)^(1/2)) - 1.0e33*kappa_x1^3*l1*m*cos(2.0*l1*(kappa_x1^2 + kappa_y1^2)^(1/2))*(kappa_x1^2 + kappa_y1^2)^(1/2) + 2.6666666666666666666666666666667e33*kappa_x1*kappa_y1^2*l1^3*m*(kappa_x1^2 + kappa_y1^2)^(3/2) + 5.0e33*kappa_x1^3*l1*m*r^2*(kappa_x1^2 + kappa_y1^2)^(3/2) + 1.5e33*kappa_x1^5*l1*m*r^2*(kappa_x1^2 + kappa_y1^2)^(1/2) + 4.0e33*kappa_x1*kappa_y1^4*l1^2*m*sin(l1*(kappa_x1^2 + kappa_y1^2)^(1/2)) + 4.0e33*kappa_x1*kappa_y1^4*m*r^2*sin(l1*(kappa_x1^2 + kappa_y1^2)^(1/2)) - 250000000000000000000000000000000.0*kappa_x1*kappa_y1^4*m*r^2*sin(2.0*l1*(kappa_x1^2 + kappa_y1^2)^(1/2)) + 4.0e33*kappa_x1^3*kappa_y1^2*l1^2*m*sin(l1*(kappa_x1^2 + kappa_y1^2)^(1/2)) + 6.0e33*kappa_x1*kappa_y1^2*l1*m*(kappa_x1^2 + kappa_y1^2)^(1/2) - 2.0e33*kappa_x1^3*kappa_y1^2*m*r^2*sin(l1*(kappa_x1^2 + kappa_y1^2)^(1/2)) - 3.0e33*kappa_x1*l1*m*r^2*(kappa_x1^2 + kappa_y1^2)^(5/2) + 4.0e33*kappa_x1^3*l1*m*cos(l1*(kappa_x1^2 + kappa_y1^2)^(1/2))*(kappa_x1^2 + kappa_y1^2)^(1/2) + 3.2e34*kappa_x1*kappa_y1^2*l1*m*cos(l1*(kappa_x1^2 + kappa_y1^2)^(1/2))*(kappa_x1^2 + kappa_y1^2)^(1/2) + 666666666666666666666666666666677.0*kappa_x1^3*kappa_y1^2*l1^3*m*r^2*(kappa_x1^2 + kappa_y1^2)^(3/2) - 500000000000000000000000000000000.0*kappa_x1*kappa_y1^2*l1*m*r^2*(kappa_x1^2 + kappa_y1^2)^(3/2) + 2.0e33*kappa_x1^5*l1*m*r^2*cos(l1*(kappa_x1^2 + kappa_y1^2)^(1/2))*(kappa_x1^2 + kappa_y1^2)^(1/2) - 250000000000000000000000000000000.0*kappa_x1^5*l1*m*r^2*cos(2.0*l1*(kappa_x1^2 + kappa_y1^2)^(1/2))*(kappa_x1^2 + kappa_y1^2)^(1/2) + 1.5e33*kappa_x1^3*kappa_y1^2*l1*m*r^2*(kappa_x1^2 + kappa_y1^2)^(1/2) - 333333333333333333333333333333333.0*kappa_x1*kappa_y1^2*l1^3*m*r^2*(kappa_x1^2 + kappa_y1^2)^(5/2) + 666666666666666666666666666666677.0*kappa_x1*kappa_y1^4*l1^3*m*r^2*(kappa_x1^2 + kappa_y1^2)^(3/2) + 2.0e33*kappa_x1^3*kappa_y1^2*l1*m*r^2*cos(l1*(kappa_x1^2 + kappa_y1^2)^(1/2))*(kappa_x1^2 + kappa_y1^2)^(1/2) - 250000000000000000000000000000000.0*kappa_x1^3*kappa_y1^2*l1*m*r^2*cos(2.0*l1*(kappa_x1^2 + kappa_y1^2)^(1/2))*(kappa_x1^2 + kappa_y1^2)^(1/2)))/(l1*(kappa_x1^2 + kappa_y1^2)^(9/2)) - (5.0e-34*dkappa_y1*(6.0e33*kappa_y1^3*l1*m*(kappa_x1^2 + kappa_y1^2)^(1/2) - 4.0e34*kappa_y1^3*m*sin(l1*(kappa_x1^2 + kappa_y1^2)^(1/2)) - 1.3333333333333333333333333333333e33*kappa_y1*l1^3*m*(kappa_x1^2 + kappa_y1^2)^(5/2) - 1.2e34*kappa_x1^2*kappa_y1*m*sin(l1*(kappa_x1^2 + kappa_y1^2)^(1/2)) + 2.6666666666666666666666666666667e33*kappa_y1^3*l1^3*m*(kappa_x1^2 + kappa_y1^2)^(3/2) + 3.5e33*kappa_x1^2*kappa_y1*m*sin(2.0*l1*(kappa_x1^2 + kappa_y1^2)^(1/2)) + 4.0e33*kappa_y1^5*l1^2*m*sin(l1*(kappa_x1^2 + kappa_y1^2)^(1/2)) + 1.0e34*kappa_y1*l1*m*(kappa_x1^2 + kappa_y1^2)^(3/2) + 625000000000000000000000000000000.0*kappa_x1^2*kappa_y1^3*m*r^2*sin(2.0*l1*(kappa_x1^2 + kappa_y1^2)^(1/2)) - 1.0e34*kappa_x1^4*kappa_y1*m*r^2*sin(l1*(kappa_x1^2 + kappa_y1^2)^(1/2)) - 8.0e33*kappa_y1*l1*m*cos(l1*(kappa_x1^2 + kappa_y1^2)^(1/2))*(kappa_x1^2 + kappa_y1^2)^(3/2) - 666666666666666666666666666666677.0*kappa_y1^3*l1^3*m*r^2*(kappa_x1^2 + kappa_y1^2)^(5/2) + 666666666666666666666666666666677.0*kappa_y1^5*l1^3*m*r^2*(kappa_x1^2 + kappa_y1^2)^(3/2) + 625000000000000000000000000000000.0*kappa_x1^4*kappa_y1*m*r^2*sin(2.0*l1*(kappa_x1^2 + kappa_y1^2)^(1/2)) + 4.0e33*kappa_x1^2*kappa_y1^3*l1^2*m*sin(l1*(kappa_x1^2 + kappa_y1^2)^(1/2)) - 1.0e34*kappa_x1^2*kappa_y1^3*m*r^2*sin(l1*(kappa_x1^2 + kappa_y1^2)^(1/2)) + 3.2e34*kappa_y1^3*l1*m*cos(l1*(kappa_x1^2 + kappa_y1^2)^(1/2))*(kappa_x1^2 + kappa_y1^2)^(1/2) + 4.0e33*kappa_x1^2*kappa_y1*l1*m*cos(l1*(kappa_x1^2 + kappa_y1^2)^(1/2))*(kappa_x1^2 + kappa_y1^2)^(1/2) + 666666666666666666666666666666677.0*kappa_x1^2*kappa_y1^3*l1^3*m*r^2*(kappa_x1^2 + kappa_y1^2)^(3/2) - 1.0e33*kappa_x1^2*kappa_y1*l1*m*cos(2.0*l1*(kappa_x1^2 + kappa_y1^2)^(1/2))*(kappa_x1^2 + kappa_y1^2)^(1/2) + 5.5e33*kappa_x1^2*kappa_y1*l1*m*r^2*(kappa_x1^2 + kappa_y1^2)^(3/2) + 1.5e33*kappa_x1^4*kappa_y1*l1*m*r^2*(kappa_x1^2 + kappa_y1^2)^(1/2) + 1.5e33*kappa_x1^2*kappa_y1^3*l1*m*r^2*(kappa_x1^2 + kappa_y1^2)^(1/2) - 333333333333333333333333333333333.0*kappa_x1^2*kappa_y1*l1^3*m*r^2*(kappa_x1^2 + kappa_y1^2)^(5/2) + 2.0e33*kappa_x1^4*kappa_y1*l1*m*r^2*cos(l1*(kappa_x1^2 + kappa_y1^2)^(1/2))*(kappa_x1^2 + kappa_y1^2)^(1/2) - 250000000000000000000000000000000.0*kappa_x1^4*kappa_y1*l1*m*r^2*cos(2.0*l1*(kappa_x1^2 + kappa_y1^2)^(1/2))*(kappa_x1^2 + kappa_y1^2)^(1/2) + 2.0e33*kappa_x1^2*kappa_y1^3*l1*m*r^2*cos(l1*(kappa_x1^2 + kappa_y1^2)^(1/2))*(kappa_x1^2 + kappa_y1^2)^(1/2) - 250000000000000000000000000000000.0*kappa_x1^2*kappa_y1^3*l1*m*r^2*cos(2.0*l1*(kappa_x1^2 + kappa_y1^2)^(1/2))*(kappa_x1^2 + kappa_y1^2)^(1/2)))/(l1*(kappa_x1^2 + kappa_y1^2)^(9/2));


y = V;
